simulink model "kinovaMicoSimscapeModel"  (R2021b)
(part 36 of 50)

Y1_10_7=(7*3^(1/2)*dq6*dqr2*cos(q2)*cos(q3)*sin(q6))/4000 + (29*3^(1/2)*dq1*dqr2*sin(2*q2)*cos(q3)*cos(q6))/400 + dq1*dqr2*cos(2*q2)*sin(2*q3)*cos(q6)*((6847*3^(1/2))/160000 - 481/32000) - dq1*dqr2*cos(2*q3)*sin(2*q2)*cos(q6)*((6847*3^(1/2))/160000 - 481/32000) - (333*dq1*dqr2*cos(2*q2)*cos(2*q5)*sin(2*q3)*cos(q6))/32000 + (333*dq1*dqr2*cos(2*q3)*cos(2*q5)*sin(2*q2)*cos(q6))/32000 + (21*dq2*dqr3*cos(q6)*sin(q2)*sin(q3)*sin(q4))/4000 - (21*dq3*dqr3*cos(q6)*sin(q2)*sin(q3)*sin(q4))/4000 + (333*dq1*dqr2*cos(2*q2)*sin(2*q3)*sin(2*q5)*sin(q6))/16000 - (333*dq1*dqr2*cos(2*q3)*sin(2*q2)*sin(2*q5)*sin(q6))/16000 + dq2*dqr2*sin(2*q4)*cos(q2)*cos(q3)*cos(q6)*((1923*3^(1/2))/80000 + 111/3200) - dq3*dqr2*sin(2*q4)*cos(q2)*cos(q3)*cos(q6)*((1923*3^(1/2))/80000 + 111/3200) - (37*3^(1/2)*dq5*dqr3*cos(q6)*sin(q2)*sin(q3)*sin(q4))/4000 + (7*3^(1/2)*dq5*dqr3*cos(q6)*sin(q2)*sin(q3)*sin(q5))/4000 - (37*3^(1/2)*dq6*dqr3*cos(q6)*sin(q2)*sin(q3)*sin(q4))/4000 + (7*3^(1/2)*dq6*dqr3*cos(q6)*sin(q2)*sin(q3)*sin(q5))/2000 + (877*dq1*dqr2*cos(2*q2)*cos(2*q3)*cos(q4)*cos(q5)*sin(q6))/4000 - (37*dq2*dqr2*cos(2*q4)*cos(2*q5)*cos(q2)*cos(q3)*sin(q6))/2000 - (37*dq2*dqr2*cos(2*q4)*sin(2*q5)*cos(q2)*cos(q3)*cos(q6))/4000 - (37*dq2*dqr2*cos(2*q5)*sin(2*q4)*cos(q2)*cos(q3)*cos(q6))/3200 + (37*dq3*dqr2*cos(2*q4)*cos(2*q5)*cos(q2)*cos(q3)*sin(q6))/2000 + (37*dq3*dqr2*cos(2*q4)*sin(2*q5)*cos(q2)*cos(q3)*cos(q6))/4000 + (37*dq3*dqr2*cos(2*q5)*sin(2*q4)*cos(q2)*cos(q3)*cos(q6))/3200 + (877*dq1*dqr2*sin(2*q2)*sin(2*q3)*cos(q4)*cos(q5)*sin(q6))/4000 + (37*dq2*dqr2*sin(2*q4)*sin(2*q5)*cos(q2)*cos(q3)*sin(q6))/1600 - (37*dq3*dqr2*sin(2*q4)*sin(2*q5)*cos(q2)*cos(q3)*sin(q6))/1600 - (29*3^(1/2)*dq1*dqr2*sin(2*q2)*cos(q3)*cos(q5)*cos(q6))/400 - (7*dq2*dqr2*cos(q2)*cos(q3)*cos(q4)*cos(q5)*sin(q6))/1000 - (7*dq2*dqr2*cos(q2)*cos(q3)*cos(q4)*cos(q6)*sin(q5))/2000 + (7*dq3*dqr2*cos(q2)*cos(q3)*cos(q4)*cos(q5)*sin(q6))/1000 + (7*dq3*dqr2*cos(q2)*cos(q3)*cos(q4)*cos(q6)*sin(q5))/2000 - dq1*dqr2*cos(2*q2)*sin(2*q3)*cos(q5)*cos(q6)*((9411*3^(1/2))/160000 - 259/16000) + dq1*dqr2*cos(2*q3)*sin(2*q2)*cos(q5)*cos(q6)*((9411*3^(1/2))/160000 - 259/16000) + (29*3^(1/2)*dq1*dqr2*sin(2*q2)*cos(q3)*sin(q5)*sin(q6))/200 + (7*dq2*dqr3*cos(q4)*cos(q5)*sin(q2)*sin(q3)*sin(q6))/1000 + (7*dq2*dqr3*cos(q4)*cos(q6)*sin(q2)*sin(q3)*sin(q5))/2000 + (7*dq2*dqr3*cos(q5)*cos(q6)*sin(q2)*sin(q3)*sin(q4))/4000 - (7*dq3*dqr3*cos(q4)*cos(q5)*sin(q2)*sin(q3)*sin(q6))/1000 - (7*dq3*dqr3*cos(q4)*cos(q6)*sin(q2)*sin(q3)*sin(q5))/2000 - (7*dq3*dqr3*cos(q5)*cos(q6)*sin(q2)*sin(q3)*sin(q4))/4000 + dq1*dqr2*cos(2*q2)*sin(2*q3)*sin(q5)*sin(q6)*((9411*3^(1/2))/80000 + 37/4000) - dq1*dqr2*cos(2*q3)*sin(2*q2)*sin(q5)*sin(q6)*((9411*3^(1/2))/80000 + 37/4000) - (7*dq2*dqr3*sin(q2)*sin(q3)*sin(q4)*sin(q5)*sin(q6))/2000 + (7*dq3*dqr3*sin(q2)*sin(q3)*sin(q4)*sin(q5)*sin(q6))/2000 - dq6*dqr2*cos(q2)*cos(q3)*cos(q4)*sin(q6)*((37*3^(1/2))/3200 + 1923/80000) - (29*dq1*dqr2*cos(2*q2)*cos(q3)*cos(q4)*cos(q5)*sin(q6))/100 - (29*dq1*dqr2*cos(2*q2)*cos(q3)*cos(q4)*cos(q6)*sin(q5))/200 + dq1*dqr2*cos(2*q2)*cos(2*q4)*sin(2*q3)*cos(q6)*((1923*3^(1/2))/160000 + 111/6400) - dq1*dqr2*cos(2*q3)*cos(2*q4)*sin(2*q2)*cos(q6)*((1923*3^(1/2))/160000 + 111/6400) - (37*dq1*dqr2*cos(2*q2)*cos(2*q4)*cos(2*q5)*sin(2*q3)*cos(q6))/6400 + (37*dq1*dqr2*cos(2*q3)*cos(2*q4)*cos(2*q5)*sin(2*q2)*cos(q6))/6400 - (7*3^(1/2)*dq5*dqr2*cos(q2)*cos(q3)*cos(q5)*sin(q6))/2000 - (7*3^(1/2)*dq5*dqr2*cos(q2)*cos(q3)*cos(q6)*sin(q5))/4000 - (7*3^(1/2)*dq6*dqr2*cos(q2)*cos(q3)*cos(q5)*sin(q6))/4000 - (7*3^(1/2)*dq6*dqr2*cos(q2)*cos(q3)*cos(q6)*sin(q5))/2000 + (37*dq1*dqr2*cos(2*q2)*cos(2*q4)*sin(2*q3)*sin(2*q5)*sin(q6))/3200 + (37*dq1*dqr2*cos(2*q2)*cos(2*q5)*sin(2*q3)*sin(2*q4)*sin(q6))/4000 + (37*dq1*dqr2*cos(2*q2)*sin(2*q3)*sin(2*q4)*sin(2*q5)*cos(q6))/8000 - (37*dq1*dqr2*cos(2*q3)*cos(2*q4)*sin(2*q2)*sin(2*q5)*sin(q6))/3200 - (37*dq1*dqr2*cos(2*q3)*cos(2*q5)*sin(2*q2)*sin(2*q4)*sin(q6))/4000 - (37*dq1*dqr2*cos(2*q3)*sin(2*q2)*sin(2*q4)*sin(2*q5)*cos(q6))/8000 + dq2*dqr3*sin(2*q4)*sin(q2)*sin(q3)*sin(q5)*sin(q6)*((641*3^(1/2))/40000 + 37/2000) - dq3*dqr3*sin(2*q4)*sin(q2)*sin(q3)*sin(q5)*sin(q6)*((641*3^(1/2))/40000 + 37/2000) - (37*3^(1/2)*dq5*dqr2*cos(2*q5)*cos(q2)*cos(q3)*cos(q4)*sin(q6))/4000 - (37*3^(1/2)*dq5*dqr2*sin(2*q5)*cos(q2)*cos(q3)*cos(q4)*cos(q6))/8000 - (37*3^(1/2)*dq6*dqr2*cos(2*q5)*cos(q2)*cos(q3)*cos(q4)*sin(q6))/16000 - (37*3^(1/2)*dq6*dqr2*sin(2*q5)*cos(q2)*cos(q3)*cos(q4)*cos(q6))/8000 - dq1*dqr2*cos(2*q2)*cos(2*q3)*cos(q4)*cos(q6)*sin(q5)*((37*3^(1/2))/4000 - 877/8000) + (37*3^(1/2)*dq5*dqr3*cos(2*q5)*cos(q6)*sin(q2)*sin(q3)*sin(q4))/4000 + (37*3^(1/2)*dq6*dqr3*cos(2*q5)*cos(q6)*sin(q2)*sin(q3)*sin(q4))/4000 - dq1*dqr2*sin(2*q2)*sin(2*q3)*cos(q4)*cos(q6)*sin(q5)*((37*3^(1/2))/4000 - 877/8000) - (37*3^(1/2)*dq5*dqr3*sin(2*q5)*sin(q2)*sin(q3)*sin(q4)*sin(q6))/2000 - (37*3^(1/2)*dq6*dqr3*sin(2*q5)*sin(q2)*sin(q3)*sin(q4)*sin(q6))/8000 + dq5*dqr2*cos(q2)*cos(q3)*cos(q4)*cos(q5)*sin(q6)*((37*3^(1/2))/2000 + 1923/40000) + dq6*dqr2*cos(q2)*cos(q3)*cos(q4)*cos(q6)*sin(q5)*((37*3^(1/2))/2000 + 1923/40000) - dq5*dqr2*cos(q2)*cos(q3)*cos(q4)*cos(q6)*sin(q5)*((37*3^(1/2))/8000 - 1923/80000) + dq6*dqr2*cos(q2)*cos(q3)*cos(q4)*cos(q5)*sin(q6)*((111*3^(1/2))/8000 + 1923/80000) + dq1*dqr2*cos(2*q2)*cos(2*q4)*sin(2*q3)*cos(q5)*cos(q6)*((641*3^(1/2))/160000 - 37/16000) - dq1*dqr2*cos(2*q3)*cos(2*q4)*sin(2*q2)*cos(q5)*cos(q6)*((641*3^(1/2))/160000 - 37/16000) - dq6*dqr3*cos(q4)*cos(q6)*sin(q2)*sin(q3)*sin(q5)*((37*3^(1/2))/2000 + 1923/40000) + dq5*dqr3*cos(q4)*cos(q6)*sin(q2)*sin(q3)*sin(q5)*((37*3^(1/2))/8000 - 1923/80000) - dq1*dqr2*cos(2*q2)*sin(2*q3)*sin(2*q4)*cos(q5)*sin(q6)*((641*3^(1/2))/40000 + 37/2000) + dq1*dqr2*cos(2*q3)*sin(2*q2)*sin(2*q4)*cos(q5)*sin(q6)*((641*3^(1/2))/40000 + 37/2000) - dq1*dqr2*cos(2*q2)*cos(2*q4)*sin(2*q3)*sin(q5)*sin(q6)*((641*3^(1/2))/80000 + 37/4000) + dq1*dqr2*cos(2*q3)*cos(2*q4)*sin(2*q2)*sin(q5)*sin(q6)*((641*3^(1/2))/80000 + 37/4000) - dq1*dqr2*cos(2*q2)*sin(2*q3)*sin(2*q4)*cos(q6)*sin(q5)*((641*3^(1/2))/80000 - 37/8000) + dq1*dqr2*cos(2*q3)*sin(2*q2)*sin(2*q4)*cos(q6)*sin(q5)*((641*3^(1/2))/80000 - 37/8000) + (37*3^(1/2)*dq1*dqr2*cos(2*q2)*cos(2*q3)*cos(2*q5)*cos(q4)*sin(q6))/2000 + (37*3^(1/2)*dq1*dqr2*cos(2*q2)*cos(2*q3)*sin(2*q5)*cos(q4)*cos(q6))/4000 + dq2*dqr2*cos(2*q4)*cos(q2)*cos(q3)*cos(q5)*sin(q6)*((641*3^(1/2))/20000 + 37/1000) - dq3*dqr2*cos(2*q4)*cos(q2)*cos(q3)*cos(q5)*sin(q6)*((641*3^(1/2))/20000 + 37/1000) + dq2*dqr2*cos(2*q4)*cos(q2)*cos(q3)*cos(q6)*sin(q5)*((641*3^(1/2))/40000 - 37/4000) - dq3*dqr2*cos(2*q4)*cos(q2)*cos(q3)*cos(q6)*sin(q5)*((641*3^(1/2))/40000 - 37/4000) + dq2*dqr2*sin(2*q4)*cos(q2)*cos(q3)*cos(q5)*cos(q6)*((641*3^(1/2))/80000 - 37/8000) - dq3*dqr2*sin(2*q4)*cos(q2)*cos(q3)*cos(q5)*cos(q6)*((641*3^(1/2))/80000 - 37/8000) + (37*3^(1/2)*dq1*dqr2*cos(2*q5)*sin(2*q2)*sin(2*q3)*cos(q4)*sin(q6))/2000 + (37*3^(1/2)*dq1*dqr2*sin(2*q2)*sin(2*q3)*sin(2*q5)*cos(q4)*cos(q6))/4000 - dq2*dqr3*cos(2*q4)*cos(q6)*sin(q2)*sin(q3)*sin(q5)*((641*3^(1/2))/40000 - 37/4000) + dq3*dqr3*cos(2*q4)*cos(q6)*sin(q2)*sin(q3)*sin(q5)*((641*3^(1/2))/40000 - 37/4000) + (37*3^(1/2)*dq6*dqr3*sin(q2)*sin(q3)*sin(q4)*sin(q5)*sin(q6))/4000;
Y1_10_8=(37*dq5*dqr3*cos(q3)*cos(q6)*sin(q2))/4000 + (37*dq6*dqr3*cos(q3)*cos(q6)*sin(q2))/4000 + (111*dq4*dqr3*sin(2*q5)*cos(q3)*sin(q2)*sin(q6))/8000 - (7*3^(1/2)*dq2*dqr3*cos(q3)*cos(q6)*sin(q2))/4000 + (7*3^(1/2)*dq3*dqr3*cos(q3)*cos(q6)*sin(q2))/4000 - (7*3^(1/2)*dq6*dqr3*sin(q2)*sin(q3)*sin(q6))/4000 + (21*dq4*dqr3*cos(q3)*cos(q4)*cos(q6)*sin(q2))/4000 - (21*dq6*dqr3*cos(q3)*sin(q2)*sin(q4)*sin(q6))/4000 - dq4*dqr3*cos(q3)*cos(q6)*sin(q2)*((1923*3^(1/2))/80000 + 259/16000) - (111*dq4*dqr3*cos(2*q5)*cos(q3)*cos(q6)*sin(q2))/16000 - dq4*dqr3*cos(2*q4)*cos(q3)*cos(q6)*sin(q2)*((1923*3^(1/2))/80000 + 111/3200) - (7*3^(1/2)*dq2*dqr3*cos(q3)*sin(q2)*sin(q5)*sin(q6))/2000 + (7*3^(1/2)*dq3*dqr3*cos(q3)*sin(q2)*sin(q5)*sin(q6))/2000 + (7*3^(1/2)*dq5*dqr3*cos(q5)*sin(q2)*sin(q3)*sin(q6))/2000 + (7*3^(1/2)*dq6*dqr3*cos(q5)*sin(q2)*sin(q3)*sin(q6))/4000 + (37*dq4*dqr3*cos(2*q4)*cos(2*q5)*cos(q3)*cos(q6)*sin(q2))/3200 + (37*dq5*dqr3*cos(2*q4)*cos(2*q5)*cos(q3)*cos(q6)*sin(q2))/4000 + (37*dq6*dqr3*cos(2*q4)*cos(2*q5)*cos(q3)*cos(q6)*sin(q2))/4000 - dq2*dqr3*sin(2*q4)*cos(q6)*sin(q2)*sin(q3)*((1923*3^(1/2))/80000 + 111/3200) + dq3*dqr3*sin(2*q4)*cos(q6)*sin(q2)*sin(q3)*((1923*3^(1/2))/80000 + 111/3200) + dq6*dqr3*sin(2*q4)*cos(q3)*sin(q2)*sin(q6)*((1923*3^(1/2))/160000 + 111/6400) + (37*dq2*dqr3*cos(2*q4)*cos(2*q5)*sin(q2)*sin(q3)*sin(q6))/2000 + (37*dq2*dqr3*cos(2*q4)*sin(2*q5)*cos(q6)*sin(q2)*sin(q3))/4000 + (37*dq2*dqr3*cos(2*q5)*sin(2*q4)*cos(q6)*sin(q2)*sin(q3))/3200 - (37*dq3*dqr3*cos(2*q4)*cos(2*q5)*sin(q2)*sin(q3)*sin(q6))/2000 - (37*dq3*dqr3*cos(2*q4)*sin(2*q5)*cos(q6)*sin(q2)*sin(q3))/4000 - (37*dq3*dqr3*cos(2*q5)*sin(2*q4)*cos(q6)*sin(q2)*sin(q3))/3200 - (37*dq4*dqr3*cos(2*q4)*sin(2*q5)*cos(q3)*sin(q2)*sin(q6))/1600 - (37*dq4*dqr3*cos(2*q5)*sin(2*q4)*cos(q3)*sin(q2)*sin(q6))/2000 - (37*dq4*dqr3*sin(2*q4)*sin(2*q5)*cos(q3)*cos(q6)*sin(q2))/4000 - (37*dq5*dqr3*cos(2*q4)*sin(2*q5)*cos(q3)*sin(q2)*sin(q6))/2000 - (37*dq5*dqr3*cos(2*q5)*sin(2*q4)*cos(q3)*sin(q2)*sin(q6))/1600 - (37*dq5*dqr3*sin(2*q4)*sin(2*q5)*cos(q3)*cos(q6)*sin(q2))/3200 - (37*dq6*dqr3*cos(2*q4)*sin(2*q5)*cos(q3)*sin(q2)*sin(q6))/8000 - (37*dq6*dqr3*cos(2*q5)*sin(2*q4)*cos(q3)*sin(q2)*sin(q6))/6400 - (37*dq6*dqr3*sin(2*q4)*sin(2*q5)*cos(q3)*cos(q6)*sin(q2))/3200 - (37*dq2*dqr3*sin(2*q4)*sin(2*q5)*sin(q2)*sin(q3)*sin(q6))/1600 + (37*dq3*dqr3*sin(2*q4)*sin(2*q5)*sin(q2)*sin(q3)*sin(q6))/1600 + (1231*dq2*dqr3*cos(q3)*cos(q4)*cos(q5)*cos(q6)*sin(q2))/40000 - (1231*dq3*dqr3*cos(q3)*cos(q4)*cos(q5)*cos(q6)*sin(q2))/40000 + (7*dq4*dqr3*cos(q3)*cos(q4)*cos(q5)*cos(q6)*sin(q2))/4000 + (7*dq5*dqr3*cos(q3)*cos(q4)*cos(q5)*cos(q6)*sin(q2))/2000 + (7*dq6*dqr3*cos(q3)*cos(q4)*cos(q5)*cos(q6)*sin(q2))/1000 - (877*dq2*dqr3*cos(q3)*cos(q5)*sin(q2)*sin(q4)*sin(q6))/4000 + (877*dq3*dqr3*cos(q3)*cos(q5)*sin(q2)*sin(q4)*sin(q6))/4000 - (7*dq4*dqr3*cos(q3)*cos(q4)*sin(q2)*sin(q5)*sin(q6))/2000 - (7*dq4*dqr3*cos(q3)*cos(q5)*sin(q2)*sin(q4)*sin(q6))/1000 - (7*dq4*dqr3*cos(q3)*cos(q6)*sin(q2)*sin(q4)*sin(q5))/2000 - (7*dq5*dqr3*cos(q3)*cos(q4)*sin(q2)*sin(q5)*sin(q6))/1000 - (7*dq5*dqr3*cos(q3)*cos(q5)*sin(q2)*sin(q4)*sin(q6))/2000 - (7*dq5*dqr3*cos(q3)*cos(q6)*sin(q2)*sin(q4)*sin(q5))/4000 - (7*dq6*dqr3*cos(q3)*cos(q4)*sin(q2)*sin(q5)*sin(q6))/2000 - (7*dq6*dqr3*cos(q3)*cos(q5)*sin(q2)*sin(q4)*sin(q6))/4000 - (7*dq6*dqr3*cos(q3)*cos(q6)*sin(q2)*sin(q4)*sin(q5))/2000 - dq6*dqr3*cos(q3)*cos(q5)*cos(q6)*sin(q2)*((641*3^(1/2))/40000 + 37/2000) + dq2*dqr3*cos(q3)*cos(q4)*cos(q6)*sin(q2)*((111*3^(1/2))/8000 + 7539/40000) - dq3*dqr3*cos(q3)*cos(q4)*cos(q6)*sin(q2)*((111*3^(1/2))/8000 + 7539/40000) - dq4*dqr3*cos(q3)*cos(q5)*cos(q6)*sin(q2)*((641*3^(1/2))/80000 - 37/8000) - dq5*dqr3*cos(q3)*cos(q5)*cos(q6)*sin(q2)*((641*3^(1/2))/80000 - 37/8000) + dq4*dqr3*cos(q3)*sin(q2)*sin(q5)*sin(q6)*((641*3^(1/2))/40000 + 37/2000) + dq5*dqr3*cos(q3)*sin(q2)*sin(q5)*sin(q6)*((641*3^(1/2))/40000 + 37/2000) + dq6*dqr3*cos(q3)*sin(q2)*sin(q5)*sin(q6)*((641*3^(1/2))/80000 + 37/1600) + dq6*dqr3*cos(q4)*sin(q2)*sin(q3)*sin(q6)*((37*3^(1/2))/3200 + 1923/80000) + (7*3^(1/2)*dq2*dqr3*cos(q3)*cos(q5)*cos(q6)*sin(q2))/4000 - (7*3^(1/2)*dq3*dqr3*cos(q3)*cos(q5)*cos(q6)*sin(q2))/4000 - (29*dq1*dqr3*sin(2*q2)*sin(q3)*sin(q4)*sin(q5)*sin(q6))/400 + (37*3^(1/2)*dq2*dqr3*cos(2*q5)*cos(q3)*cos(q4)*cos(q6)*sin(q2))/8000 - (37*3^(1/2)*dq3*dqr3*cos(2*q5)*cos(q3)*cos(q4)*cos(q6)*sin(q2))/8000 - (37*3^(1/2)*dq2*dqr3*cos(2*q5)*cos(q3)*sin(q2)*sin(q4)*sin(q6))/2000 - (37*3^(1/2)*dq2*dqr3*sin(2*q5)*cos(q3)*cos(q4)*sin(q2)*sin(q6))/4000 - (37*3^(1/2)*dq2*dqr3*sin(2*q5)*cos(q3)*cos(q6)*sin(q2)*sin(q4))/4000 + (37*3^(1/2)*dq3*dqr3*cos(2*q5)*cos(q3)*sin(q2)*sin(q4)*sin(q6))/2000 + (37*3^(1/2)*dq3*dqr3*sin(2*q5)*cos(q3)*cos(q4)*sin(q2)*sin(q6))/4000 + (37*3^(1/2)*dq3*dqr3*sin(2*q5)*cos(q3)*cos(q6)*sin(q2)*sin(q4))/4000 + (37*3^(1/2)*dq5*dqr3*cos(2*q5)*cos(q4)*sin(q2)*sin(q3)*sin(q6))/4000 + (37*3^(1/2)*dq5*dqr3*sin(2*q5)*cos(q4)*cos(q6)*sin(q2)*sin(q3))/8000 + (37*3^(1/2)*dq6*dqr3*cos(2*q5)*cos(q4)*sin(q2)*sin(q3)*sin(q6))/16000 + (37*3^(1/2)*dq6*dqr3*sin(2*q5)*cos(q4)*cos(q6)*sin(q2)*sin(q3))/8000 + dq2*dqr3*cos(q3)*cos(q6)*sin(q2)*sin(q4)*sin(q5)*((37*3^(1/2))/4000 - 877/8000) - dq3*dqr3*cos(q3)*cos(q6)*sin(q2)*sin(q4)*sin(q5)*((37*3^(1/2))/4000 - 877/8000) + dq2*dqr3*cos(q3)*cos(q4)*sin(q2)*sin(q5)*sin(q6)*((37*3^(1/2))/2000 - 1231/20000) - dq3*dqr3*cos(q3)*cos(q4)*sin(q2)*sin(q5)*sin(q6)*((37*3^(1/2))/2000 - 1231/20000) - dq5*dqr3*cos(q4)*cos(q5)*sin(q2)*sin(q3)*sin(q6)*((37*3^(1/2))/2000 + 1923/40000) - dq6*dqr3*cos(q4)*cos(q5)*sin(q2)*sin(q3)*sin(q6)*((111*3^(1/2))/8000 + 1923/80000) - dq6*dqr3*cos(2*q4)*cos(q3)*cos(q5)*cos(q6)*sin(q2)*((641*3^(1/2))/40000 + 37/2000) - dq4*dqr3*cos(2*q4)*cos(q3)*cos(q5)*cos(q6)*sin(q2)*((641*3^(1/2))/80000 - 37/8000) - dq5*dqr3*cos(2*q4)*cos(q3)*cos(q5)*cos(q6)*sin(q2)*((641*3^(1/2))/80000 - 37/8000) - dq2*dqr3*cos(2*q4)*cos(q5)*sin(q2)*sin(q3)*sin(q6)*((641*3^(1/2))/20000 + 37/1000) + dq3*dqr3*cos(2*q4)*cos(q5)*sin(q2)*sin(q3)*sin(q6)*((641*3^(1/2))/20000 + 37/1000) + dq4*dqr3*sin(2*q4)*cos(q3)*cos(q5)*sin(q2)*sin(q6)*((641*3^(1/2))/20000 + 37/1000) + dq4*dqr3*cos(2*q4)*cos(q3)*sin(q2)*sin(q5)*sin(q6)*((641*3^(1/2))/40000 + 37/2000) + dq5*dqr3*cos(2*q4)*cos(q3)*sin(q2)*sin(q5)*sin(q6)*((641*3^(1/2))/40000 + 37/2000) + dq4*dqr3*sin(2*q4)*cos(q3)*cos(q6)*sin(q2)*sin(q5)*((641*3^(1/2))/40000 - 37/4000) + dq5*dqr3*sin(2*q4)*cos(q3)*cos(q5)*sin(q2)*sin(q6)*((641*3^(1/2))/80000 + 37/4000) + dq6*dqr3*sin(2*q4)*cos(q3)*cos(q6)*sin(q2)*sin(q5)*((641*3^(1/2))/80000 + 37/4000) - dq2*dqr3*sin(2*q4)*cos(q5)*cos(q6)*sin(q2)*sin(q3)*((641*3^(1/2))/80000 - 37/8000) + dq3*dqr3*sin(2*q4)*cos(q5)*cos(q6)*sin(q2)*sin(q3)*((641*3^(1/2))/80000 - 37/8000) + dq6*dqr3*cos(2*q4)*cos(q3)*sin(q2)*sin(q5)*sin(q6)*((641*3^(1/2))/80000 - 37/8000) + dq5*dqr3*sin(2*q4)*cos(q3)*cos(q6)*sin(q2)*sin(q5)*((641*3^(1/2))/160000 - 37/16000) + dq6*dqr3*sin(2*q4)*cos(q3)*cos(q5)*sin(q2)*sin(q6)*((641*3^(1/2))/160000 - 37/16000);
Y1_10_9=(87*dq1*dqr3*sin(2*q2)*cos(q6)*sin(q3)*sin(q4))/800 - (37*dq5*dqr3*cos(q2)*cos(q6)*sin(q3))/4000 - (37*dq6*dqr3*cos(q2)*cos(q6)*sin(q3))/4000 - (29*3^(1/2)*dq1*dqr3*cos(q6)*sin(q3))/800 - (111*dq4*dqr3*sin(2*q5)*cos(q2)*sin(q3)*sin(q6))/8000 + (7*3^(1/2)*dq2*dqr3*cos(q2)*cos(q6)*sin(q3))/4000 - (7*3^(1/2)*dq3*dqr3*cos(q2)*cos(q6)*sin(q3))/4000 + (29*3^(1/2)*dq1*dqr3*cos(q5)*cos(q6)*sin(q3))/800 - (29*3^(1/2)*dq1*dqr3*sin(q3)*sin(q5)*sin(q6))/400 + (29*3^(1/2)*dq1*dqr3*cos(2*q2)*cos(q6)*sin(q3))/800 + (21*dq2*dqr3*cos(q2)*cos(q3)*cos(q6)*sin(q4))/4000 - (21*dq3*dqr3*cos(q2)*cos(q3)*cos(q6)*sin(q4))/4000 - (21*dq4*dqr3*cos(q2)*cos(q4)*cos(q6)*sin(q3))/4000 + (29*dq1*dqr3*cos(q3)*sin(q4)*sin(q5)*sin(q6))/400 + (21*dq6*dqr3*cos(q2)*sin(q3)*sin(q4)*sin(q6))/4000 + dq4*dqr3*cos(q2)*cos(q6)*sin(q3)*((1923*3^(1/2))/80000 + 259/16000) + (111*dq4*dqr3*cos(2*q5)*cos(q2)*cos(q6)*sin(q3))/16000 + dq4*dqr3*cos(2*q4)*cos(q2)*cos(q6)*sin(q3)*((1923*3^(1/2))/80000 + 111/3200) + (7*3^(1/2)*dq2*dqr3*cos(q2)*sin(q3)*sin(q5)*sin(q6))/2000 - (7*3^(1/2)*dq3*dqr3*cos(q2)*sin(q3)*sin(q5)*sin(q6))/2000 - (37*dq4*dqr3*cos(2*q4)*cos(2*q5)*cos(q2)*cos(q6)*sin(q3))/3200 - (37*dq5*dqr3*cos(2*q4)*cos(2*q5)*cos(q2)*cos(q6)*sin(q3))/4000 - (37*dq6*dqr3*cos(2*q4)*cos(2*q5)*cos(q2)*cos(q6)*sin(q3))/4000 - dq6*dqr3*sin(2*q4)*cos(q2)*sin(q3)*sin(q6)*((1923*3^(1/2))/160000 + 111/6400) + (37*dq4*dqr3*cos(2*q4)*sin(2*q5)*cos(q2)*sin(q3)*sin(q6))/1600 + (37*dq4*dqr3*cos(2*q5)*sin(2*q4)*cos(q2)*sin(q3)*sin(q6))/2000 + (37*dq4*dqr3*sin(2*q4)*sin(2*q5)*cos(q2)*cos(q6)*sin(q3))/4000 + (37*dq5*dqr3*cos(2*q4)*sin(2*q5)*cos(q2)*sin(q3)*sin(q6))/2000 + (37*dq5*dqr3*cos(2*q5)*sin(2*q4)*cos(q2)*sin(q3)*sin(q6))/1600 + (37*dq5*dqr3*sin(2*q4)*sin(2*q5)*cos(q2)*cos(q6)*sin(q3))/3200 + (37*dq6*dqr3*cos(2*q4)*sin(2*q5)*cos(q2)*sin(q3)*sin(q6))/8000 + (37*dq6*dqr3*cos(2*q5)*sin(2*q4)*cos(q2)*sin(q3)*sin(q6))/6400 + (37*dq6*dqr3*sin(2*q4)*sin(2*q5)*cos(q2)*cos(q6)*sin(q3))/3200 - (29*3^(1/2)*dq1*dqr3*cos(2*q2)*cos(q5)*cos(q6)*sin(q3))/800 + (7*dq2*dqr3*cos(q2)*cos(q3)*cos(q5)*cos(q6)*sin(q4))/4000 - (1231*dq2*dqr3*cos(q2)*cos(q4)*cos(q5)*cos(q6)*sin(q3))/40000 - (7*dq3*dqr3*cos(q2)*cos(q3)*cos(q5)*cos(q6)*sin(q4))/4000 + (1231*dq3*dqr3*cos(q2)*cos(q4)*cos(q5)*cos(q6)*sin(q3))/40000 - (7*dq4*dqr3*cos(q2)*cos(q4)*cos(q5)*cos(q6)*sin(q3))/4000 - (7*dq5*dqr3*cos(q2)*cos(q4)*cos(q5)*cos(q6)*sin(q3))/2000 - (7*dq6*dqr3*cos(q2)*cos(q4)*cos(q5)*cos(q6)*sin(q3))/1000 + (29*3^(1/2)*dq1*dqr3*cos(2*q2)*sin(q3)*sin(q5)*sin(q6))/400 - (7*dq2*dqr3*cos(q2)*cos(q3)*sin(q4)*sin(q5)*sin(q6))/2000 + (877*dq2*dqr3*cos(q2)*cos(q5)*sin(q3)*sin(q4)*sin(q6))/4000 + (7*dq3*dqr3*cos(q2)*cos(q3)*sin(q4)*sin(q5)*sin(q6))/2000 - (877*dq3*dqr3*cos(q2)*cos(q5)*sin(q3)*sin(q4)*sin(q6))/4000 + (7*dq4*dqr3*cos(q2)*cos(q4)*sin(q3)*sin(q5)*sin(q6))/2000 + (7*dq4*dqr3*cos(q2)*cos(q5)*sin(q3)*sin(q4)*sin(q6))/1000 + (7*dq4*dqr3*cos(q2)*cos(q6)*sin(q3)*sin(q4)*sin(q5))/2000 + (7*dq5*dqr3*cos(q2)*cos(q4)*sin(q3)*sin(q5)*sin(q6))/1000 + (7*dq5*dqr3*cos(q2)*cos(q5)*sin(q3)*sin(q4)*sin(q6))/2000 + (7*dq5*dqr3*cos(q2)*cos(q6)*sin(q3)*sin(q4)*sin(q5))/4000 + (7*dq6*dqr3*cos(q2)*cos(q4)*sin(q3)*sin(q5)*sin(q6))/2000 + (7*dq6*dqr3*cos(q2)*cos(q5)*sin(q3)*sin(q4)*sin(q6))/4000 + (7*dq6*dqr3*cos(q2)*cos(q6)*sin(q3)*sin(q4)*sin(q5))/2000 + dq6*dqr3*cos(q2)*cos(q5)*cos(q6)*sin(q3)*((641*3^(1/2))/40000 + 37/2000) - dq2*dqr3*cos(q2)*cos(q4)*cos(q6)*sin(q3)*((111*3^(1/2))/8000 + 7539/40000) + dq3*dqr3*cos(q2)*cos(q4)*cos(q6)*sin(q3)*((111*3^(1/2))/8000 + 7539/40000) + dq4*dqr3*cos(q2)*cos(q5)*cos(q6)*sin(q3)*((641*3^(1/2))/80000 - 37/8000) + dq5*dqr3*cos(q2)*cos(q5)*cos(q6)*sin(q3)*((641*3^(1/2))/80000 - 37/8000) - dq4*dqr3*cos(q2)*sin(q3)*sin(q5)*sin(q6)*((641*3^(1/2))/40000 + 37/2000) - dq5*dqr3*cos(q2)*sin(q3)*sin(q5)*sin(q6)*((641*3^(1/2))/40000 + 37/2000) - dq6*dqr3*cos(q2)*sin(q3)*sin(q5)*sin(q6)*((641*3^(1/2))/80000 + 37/1600) - (29*dq1*dqr3*cos(2*q2)*cos(q3)*sin(q4)*sin(q5)*sin(q6))/400 + (29*dq1*dqr3*sin(2*q2)*cos(q4)*cos(q5)*sin(q3)*sin(q6))/200 + (29*dq1*dqr3*sin(2*q2)*cos(q4)*cos(q6)*sin(q3)*sin(q5))/400 + (29*dq1*dqr3*sin(2*q2)*cos(q5)*cos(q6)*sin(q3)*sin(q4))/800 - (7*3^(1/2)*dq2*dqr3*cos(q2)*cos(q5)*cos(q6)*sin(q3))/4000 + (7*3^(1/2)*dq3*dqr3*cos(q2)*cos(q5)*cos(q6)*sin(q3))/4000 + (37*3^(1/2)*dq1*dqr3*sin(2*q2)*sin(2*q3)*sin(2*q5)*sin(q4)*sin(q6))/4000 - (37*3^(1/2)*dq2*dqr3*cos(2*q5)*cos(q2)*cos(q4)*cos(q6)*sin(q3))/8000 + (37*3^(1/2)*dq3*dqr3*cos(2*q5)*cos(q2)*cos(q4)*cos(q6)*sin(q3))/8000 + (37*3^(1/2)*dq2*dqr3*cos(2*q5)*cos(q2)*sin(q3)*sin(q4)*sin(q6))/2000 + (37*3^(1/2)*dq2*dqr3*sin(2*q5)*cos(q2)*cos(q4)*sin(q3)*sin(q6))/4000 + (37*3^(1/2)*dq2*dqr3*sin(2*q5)*cos(q2)*cos(q6)*sin(q3)*sin(q4))/4000 - (37*3^(1/2)*dq3*dqr3*cos(2*q5)*cos(q2)*sin(q3)*sin(q4)*sin(q6))/2000 - (37*3^(1/2)*dq3*dqr3*sin(2*q5)*cos(q2)*cos(q4)*sin(q3)*sin(q6))/4000 - (37*3^(1/2)*dq3*dqr3*sin(2*q5)*cos(q2)*cos(q6)*sin(q3)*sin(q4))/4000 - (37*3^(1/2)*dq5*dqr3*sin(2*q5)*cos(q2)*cos(q3)*sin(q4)*sin(q6))/2000 - (37*3^(1/2)*dq6*dqr3*sin(2*q5)*cos(q2)*cos(q3)*sin(q4)*sin(q6))/8000 - dq1*dqr3*cos(2*q2)*cos(2*q3)*sin(q4)*sin(q5)*sin(q6)*((37*3^(1/2))/2000 - 1231/20000) - dq1*dqr3*sin(2*q2)*sin(2*q3)*sin(q4)*sin(q5)*sin(q6)*((37*3^(1/2))/2000 - 1231/20000) - dq2*dqr3*cos(q2)*cos(q6)*sin(q3)*sin(q4)*sin(q5)*((37*3^(1/2))/4000 - 877/8000) + dq3*dqr3*cos(q2)*cos(q6)*sin(q3)*sin(q4)*sin(q5)*((37*3^(1/2))/4000 - 877/8000) - dq2*dqr3*cos(q2)*cos(q4)*sin(q3)*sin(q5)*sin(q6)*((37*3^(1/2))/2000 - 1231/20000) + dq3*dqr3*cos(q2)*cos(q4)*sin(q3)*sin(q5)*sin(q6)*((37*3^(1/2))/2000 - 1231/20000) + dq6*dqr3*cos(2*q4)*cos(q2)*cos(q5)*cos(q6)*sin(q3)*((641*3^(1/2))/40000 + 37/2000) + dq4*dqr3*cos(2*q4)*cos(q2)*cos(q5)*cos(q6)*sin(q3)*((641*3^(1/2))/80000 - 37/8000) + dq5*dqr3*cos(2*q4)*cos(q2)*cos(q5)*cos(q6)*sin(q3)*((641*3^(1/2))/80000 - 37/8000) + (37*3^(1/2)*dq6*dqr3*cos(q2)*cos(q3)*sin(q4)*sin(q5)*sin(q6))/4000 + (37*3^(1/2)*dq1*dqr3*cos(2*q2)*cos(2*q3)*sin(2*q5)*sin(q4)*sin(q6))/4000 - dq4*dqr3*sin(2*q4)*cos(q2)*cos(q5)*sin(q3)*sin(q6)*((641*3^(1/2))/20000 + 37/1000) - dq4*dqr3*cos(2*q4)*cos(q2)*sin(q3)*sin(q5)*sin(q6)*((641*3^(1/2))/40000 + 37/2000) - dq5*dqr3*cos(2*q4)*cos(q2)*sin(q3)*sin(q5)*sin(q6)*((641*3^(1/2))/40000 + 37/2000) - dq4*dqr3*sin(2*q4)*cos(q2)*cos(q6)*sin(q3)*sin(q5)*((641*3^(1/2))/40000 - 37/4000) - dq5*dqr3*sin(2*q4)*cos(q2)*cos(q5)*sin(q3)*sin(q6)*((641*3^(1/2))/80000 + 37/4000) - dq6*dqr3*sin(2*q4)*cos(q2)*cos(q6)*sin(q3)*sin(q5)*((641*3^(1/2))/80000 + 37/4000) - dq6*dqr3*cos(2*q4)*cos(q2)*sin(q3)*sin(q5)*sin(q6)*((641*3^(1/2))/80000 - 37/8000) - dq5*dqr3*sin(2*q4)*cos(q2)*cos(q6)*sin(q3)*sin(q5)*((641*3^(1/2))/160000 - 37/16000) - dq6*dqr3*sin(2*q4)*cos(q2)*cos(q5)*sin(q3)*sin(q6)*((641*3^(1/2))/160000 - 37/16000);
Y1_10_10=dq1*dqr3*cos(2*q3)*sin(2*q2)*cos(q6)*((6847*3^(1/2))/160000 - 481/32000) - (7*3^(1/2)*dq6*dqr3*cos(q2)*cos(q3)*sin(q6))/4000 - (29*3^(1/2)*dq1*dqr3*sin(2*q2)*cos(q3)*cos(q6))/800 - (29*dq1*dqr3*cos(q3)*cos(q4)*cos(q5)*sin(q6))/200 - (29*dq1*dqr3*cos(q3)*cos(q4)*cos(q6)*sin(q5))/400 - (29*dq1*dqr3*cos(q3)*cos(q5)*cos(q6)*sin(q4))/800 - dq1*dqr3*cos(2*q2)*sin(2*q3)*cos(q6)*((6847*3^(1/2))/160000 - 481/32000) - (87*dq1*dqr3*cos(q3)*cos(q6)*sin(q4))/800 + (333*dq1*dqr3*cos(2*q2)*cos(2*q5)*sin(2*q3)*cos(q6))/32000 - (333*dq1*dqr3*cos(2*q3)*cos(2*q5)*sin(2*q2)*cos(q6))/32000 - (21*dq4*dqr4*cos(q6)*sin(q2)*sin(q3)*sin(q4))/4000 - (333*dq1*dqr3*cos(2*q2)*sin(2*q3)*sin(2*q5)*sin(q6))/16000 + (333*dq1*dqr3*cos(2*q3)*sin(2*q2)*sin(2*q5)*sin(q6))/16000 + (87*dq1*dqr3*cos(2*q2)*cos(q3)*cos(q6)*sin(q4))/800 - dq2*dqr3*sin(2*q4)*cos(q2)*cos(q3)*cos(q6)*((1923*3^(1/2))/80000 + 111/3200) + dq3*dqr3*sin(2*q4)*cos(q2)*cos(q3)*cos(q6)*((1923*3^(1/2))/80000 + 111/3200) - (877*dq1*dqr3*cos(2*q2)*cos(2*q3)*cos(q4)*cos(q5)*sin(q6))/4000 - (1231*dq1*dqr3*cos(2*q2)*cos(2*q3)*cos(q5)*cos(q6)*sin(q4))/40000 + (37*dq2*dqr3*cos(2*q4)*cos(2*q5)*cos(q2)*cos(q3)*sin(q6))/2000 + (37*dq2*dqr3*cos(2*q4)*sin(2*q5)*cos(q2)*cos(q3)*cos(q6))/4000 + (37*dq2*dqr3*cos(2*q5)*sin(2*q4)*cos(q2)*cos(q3)*cos(q6))/3200 - (37*dq3*dqr3*cos(2*q4)*cos(2*q5)*cos(q2)*cos(q3)*sin(q6))/2000 - (37*dq3*dqr3*cos(2*q4)*sin(2*q5)*cos(q2)*cos(q3)*cos(q6))/4000 - (37*dq3*dqr3*cos(2*q5)*sin(2*q4)*cos(q2)*cos(q3)*cos(q6))/3200 - (877*dq1*dqr3*sin(2*q2)*sin(2*q3)*cos(q4)*cos(q5)*sin(q6))/4000 - (1231*dq1*dqr3*sin(2*q2)*sin(2*q3)*cos(q5)*cos(q6)*sin(q4))/40000 - (37*dq2*dqr3*sin(2*q4)*sin(2*q5)*cos(q2)*cos(q3)*sin(q6))/1600 + (37*dq3*dqr3*sin(2*q4)*sin(2*q5)*cos(q2)*cos(q3)*sin(q6))/1600 + (29*3^(1/2)*dq1*dqr3*sin(2*q2)*cos(q3)*cos(q5)*cos(q6))/800 + (7*dq2*dqr3*cos(q2)*cos(q3)*cos(q4)*cos(q5)*sin(q6))/1000 + (7*dq2*dqr3*cos(q2)*cos(q3)*cos(q4)*cos(q6)*sin(q5))/2000 - (7*dq3*dqr3*cos(q2)*cos(q3)*cos(q4)*cos(q5)*sin(q6))/1000 - (7*dq3*dqr3*cos(q2)*cos(q3)*cos(q4)*cos(q6)*sin(q5))/2000 - dq1*dqr3*cos(2*q2)*cos(2*q3)*cos(q6)*sin(q4)*((111*3^(1/2))/8000 + 7539/40000) + dq1*dqr3*cos(2*q2)*sin(2*q3)*cos(q5)*cos(q6)*((9411*3^(1/2))/160000 - 259/16000) - dq1*dqr3*cos(2*q3)*sin(2*q2)*cos(q5)*cos(q6)*((9411*3^(1/2))/160000 - 259/16000) - (29*3^(1/2)*dq1*dqr3*sin(2*q2)*cos(q3)*sin(q5)*sin(q6))/400 - (7*dq4*dqr4*cos(q5)*cos(q6)*sin(q2)*sin(q3)*sin(q4))/4000 - (7*dq5*dqr4*cos(q5)*cos(q6)*sin(q2)*sin(q3)*sin(q4))/2000 - (7*dq6*dqr4*cos(q5)*cos(q6)*sin(q2)*sin(q3)*sin(q4))/1000 - dq1*dqr3*sin(2*q2)*sin(2*q3)*cos(q6)*sin(q4)*((111*3^(1/2))/8000 + 7539/40000) - dq1*dqr3*cos(2*q2)*sin(2*q3)*sin(q5)*sin(q6)*((9411*3^(1/2))/80000 + 37/4000) + dq1*dqr3*cos(2*q3)*sin(2*q2)*sin(q5)*sin(q6)*((9411*3^(1/2))/80000 + 37/4000) + (7*dq4*dqr4*sin(q2)*sin(q3)*sin(q4)*sin(q5)*sin(q6))/2000 + (7*dq5*dqr4*sin(q2)*sin(q3)*sin(q4)*sin(q5)*sin(q6))/1000 + (7*dq6*dqr4*sin(q2)*sin(q3)*sin(q4)*sin(q5)*sin(q6))/2000 + dq6*dqr3*cos(q2)*cos(q3)*cos(q4)*sin(q6)*((37*3^(1/2))/3200 + 1923/80000) + (29*dq1*dqr3*cos(2*q2)*cos(q3)*cos(q4)*cos(q5)*sin(q6))/200 + (29*dq1*dqr3*cos(2*q2)*cos(q3)*cos(q4)*cos(q6)*sin(q5))/400 + (29*dq1*dqr3*cos(2*q2)*cos(q3)*cos(q5)*cos(q6)*sin(q4))/800 - dq1*dqr3*cos(2*q2)*cos(2*q4)*sin(2*q3)*cos(q6)*((1923*3^(1/2))/160000 + 111/6400) + dq1*dqr3*cos(2*q3)*cos(2*q4)*sin(2*q2)*cos(q6)*((1923*3^(1/2))/160000 + 111/6400) + (37*dq1*dqr3*cos(2*q2)*cos(2*q4)*cos(2*q5)*sin(2*q3)*cos(q6))/6400 - (37*dq1*dqr3*cos(2*q3)*cos(2*q4)*cos(2*q5)*sin(2*q2)*cos(q6))/6400 - (37*3^(1/2)*dq5*dqr3*cos(q2)*cos(q3)*cos(q6)*sin(q4))/4000 + (7*3^(1/2)*dq5*dqr3*cos(q2)*cos(q3)*cos(q5)*sin(q6))/2000 + (7*3^(1/2)*dq5*dqr3*cos(q2)*cos(q3)*cos(q6)*sin(q5))/4000 - (37*3^(1/2)*dq6*dqr3*cos(q2)*cos(q3)*cos(q6)*sin(q4))/4000 + (7*3^(1/2)*dq6*dqr3*cos(q2)*cos(q3)*cos(q5)*sin(q6))/4000 + (7*3^(1/2)*dq6*dqr3*cos(q2)*cos(q3)*cos(q6)*sin(q5))/2000 - (37*dq1*dqr3*cos(2*q2)*cos(2*q4)*sin(2*q3)*sin(2*q5)*sin(q6))/3200 - (37*dq1*dqr3*cos(2*q2)*cos(2*q5)*sin(2*q3)*sin(2*q4)*sin(q6))/4000 - (37*dq1*dqr3*cos(2*q2)*sin(2*q3)*sin(2*q4)*sin(2*q5)*cos(q6))/8000 + (37*dq1*dqr3*cos(2*q3)*cos(2*q4)*sin(2*q2)*sin(2*q5)*sin(q6))/3200 + (37*dq1*dqr3*cos(2*q3)*cos(2*q5)*sin(2*q2)*sin(2*q4)*sin(q6))/4000 + (37*dq1*dqr3*cos(2*q3)*sin(2*q2)*sin(2*q4)*sin(2*q5)*cos(q6))/8000 + (37*3^(1/2)*dq5*dqr3*cos(2*q5)*cos(q2)*cos(q3)*cos(q4)*sin(q6))/4000 + (37*3^(1/2)*dq5*dqr3*cos(2*q5)*cos(q2)*cos(q3)*cos(q6)*sin(q4))/4000 + (37*3^(1/2)*dq5*dqr3*sin(2*q5)*cos(q2)*cos(q3)*cos(q4)*cos(q6))/8000 + (37*3^(1/2)*dq6*dqr3*cos(2*q5)*cos(q2)*cos(q3)*cos(q4)*sin(q6))/16000 + (37*3^(1/2)*dq6*dqr3*cos(2*q5)*cos(q2)*cos(q3)*cos(q6)*sin(q4))/4000 + (37*3^(1/2)*dq6*dqr3*sin(2*q5)*cos(q2)*cos(q3)*cos(q4)*cos(q6))/8000 + dq1*dqr3*cos(2*q2)*cos(2*q3)*cos(q4)*cos(q6)*sin(q5)*((37*3^(1/2))/4000 - 877/8000) + dq1*dqr3*sin(2*q2)*sin(2*q3)*cos(q4)*cos(q6)*sin(q5)*((37*3^(1/2))/4000 - 877/8000) - dq5*dqr3*cos(q2)*cos(q3)*cos(q4)*cos(q5)*sin(q6)*((37*3^(1/2))/2000 + 1923/40000) - dq6*dqr3*cos(q2)*cos(q3)*cos(q4)*cos(q6)*sin(q5)*((37*3^(1/2))/2000 + 1923/40000) + dq5*dqr3*cos(q2)*cos(q3)*cos(q4)*cos(q6)*sin(q5)*((37*3^(1/2))/8000 - 1923/80000) - dq6*dqr3*cos(q2)*cos(q3)*cos(q4)*cos(q5)*sin(q6)*((111*3^(1/2))/8000 + 1923/80000) - dq1*dqr3*cos(2*q2)*cos(2*q4)*sin(2*q3)*cos(q5)*cos(q6)*((641*3^(1/2))/160000 - 37/16000) + dq1*dqr3*cos(2*q3)*cos(2*q4)*sin(2*q2)*cos(q5)*cos(q6)*((641*3^(1/2))/160000 - 37/16000) + dq1*dqr3*cos(2*q2)*sin(2*q3)*sin(2*q4)*cos(q5)*sin(q6)*((641*3^(1/2))/40000 + 37/2000) - dq1*dqr3*cos(2*q3)*sin(2*q2)*sin(2*q4)*cos(q5)*sin(q6)*((641*3^(1/2))/40000 + 37/2000) + dq1*dqr3*cos(2*q2)*cos(2*q4)*sin(2*q3)*sin(q5)*sin(q6)*((641*3^(1/2))/80000 + 37/4000) - dq1*dqr3*cos(2*q3)*cos(2*q4)*sin(2*q2)*sin(q5)*sin(q6)*((641*3^(1/2))/80000 + 37/4000) + dq1*dqr3*cos(2*q2)*sin(2*q3)*sin(2*q4)*cos(q6)*sin(q5)*((641*3^(1/2))/80000 - 37/8000) - dq1*dqr3*cos(2*q3)*sin(2*q2)*sin(2*q4)*cos(q6)*sin(q5)*((641*3^(1/2))/80000 - 37/8000) - (37*3^(1/2)*dq1*dqr3*cos(2*q2)*cos(2*q3)*cos(2*q5)*cos(q4)*sin(q6))/2000 - (37*3^(1/2)*dq1*dqr3*cos(2*q2)*cos(2*q3)*cos(2*q5)*cos(q6)*sin(q4))/8000 - (37*3^(1/2)*dq1*dqr3*cos(2*q2)*cos(2*q3)*sin(2*q5)*cos(q4)*cos(q6))/4000 - dq2*dqr3*cos(2*q4)*cos(q2)*cos(q3)*cos(q5)*sin(q6)*((641*3^(1/2))/20000 + 37/1000) + dq3*dqr3*cos(2*q4)*cos(q2)*cos(q3)*cos(q5)*sin(q6)*((641*3^(1/2))/20000 + 37/1000) - dq2*dqr3*cos(2*q4)*cos(q2)*cos(q3)*cos(q6)*sin(q5)*((641*3^(1/2))/40000 - 37/4000) + dq3*dqr3*cos(2*q4)*cos(q2)*cos(q3)*cos(q6)*sin(q5)*((641*3^(1/2))/40000 - 37/4000) - dq2*dqr3*sin(2*q4)*cos(q2)*cos(q3)*cos(q5)*cos(q6)*((641*3^(1/2))/80000 - 37/8000) + dq3*dqr3*sin(2*q4)*cos(q2)*cos(q3)*cos(q5)*cos(q6)*((641*3^(1/2))/80000 - 37/8000) - (37*3^(1/2)*dq1*dqr3*cos(2*q5)*sin(2*q2)*sin(2*q3)*cos(q4)*sin(q6))/2000 - (37*3^(1/2)*dq1*dqr3*cos(2*q5)*sin(2*q2)*sin(2*q3)*cos(q6)*sin(q4))/8000 - (37*3^(1/2)*dq1*dqr3*sin(2*q2)*sin(2*q3)*sin(2*q5)*cos(q4)*cos(q6))/4000 + dq2*dqr3*sin(2*q4)*cos(q2)*cos(q3)*sin(q5)*sin(q6)*((641*3^(1/2))/40000 + 37/2000) - dq3*dqr3*sin(2*q4)*cos(q2)*cos(q3)*sin(q5)*sin(q6)*((641*3^(1/2))/40000 + 37/2000);
Y1_10_11=(87*dq6*dqr4*sin(q2)*sin(q4)*sin(q6))/400 - (87*dq4*dqr4*cos(q4)*cos(q6)*sin(q2))/400 - (111*dq2*dqr4*sin(2*q5)*cos(q3)*sin(q2)*sin(q6))/8000 + (111*dq3*dqr4*sin(2*q5)*cos(q3)*sin(q2)*sin(q6))/8000 + (111*dq5*dqr4*cos(2*q5)*sin(q2)*sin(q3)*sin(q6))/4000 + (111*dq5*dqr4*sin(2*q5)*cos(q6)*sin(q2)*sin(q3))/8000 + (111*dq6*dqr4*cos(2*q5)*sin(q2)*sin(q3)*sin(q6))/16000 + (111*dq6*dqr4*sin(2*q5)*cos(q6)*sin(q2)*sin(q3))/8000 - (21*dq2*dqr4*cos(q3)*cos(q4)*cos(q6)*sin(q2))/4000 + (21*dq3*dqr4*cos(q3)*cos(q4)*cos(q6)*sin(q2))/4000 - (29*dq4*dqr4*cos(q4)*cos(q5)*cos(q6)*sin(q2))/400 - (29*dq5*dqr4*cos(q4)*cos(q5)*cos(q6)*sin(q2))/200 - (29*dq6*dqr4*cos(q4)*cos(q5)*cos(q6)*sin(q2))/100 + (29*dq4*dqr4*cos(q4)*sin(q2)*sin(q5)*sin(q6))/200 + (29*dq4*dqr4*cos(q5)*sin(q2)*sin(q4)*sin(q6))/100 + (29*dq4*dqr4*cos(q6)*sin(q2)*sin(q4)*sin(q5))/200 - (21*dq6*dqr4*cos(q4)*sin(q2)*sin(q3)*sin(q6))/4000 + (29*dq5*dqr4*cos(q4)*sin(q2)*sin(q5)*sin(q6))/100 + (29*dq5*dqr4*cos(q5)*sin(q2)*sin(q4)*sin(q6))/200 + (29*dq5*dqr4*cos(q6)*sin(q2)*sin(q4)*sin(q5))/400 + (29*dq6*dqr4*cos(q4)*sin(q2)*sin(q5)*sin(q6))/200 + (29*dq6*dqr4*cos(q5)*sin(q2)*sin(q4)*sin(q6))/400 + (29*dq6*dqr4*cos(q6)*sin(q2)*sin(q4)*sin(q5))/200 + dq2*dqr4*cos(q3)*cos(q6)*sin(q2)*((1923*3^(1/2))/80000 + 259/16000) - dq3*dqr4*cos(q3)*cos(q6)*sin(q2)*((1923*3^(1/2))/80000 + 259/16000) + (111*dq2*dqr4*cos(2*q5)*cos(q3)*cos(q6)*sin(q2))/16000 - (111*dq3*dqr4*cos(2*q5)*cos(q3)*cos(q6)*sin(q2))/16000 + dq6*dqr4*sin(q2)*sin(q3)*sin(q6)*((1923*3^(1/2))/80000 + 259/16000) + dq2*dqr4*cos(2*q4)*cos(q3)*cos(q6)*sin(q2)*((1923*3^(1/2))/80000 + 111/3200) - dq3*dqr4*cos(2*q4)*cos(q3)*cos(q6)*sin(q2)*((1923*3^(1/2))/80000 + 111/3200) - (37*dq2*dqr4*cos(2*q4)*cos(2*q5)*cos(q3)*cos(q6)*sin(q2))/3200 + (37*dq3*dqr4*cos(2*q4)*cos(2*q5)*cos(q3)*cos(q6)*sin(q2))/3200 + (37*dq2*dqr4*cos(2*q4)*sin(2*q5)*cos(q3)*sin(q2)*sin(q6))/1600 + (37*dq2*dqr4*cos(2*q5)*sin(2*q4)*cos(q3)*sin(q2)*sin(q6))/2000 + (37*dq2*dqr4*sin(2*q4)*sin(2*q5)*cos(q3)*cos(q6)*sin(q2))/4000 - (37*dq3*dqr4*cos(2*q4)*sin(2*q5)*cos(q3)*sin(q2)*sin(q6))/1600 - (37*dq3*dqr4*cos(2*q5)*sin(2*q4)*cos(q3)*sin(q2)*sin(q6))/2000 - (37*dq3*dqr4*sin(2*q4)*sin(2*q5)*cos(q3)*cos(q6)*sin(q2))/4000 - (7*dq2*dqr4*cos(q3)*cos(q4)*cos(q5)*cos(q6)*sin(q2))/4000 + (7*dq3*dqr4*cos(q3)*cos(q4)*cos(q5)*cos(q6)*sin(q2))/4000 + (1231*dq4*dqr4*cos(q3)*cos(q4)*cos(q5)*cos(q6)*sin(q2))/40000 + (877*dq6*dqr4*cos(q3)*cos(q4)*cos(q5)*cos(q6)*sin(q2))/4000 - (7*dq2*dqr4*cos(q2)*cos(q6)*sin(q3)*sin(q4)*sin(q5))/2000 + (7*dq2*dqr4*cos(q3)*cos(q4)*sin(q2)*sin(q5)*sin(q6))/2000 + (7*dq2*dqr4*cos(q3)*cos(q5)*sin(q2)*sin(q4)*sin(q6))/1000 + (7*dq2*dqr4*cos(q3)*cos(q6)*sin(q2)*sin(q4)*sin(q5))/2000 + (7*dq3*dqr4*cos(q2)*cos(q6)*sin(q3)*sin(q4)*sin(q5))/2000 - (7*dq3*dqr4*cos(q3)*cos(q4)*sin(q2)*sin(q5)*sin(q6))/2000 - (7*dq3*dqr4*cos(q3)*cos(q5)*sin(q2)*sin(q4)*sin(q6))/1000 - (7*dq3*dqr4*cos(q3)*cos(q6)*sin(q2)*sin(q4)*sin(q5))/2000 - (877*dq4*dqr4*cos(q3)*cos(q5)*sin(q2)*sin(q4)*sin(q6))/4000 - (7*dq4*dqr4*cos(q4)*cos(q5)*sin(q2)*sin(q3)*sin(q6))/1000 - (7*dq4*dqr4*cos(q4)*cos(q6)*sin(q2)*sin(q3)*sin(q5))/2000 - (877*dq5*dqr4*cos(q3)*cos(q4)*sin(q2)*sin(q5)*sin(q6))/4000 - (877*dq5*dqr4*cos(q3)*cos(q5)*sin(q2)*sin(q4)*sin(q6))/8000 - (7*dq5*dqr4*cos(q4)*cos(q5)*sin(q2)*sin(q3)*sin(q6))/2000 - (7*dq5*dqr4*cos(q4)*cos(q6)*sin(q2)*sin(q3)*sin(q5))/4000 - (877*dq6*dqr4*cos(q3)*cos(q4)*sin(q2)*sin(q5)*sin(q6))/8000 - (877*dq6*dqr4*cos(q3)*cos(q6)*sin(q2)*sin(q4)*sin(q5))/8000 - (7*dq6*dqr4*cos(q4)*cos(q5)*sin(q2)*sin(q3)*sin(q6))/4000 - (7*dq6*dqr4*cos(q4)*cos(q6)*sin(q2)*sin(q3)*sin(q5))/2000 + dq4*dqr4*cos(q3)*cos(q4)*cos(q6)*sin(q2)*((111*3^(1/2))/8000 + 7539/40000) + dq2*dqr4*cos(q3)*cos(q5)*cos(q6)*sin(q2)*((641*3^(1/2))/80000 - 37/8000) - dq3*dqr4*cos(q3)*cos(q5)*cos(q6)*sin(q2)*((641*3^(1/2))/80000 - 37/8000) - dq6*dqr4*cos(q3)*sin(q2)*sin(q4)*sin(q6)*((37*3^(1/2))/16000 + 2631/16000) - dq2*dqr4*cos(q3)*sin(q2)*sin(q5)*sin(q6)*((641*3^(1/2))/40000 + 37/2000) + dq3*dqr4*cos(q3)*sin(q2)*sin(q5)*sin(q6)*((641*3^(1/2))/40000 + 37/2000) + dq5*dqr4*cos(q5)*sin(q2)*sin(q3)*sin(q6)*((641*3^(1/2))/40000 + 37/2000) + dq6*dqr4*cos(q6)*sin(q2)*sin(q3)*sin(q5)*((641*3^(1/2))/40000 + 37/2000) + dq5*dqr4*cos(q6)*sin(q2)*sin(q3)*sin(q5)*((641*3^(1/2))/80000 - 37/8000) + dq6*dqr4*cos(q5)*sin(q2)*sin(q3)*sin(q6)*((641*3^(1/2))/80000 - 37/8000) + (37*3^(1/2)*dq5*dqr4*cos(q3)*cos(q4)*cos(q6)*sin(q2))/4000 + (37*3^(1/2)*dq6*dqr4*cos(q3)*cos(q4)*cos(q6)*sin(q2))/4000 + (37*3^(1/2)*dq4*dqr4*cos(2*q5)*cos(q3)*cos(q4)*cos(q6)*sin(q2))/8000 + (37*3^(1/2)*dq5*dqr4*cos(2*q5)*cos(q3)*cos(q4)*cos(q6)*sin(q2))/4000 + (37*3^(1/2)*dq6*dqr4*cos(2*q5)*cos(q3)*cos(q4)*cos(q6)*sin(q2))/4000 - (37*3^(1/2)*dq4*dqr4*cos(2*q5)*cos(q3)*sin(q2)*sin(q4)*sin(q6))/2000 - (37*3^(1/2)*dq4*dqr4*sin(2*q5)*cos(q3)*cos(q4)*sin(q2)*sin(q6))/4000 - (37*3^(1/2)*dq4*dqr4*sin(2*q5)*cos(q3)*cos(q6)*sin(q2)*sin(q4))/4000 - (37*3^(1/2)*dq5*dqr4*cos(2*q5)*cos(q3)*sin(q2)*sin(q4)*sin(q6))/4000 - (37*3^(1/2)*dq5*dqr4*sin(2*q5)*cos(q3)*cos(q4)*sin(q2)*sin(q6))/2000 - (37*3^(1/2)*dq5*dqr4*sin(2*q5)*cos(q3)*cos(q6)*sin(q2)*sin(q4))/8000 - (37*3^(1/2)*dq6*dqr4*cos(2*q5)*cos(q3)*sin(q2)*sin(q4)*sin(q6))/16000 - (37*3^(1/2)*dq6*dqr4*sin(2*q5)*cos(q3)*cos(q4)*sin(q2)*sin(q6))/8000 - (37*3^(1/2)*dq6*dqr4*sin(2*q5)*cos(q3)*cos(q6)*sin(q2)*sin(q4))/8000 - dq5*dqr4*cos(q3)*cos(q4)*cos(q5)*cos(q6)*sin(q2)*((37*3^(1/2))/4000 - 877/8000) - dq4*dqr4*cos(q2)*cos(q6)*sin(q3)*sin(q4)*sin(q5)*((37*3^(1/2))/4000 - 877/8000) + dq4*dqr4*cos(q3)*cos(q6)*sin(q2)*sin(q4)*sin(q5)*((37*3^(1/2))/4000 - 877/8000) + dq4*dqr4*cos(q3)*cos(q4)*sin(q2)*sin(q5)*sin(q6)*((37*3^(1/2))/2000 - 1231/20000) - dq5*dqr4*cos(q2)*cos(q6)*sin(q3)*sin(q4)*sin(q5)*((37*3^(1/2))/8000 - 877/16000) + dq5*dqr4*cos(q3)*cos(q6)*sin(q2)*sin(q4)*sin(q5)*((37*3^(1/2))/8000 - 877/16000) - dq6*dqr4*cos(q3)*cos(q5)*sin(q2)*sin(q4)*sin(q6)*((111*3^(1/2))/8000 + 877/16000) + dq2*dqr4*cos(2*q4)*cos(q3)*cos(q5)*cos(q6)*sin(q2)*((641*3^(1/2))/80000 - 37/8000) - dq3*dqr4*cos(2*q4)*cos(q3)*cos(q5)*cos(q6)*sin(q2)*((641*3^(1/2))/80000 - 37/8000) - dq2*dqr4*sin(2*q4)*cos(q3)*cos(q5)*sin(q2)*sin(q6)*((641*3^(1/2))/20000 + 37/1000) + dq3*dqr4*sin(2*q4)*cos(q3)*cos(q5)*sin(q2)*sin(q6)*((641*3^(1/2))/20000 + 37/1000) - dq2*dqr4*cos(2*q4)*cos(q3)*sin(q2)*sin(q5)*sin(q6)*((641*3^(1/2))/40000 + 37/2000) + dq3*dqr4*cos(2*q4)*cos(q3)*sin(q2)*sin(q5)*sin(q6)*((641*3^(1/2))/40000 + 37/2000) - dq2*dqr4*sin(2*q4)*cos(q3)*cos(q6)*sin(q2)*sin(q5)*((641*3^(1/2))/40000 - 37/4000) + dq3*dqr4*sin(2*q4)*cos(q3)*cos(q6)*sin(q2)*sin(q5)*((641*3^(1/2))/40000 - 37/4000);
Y1_10_12=(7*dq1*dqr4*sin(q4)*sin(q5)*sin(q6))/2000 - (87*dq1*dqr4*cos(q4)*cos(q6)*sin(q3))/800 - (7*dq1*dqr4*cos(q5)*cos(q6)*sin(q4))/4000 - (21*dq1*dqr4*cos(q6)*sin(q4))/4000 + (111*dq2*dqr4*sin(2*q5)*cos(q2)*sin(q3)*sin(q6))/8000 - (111*dq3*dqr4*sin(2*q5)*cos(q2)*sin(q3)*sin(q6))/8000 - dq1*dqr4*sin(2*q4)*sin(q5)*sin(q6)*((641*3^(1/2))/80000 + 37/4000) + (21*dq2*dqr4*cos(q2)*cos(q4)*cos(q6)*sin(q3))/4000 - (21*dq3*dqr4*cos(q2)*cos(q4)*cos(q6)*sin(q3))/4000 - (29*dq1*dqr4*cos(q4)*cos(q5)*cos(q6)*sin(q3))/800 - (21*dq4*dqr4*cos(q2)*cos(q3)*cos(q6)*sin(q4))/4000 + (29*dq1*dqr4*cos(q4)*sin(q3)*sin(q5)*sin(q6))/400 + (29*dq1*dqr4*cos(q5)*sin(q3)*sin(q4)*sin(q6))/200 + (29*dq1*dqr4*cos(q6)*sin(q3)*sin(q4)*sin(q5))/400 - dq2*dqr4*cos(q2)*cos(q6)*sin(q3)*((1923*3^(1/2))/80000 + 259/16000) + dq3*dqr4*cos(q2)*cos(q6)*sin(q3)*((1923*3^(1/2))/80000 + 259/16000) + (87*dq1*dqr4*cos(2*q2)*cos(q4)*cos(q6)*sin(q3))/800 - (111*dq2*dqr4*cos(2*q5)*cos(q2)*cos(q6)*sin(q3))/16000 + (111*dq3*dqr4*cos(2*q5)*cos(q2)*cos(q6)*sin(q3))/16000 - dq2*dqr4*cos(2*q4)*cos(q2)*cos(q6)*sin(q3)*((1923*3^(1/2))/80000 + 111/3200) + dq3*dqr4*cos(2*q4)*cos(q2)*cos(q6)*sin(q3)*((1923*3^(1/2))/80000 + 111/3200) + (37*dq2*dqr4*cos(2*q4)*cos(2*q5)*cos(q2)*cos(q6)*sin(q3))/3200 - (37*dq3*dqr4*cos(2*q4)*cos(2*q5)*cos(q2)*cos(q6)*sin(q3))/3200 + (877*dq1*dqr4*cos(2*q2)*sin(2*q3)*cos(q5)*sin(q4)*sin(q6))/8000 - (877*dq1*dqr4*cos(2*q3)*sin(2*q2)*cos(q5)*sin(q4)*sin(q6))/8000 - (37*dq2*dqr4*cos(2*q4)*sin(2*q5)*cos(q2)*sin(q3)*sin(q6))/1600 - (37*dq2*dqr4*cos(2*q5)*sin(2*q4)*cos(q2)*sin(q3)*sin(q6))/2000 - (37*dq2*dqr4*sin(2*q4)*sin(2*q5)*cos(q2)*cos(q6)*sin(q3))/4000 + (37*dq3*dqr4*cos(2*q4)*sin(2*q5)*cos(q2)*sin(q3)*sin(q6))/1600 + (37*dq3*dqr4*cos(2*q5)*sin(2*q4)*cos(q2)*sin(q3)*sin(q6))/2000 + (37*dq3*dqr4*sin(2*q4)*sin(2*q5)*cos(q2)*cos(q6)*sin(q3))/4000 + (7*dq2*dqr4*cos(q2)*cos(q4)*cos(q5)*cos(q6)*sin(q3))/4000 - (7*dq3*dqr4*cos(q2)*cos(q4)*cos(q5)*cos(q6)*sin(q3))/4000 - (7*dq4*dqr4*cos(q2)*cos(q3)*cos(q4)*cos(q6)*sin(q5))/2000 - (7*dq4*dqr4*cos(q2)*cos(q3)*cos(q5)*cos(q6)*sin(q4))/4000 - (1231*dq4*dqr4*cos(q2)*cos(q4)*cos(q5)*cos(q6)*sin(q3))/40000 - (7*dq5*dqr4*cos(q2)*cos(q3)*cos(q4)*cos(q6)*sin(q5))/4000 - (7*dq5*dqr4*cos(q2)*cos(q3)*cos(q5)*cos(q6)*sin(q4))/2000 - (7*dq6*dqr4*cos(q2)*cos(q3)*cos(q5)*cos(q6)*sin(q4))/1000 - (877*dq6*dqr4*cos(q2)*cos(q4)*cos(q5)*cos(q6)*sin(q3))/4000 - (7*dq2*dqr4*cos(q2)*cos(q4)*sin(q3)*sin(q5)*sin(q6))/2000 - (7*dq2*dqr4*cos(q2)*cos(q5)*sin(q3)*sin(q4)*sin(q6))/1000 + (7*dq3*dqr4*cos(q2)*cos(q4)*sin(q3)*sin(q5)*sin(q6))/2000 + (7*dq3*dqr4*cos(q2)*cos(q5)*sin(q3)*sin(q4)*sin(q6))/1000 + (7*dq4*dqr4*cos(q2)*cos(q3)*sin(q4)*sin(q5)*sin(q6))/2000 + (877*dq4*dqr4*cos(q2)*cos(q5)*sin(q3)*sin(q4)*sin(q6))/4000 + (7*dq5*dqr4*cos(q2)*cos(q3)*sin(q4)*sin(q5)*sin(q6))/1000 + (877*dq5*dqr4*cos(q2)*cos(q4)*sin(q3)*sin(q5)*sin(q6))/4000 + (877*dq5*dqr4*cos(q2)*cos(q5)*sin(q3)*sin(q4)*sin(q6))/8000 + (7*dq6*dqr4*cos(q2)*cos(q3)*sin(q4)*sin(q5)*sin(q6))/2000 + (877*dq6*dqr4*cos(q2)*cos(q4)*sin(q3)*sin(q5)*sin(q6))/8000 + (877*dq6*dqr4*cos(q2)*cos(q6)*sin(q3)*sin(q4)*sin(q5))/8000 - dq4*dqr4*cos(q2)*cos(q4)*cos(q6)*sin(q3)*((111*3^(1/2))/8000 + 7539/40000) - dq2*dqr4*cos(q2)*cos(q5)*cos(q6)*sin(q3)*((641*3^(1/2))/80000 - 37/8000) + dq3*dqr4*cos(q2)*cos(q5)*cos(q6)*sin(q3)*((641*3^(1/2))/80000 - 37/8000) + (29*dq1*dqr4*cos(2*q2)*cos(q4)*cos(q5)*cos(q6)*sin(q3))/800 + dq6*dqr4*cos(q2)*sin(q3)*sin(q4)*sin(q6)*((37*3^(1/2))/16000 + 2631/16000) + dq2*dqr4*cos(q2)*sin(q3)*sin(q5)*sin(q6)*((641*3^(1/2))/40000 + 37/2000) - dq3*dqr4*cos(q2)*sin(q3)*sin(q5)*sin(q6)*((641*3^(1/2))/40000 + 37/2000) - (29*dq1*dqr4*cos(2*q2)*cos(q4)*sin(q3)*sin(q5)*sin(q6))/400 - (29*dq1*dqr4*cos(2*q2)*cos(q5)*sin(q3)*sin(q4)*sin(q6))/200 - (29*dq1*dqr4*cos(2*q2)*cos(q6)*sin(q3)*sin(q4)*sin(q5))/400 + (29*dq1*dqr4*sin(2*q2)*cos(q3)*cos(q4)*sin(q5)*sin(q6))/400 + (29*dq1*dqr4*sin(2*q2)*cos(q3)*cos(q5)*sin(q4)*sin(q6))/200 + (29*dq1*dqr4*sin(2*q2)*cos(q3)*cos(q6)*sin(q4)*sin(q5))/400 - (37*3^(1/2)*dq5*dqr4*cos(q2)*cos(q4)*cos(q6)*sin(q3))/4000 - (37*3^(1/2)*dq6*dqr4*cos(q2)*cos(q4)*cos(q6)*sin(q3))/4000 - (37*3^(1/2)*dq4*dqr4*cos(2*q5)*cos(q2)*cos(q4)*cos(q6)*sin(q3))/8000 - (37*3^(1/2)*dq5*dqr4*cos(2*q5)*cos(q2)*cos(q4)*cos(q6)*sin(q3))/4000 - (37*3^(1/2)*dq6*dqr4*cos(2*q5)*cos(q2)*cos(q4)*cos(q6)*sin(q3))/4000 + (37*3^(1/2)*dq4*dqr4*cos(2*q5)*cos(q2)*sin(q3)*sin(q4)*sin(q6))/2000 + (37*3^(1/2)*dq4*dqr4*sin(2*q5)*cos(q2)*cos(q4)*sin(q3)*sin(q6))/4000 + (37*3^(1/2)*dq4*dqr4*sin(2*q5)*cos(q2)*cos(q6)*sin(q3)*sin(q4))/4000 + (37*3^(1/2)*dq5*dqr4*cos(2*q5)*cos(q2)*sin(q3)*sin(q4)*sin(q6))/4000 + (37*3^(1/2)*dq5*dqr4*sin(2*q5)*cos(q2)*cos(q4)*sin(q3)*sin(q6))/2000 + (37*3^(1/2)*dq5*dqr4*sin(2*q5)*cos(q2)*cos(q6)*sin(q3)*sin(q4))/8000 + (37*3^(1/2)*dq6*dqr4*cos(2*q5)*cos(q2)*sin(q3)*sin(q4)*sin(q6))/16000 + (37*3^(1/2)*dq6*dqr4*sin(2*q5)*cos(q2)*cos(q4)*sin(q3)*sin(q6))/8000 + (37*3^(1/2)*dq6*dqr4*sin(2*q5)*cos(q2)*cos(q6)*sin(q3)*sin(q4))/8000 - dq1*dqr4*cos(2*q2)*sin(2*q3)*cos(q6)*sin(q4)*sin(q5)*((37*3^(1/2))/8000 - 877/16000) + dq1*dqr4*cos(2*q3)*sin(2*q2)*cos(q6)*sin(q4)*sin(q5)*((37*3^(1/2))/8000 - 877/16000) - dq1*dqr4*cos(2*q2)*sin(2*q3)*cos(q4)*sin(q5)*sin(q6)*((37*3^(1/2))/4000 - 1231/40000) + dq1*dqr4*cos(2*q3)*sin(2*q2)*cos(q4)*sin(q5)*sin(q6)*((37*3^(1/2))/4000 - 1231/40000) + dq5*dqr4*cos(q2)*cos(q4)*cos(q5)*cos(q6)*sin(q3)*((37*3^(1/2))/4000 - 877/8000) - dq4*dqr4*cos(q2)*cos(q4)*sin(q3)*sin(q5)*sin(q6)*((37*3^(1/2))/2000 - 1231/20000) + dq6*dqr4*cos(q2)*cos(q5)*sin(q3)*sin(q4)*sin(q6)*((111*3^(1/2))/8000 + 877/16000) + dq1*dqr4*cos(2*q2)*cos(2*q3)*sin(2*q4)*sin(q5)*sin(q6)*((641*3^(1/2))/80000 + 37/4000) + dq1*dqr4*sin(2*q2)*sin(2*q3)*sin(2*q4)*sin(q5)*sin(q6)*((641*3^(1/2))/80000 + 37/4000) - dq2*dqr4*cos(2*q4)*cos(q2)*cos(q5)*cos(q6)*sin(q3)*((641*3^(1/2))/80000 - 37/8000) + dq3*dqr4*cos(2*q4)*cos(q2)*cos(q5)*cos(q6)*sin(q3)*((641*3^(1/2))/80000 - 37/8000) + (37*3^(1/2)*dq1*dqr4*cos(2*q2)*cos(2*q5)*sin(2*q3)*sin(q4)*sin(q6))/4000 + (37*3^(1/2)*dq1*dqr4*cos(2*q2)*sin(2*q3)*sin(2*q5)*cos(q6)*sin(q4))/8000 - (37*3^(1/2)*dq1*dqr4*cos(2*q3)*cos(2*q5)*sin(2*q2)*sin(q4)*sin(q6))/4000 - (37*3^(1/2)*dq1*dqr4*cos(2*q3)*sin(2*q2)*sin(2*q5)*cos(q6)*sin(q4))/8000 + dq2*dqr4*sin(2*q4)*cos(q2)*cos(q5)*sin(q3)*sin(q6)*((641*3^(1/2))/20000 + 37/1000) - dq3*dqr4*sin(2*q4)*cos(q2)*cos(q5)*sin(q3)*sin(q6)*((641*3^(1/2))/20000 + 37/1000) + dq2*dqr4*cos(2*q4)*cos(q2)*sin(q3)*sin(q5)*sin(q6)*((641*3^(1/2))/40000 + 37/2000) - dq3*dqr4*cos(2*q4)*cos(q2)*sin(q3)*sin(q5)*sin(q6)*((641*3^(1/2))/40000 + 37/2000) + dq2*dqr4*sin(2*q4)*cos(q2)*cos(q6)*sin(q3)*sin(q5)*((641*3^(1/2))/40000 - 37/4000) - dq3*dqr4*sin(2*q4)*cos(q2)*cos(q6)*sin(q3)*sin(q5)*((641*3^(1/2))/40000 - 37/4000);
Y1_10_13=dq1*dqr4*sin(2*q4)*cos(q6)*((1923*3^(1/2))/160000 + 111/6400) - (37*dq1*dqr4*cos(2*q4)*cos(2*q5)*sin(q6))/4000 - (37*dq1*dqr4*cos(2*q4)*sin(2*q5)*cos(q6))/8000 - (37*dq1*dqr4*cos(2*q5)*sin(2*q4)*cos(q6))/6400 + (37*dq1*dqr4*sin(2*q4)*sin(2*q5)*sin(q6))/3200 - (7*dq1*dqr4*cos(q4)*cos(q5)*sin(q6))/1000 - (7*dq1*dqr4*cos(q4)*cos(q6)*sin(q5))/2000 - (37*dq6*dqr5*sin(q2)*sin(q3)*sin(q6))/4000 + (111*dq4*dqr5*cos(2*q5)*sin(q2)*sin(q3)*sin(q6))/4000 + (111*dq4*dqr5*sin(2*q5)*cos(q6)*sin(q2)*sin(q3))/8000 + dq1*dqr4*cos(2*q4)*cos(q5)*sin(q6)*((641*3^(1/2))/40000 + 37/2000) + dq1*dqr4*cos(2*q4)*cos(q6)*sin(q5)*((641*3^(1/2))/80000 - 37/8000) + dq1*dqr4*sin(2*q4)*cos(q5)*cos(q6)*((641*3^(1/2))/160000 - 37/16000) - (21*dq6*dqr4*cos(q2)*cos(q3)*cos(q4)*sin(q6))/4000 + (29*dq4*dqr5*cos(q6)*sin(q2)*sin(q4)*sin(q5))/400 + (29*dq5*dqr5*cos(q6)*sin(q2)*sin(q4)*sin(q5))/200 + (29*dq6*dqr5*cos(q6)*sin(q2)*sin(q4)*sin(q5))/100 + dq6*dqr4*cos(q2)*cos(q3)*sin(q6)*((1923*3^(1/2))/80000 + 259/16000) - (87*dq1*dqr4*sin(2*q2)*cos(q3)*cos(q4)*cos(q6))/800 + (111*dq5*dqr4*cos(2*q5)*cos(q2)*cos(q3)*sin(q6))/4000 + (111*dq5*dqr4*sin(2*q5)*cos(q2)*cos(q3)*cos(q6))/8000 + (111*dq6*dqr4*cos(2*q5)*cos(q2)*cos(q3)*sin(q6))/16000 + (111*dq6*dqr4*sin(2*q5)*cos(q2)*cos(q3)*cos(q6))/8000 + (37*3^(1/2)*dq2*dqr5*cos(q6)*sin(q2)*sin(q3)*sin(q4))/4000 - (7*3^(1/2)*dq2*dqr5*cos(q5)*sin(q2)*sin(q3)*sin(q6))/2000 - (7*3^(1/2)*dq2*dqr5*cos(q6)*sin(q2)*sin(q3)*sin(q5))/4000 - (37*3^(1/2)*dq3*dqr5*cos(q6)*sin(q2)*sin(q3)*sin(q4))/4000 + (7*3^(1/2)*dq3*dqr5*cos(q5)*sin(q2)*sin(q3)*sin(q6))/2000 + (7*3^(1/2)*dq3*dqr5*cos(q6)*sin(q2)*sin(q3)*sin(q5))/4000 - (37*dq1*dqr4*sin(2*q2)*sin(2*q3)*sin(2*q4)*sin(2*q5)*sin(q6))/3200 - (1231*dq1*dqr4*cos(2*q2)*sin(2*q3)*cos(q4)*cos(q5)*cos(q6))/80000 + (1231*dq1*dqr4*cos(2*q3)*sin(2*q2)*cos(q4)*cos(q5)*cos(q6))/80000 - (7*dq4*dqr4*cos(q2)*cos(q3)*cos(q4)*cos(q5)*sin(q6))/1000 - (7*dq5*dqr4*cos(q2)*cos(q3)*cos(q4)*cos(q5)*sin(q6))/2000 - (7*dq6*dqr4*cos(q2)*cos(q3)*cos(q4)*cos(q5)*sin(q6))/4000 - (7*dq6*dqr4*cos(q2)*cos(q3)*cos(q4)*cos(q6)*sin(q5))/2000 - dq1*dqr4*cos(2*q2)*sin(2*q3)*cos(q4)*cos(q6)*((111*3^(1/2))/16000 + 7539/80000) + dq1*dqr4*cos(2*q3)*sin(2*q2)*cos(q4)*cos(q6)*((111*3^(1/2))/16000 + 7539/80000) + (7*dq2*dqr5*cos(q3)*cos(q5)*sin(q2)*sin(q4)*sin(q6))/2000 + (7*dq2*dqr5*cos(q3)*cos(q6)*sin(q2)*sin(q4)*sin(q5))/4000 - (7*dq3*dqr5*cos(q3)*cos(q5)*sin(q2)*sin(q4)*sin(q6))/2000 - (7*dq3*dqr5*cos(q3)*cos(q6)*sin(q2)*sin(q4)*sin(q5))/4000 - (877*dq4*dqr5*cos(q3)*cos(q5)*sin(q2)*sin(q4)*sin(q6))/8000 - (7*dq4*dqr5*cos(q4)*cos(q5)*sin(q2)*sin(q3)*sin(q6))/2000 - (7*dq4*dqr5*cos(q4)*cos(q6)*sin(q2)*sin(q3)*sin(q5))/4000 - (7*dq4*dqr5*cos(q5)*cos(q6)*sin(q2)*sin(q3)*sin(q4))/2000 - (7*dq5*dqr5*cos(q4)*cos(q5)*sin(q2)*sin(q3)*sin(q6))/1000 - (7*dq5*dqr5*cos(q4)*cos(q6)*sin(q2)*sin(q3)*sin(q5))/2000 - (7*dq5*dqr5*cos(q5)*cos(q6)*sin(q2)*sin(q3)*sin(q4))/4000 - (877*dq6*dqr5*cos(q3)*cos(q6)*sin(q2)*sin(q4)*sin(q5))/4000 - (7*dq6*dqr5*cos(q4)*cos(q5)*sin(q2)*sin(q3)*sin(q6))/2000 - (7*dq6*dqr5*cos(q4)*cos(q6)*sin(q2)*sin(q3)*sin(q5))/1000 - (7*dq6*dqr5*cos(q5)*cos(q6)*sin(q2)*sin(q3)*sin(q4))/2000 + (7*dq4*dqr5*sin(q2)*sin(q3)*sin(q4)*sin(q5)*sin(q6))/1000 + (7*dq5*dqr5*sin(q2)*sin(q3)*sin(q4)*sin(q5)*sin(q6))/2000 + (7*dq6*dqr5*sin(q2)*sin(q3)*sin(q4)*sin(q5)*sin(q6))/4000 + dq5*dqr4*cos(q2)*cos(q3)*cos(q5)*sin(q6)*((641*3^(1/2))/40000 + 37/2000) + dq6*dqr4*cos(q2)*cos(q3)*cos(q6)*sin(q5)*((641*3^(1/2))/40000 + 37/2000) + dq5*dqr4*cos(q2)*cos(q3)*cos(q6)*sin(q5)*((641*3^(1/2))/80000 - 37/8000) + dq6*dqr4*cos(q2)*cos(q3)*cos(q5)*sin(q6)*((641*3^(1/2))/80000 - 37/8000) - (29*dq1*dqr4*sin(2*q2)*cos(q3)*cos(q4)*cos(q5)*cos(q6))/800 - dq1*dqr4*cos(2*q2)*cos(2*q3)*sin(2*q4)*cos(q6)*((1923*3^(1/2))/160000 + 111/6400) + dq5*dqr5*cos(q5)*sin(q2)*sin(q3)*sin(q6)*((641*3^(1/2))/20000 + 37/1000) + dq6*dqr5*cos(q6)*sin(q2)*sin(q3)*sin(q5)*((641*3^(1/2))/20000 + 37/1000) + dq4*dqr5*cos(q5)*sin(q2)*sin(q3)*sin(q6)*((641*3^(1/2))/40000 + 37/2000) + dq6*dqr5*cos(q5)*sin(q2)*sin(q3)*sin(q6)*((641*3^(1/2))/40000 + 37/2000) + dq5*dqr5*cos(q6)*sin(q2)*sin(q3)*sin(q5)*((641*3^(1/2))/40000 - 37/4000) + dq4*dqr5*cos(q6)*sin(q2)*sin(q3)*sin(q5)*((641*3^(1/2))/80000 - 37/8000) + (37*dq1*dqr4*cos(2*q2)*cos(2*q3)*cos(2*q4)*cos(2*q5)*sin(q6))/4000 + (37*dq1*dqr4*cos(2*q2)*cos(2*q3)*cos(2*q4)*sin(2*q5)*cos(q6))/8000 + (37*dq1*dqr4*cos(2*q2)*cos(2*q3)*cos(2*q5)*sin(2*q4)*cos(q6))/6400 - dq1*dqr4*sin(2*q2)*sin(2*q3)*sin(2*q4)*cos(q6)*((1923*3^(1/2))/160000 + 111/6400) - (37*dq1*dqr4*cos(2*q2)*cos(2*q3)*sin(2*q4)*sin(2*q5)*sin(q6))/3200 + (37*dq1*dqr4*cos(2*q4)*cos(2*q5)*sin(2*q2)*sin(2*q3)*sin(q6))/4000 + (37*dq1*dqr4*cos(2*q4)*sin(2*q2)*sin(2*q3)*sin(2*q5)*cos(q6))/8000 + (37*dq1*dqr4*cos(2*q5)*sin(2*q2)*sin(2*q3)*sin(2*q4)*cos(q6))/6400 - (37*3^(1/2)*dq2*dqr5*cos(2*q5)*cos(q4)*sin(q2)*sin(q3)*sin(q6))/4000 - (37*3^(1/2)*dq2*dqr5*cos(2*q5)*cos(q6)*sin(q2)*sin(q3)*sin(q4))/4000 - (37*3^(1/2)*dq2*dqr5*sin(2*q5)*cos(q4)*cos(q6)*sin(q2)*sin(q3))/8000 + (37*3^(1/2)*dq3*dqr5*cos(2*q5)*cos(q4)*sin(q2)*sin(q3)*sin(q6))/4000 + (37*3^(1/2)*dq3*dqr5*cos(2*q5)*cos(q6)*sin(q2)*sin(q3)*sin(q4))/4000 + (37*3^(1/2)*dq3*dqr5*sin(2*q5)*cos(q4)*cos(q6)*sin(q2)*sin(q3))/8000 + (37*3^(1/2)*dq2*dqr5*sin(2*q5)*sin(q2)*sin(q3)*sin(q4)*sin(q6))/2000 - (37*3^(1/2)*dq3*dqr5*sin(2*q5)*sin(q2)*sin(q3)*sin(q4)*sin(q6))/2000 - dq1*dqr4*cos(2*q2)*cos(2*q3)*cos(2*q4)*cos(q5)*sin(q6)*((641*3^(1/2))/40000 + 37/2000) - dq1*dqr4*cos(2*q2)*cos(2*q3)*cos(2*q4)*cos(q6)*sin(q5)*((641*3^(1/2))/80000 - 37/8000) - dq1*dqr4*cos(2*q2)*cos(2*q3)*sin(2*q4)*cos(q5)*cos(q6)*((641*3^(1/2))/160000 - 37/16000) + dq5*dqr5*cos(q3)*cos(q6)*sin(q2)*sin(q4)*sin(q5)*((37*3^(1/2))/4000 - 877/8000) + dq4*dqr5*cos(q3)*cos(q6)*sin(q2)*sin(q4)*sin(q5)*((37*3^(1/2))/8000 - 877/16000) + dq2*dqr5*cos(q4)*cos(q5)*sin(q2)*sin(q3)*sin(q6)*((37*3^(1/2))/2000 + 1923/40000) - dq3*dqr5*cos(q4)*cos(q5)*sin(q2)*sin(q3)*sin(q6)*((37*3^(1/2))/2000 + 1923/40000) - dq2*dqr5*cos(q4)*cos(q6)*sin(q2)*sin(q3)*sin(q5)*((37*3^(1/2))/8000 - 1923/80000) + dq3*dqr5*cos(q4)*cos(q6)*sin(q2)*sin(q3)*sin(q5)*((37*3^(1/2))/8000 - 1923/80000) - dq1*dqr4*cos(2*q4)*sin(2*q2)*sin(2*q3)*cos(q5)*sin(q6)*((641*3^(1/2))/40000 + 37/2000) - dq1*dqr4*cos(2*q4)*sin(2*q2)*sin(2*q3)*cos(q6)*sin(q5)*((641*3^(1/2))/80000 - 37/8000) - dq1*dqr4*sin(2*q2)*sin(2*q3)*sin(2*q4)*cos(q5)*cos(q6)*((641*3^(1/2))/160000 - 37/16000) - (37*3^(1/2)*dq1*dqr4*cos(2*q2)*cos(2*q5)*sin(2*q3)*cos(q4)*cos(q6))/16000 + (37*3^(1/2)*dq1*dqr4*cos(2*q3)*cos(2*q5)*sin(2*q2)*cos(q4)*cos(q6))/16000 + (37*3^(1/2)*dq1*dqr4*cos(2*q2)*sin(2*q3)*sin(2*q5)*cos(q4)*sin(q6))/8000 - (37*3^(1/2)*dq1*dqr4*cos(2*q3)*sin(2*q2)*sin(2*q5)*cos(q4)*sin(q6))/8000;
Y1_10_14=(37*dq3*dqr5*cos(q3)*cos(q6)*sin(q2))/4000 - (37*dq2*dqr5*cos(q3)*cos(q6)*sin(q2))/4000 - (29*dq4*dqr5*cos(q4)*cos(q5)*cos(q6)*sin(q2))/200 - (29*dq5*dqr5*cos(q4)*cos(q5)*cos(q6)*sin(q2))/400 - (29*dq6*dqr5*cos(q4)*cos(q5)*cos(q6)*sin(q2))/200 + (29*dq1*dqr5*cos(q4)*sin(q3)*sin(q5)*sin(q6))/200 + (29*dq1*dqr5*cos(q5)*sin(q3)*sin(q4)*sin(q6))/400 + (29*dq1*dqr5*cos(q6)*sin(q3)*sin(q4)*sin(q5))/800 + (29*dq4*dqr5*cos(q4)*sin(q2)*sin(q5)*sin(q6))/100 + (29*dq4*dqr5*cos(q5)*sin(q2)*sin(q4)*sin(q6))/200 + (29*dq5*dqr5*cos(q4)*sin(q2)*sin(q5)*sin(q6))/200 + (29*dq5*dqr5*cos(q5)*sin(q2)*sin(q4)*sin(q6))/100 + (29*dq6*dqr5*cos(q4)*sin(q2)*sin(q5)*sin(q6))/400 + (29*dq6*dqr5*cos(q5)*sin(q2)*sin(q4)*sin(q6))/200 - (7*3^(1/2)*dq5*dqr5*cos(q2)*sin(q3)*sin(q5)*sin(q6))/2000 + (7*3^(1/2)*dq5*dqr5*cos(q3)*sin(q2)*sin(q5)*sin(q6))/2000 + (37*3^(1/2)*dq6*dqr5*cos(q2)*sin(q3)*sin(q4)*sin(q6))/4000 - (37*3^(1/2)*dq6*dqr5*cos(q3)*sin(q2)*sin(q4)*sin(q6))/4000 - (7*3^(1/2)*dq6*dqr5*cos(q2)*sin(q3)*sin(q5)*sin(q6))/4000 + (7*3^(1/2)*dq6*dqr5*cos(q3)*sin(q2)*sin(q5)*sin(q6))/4000 - (37*dq2*dqr5*cos(2*q4)*cos(2*q5)*cos(q3)*cos(q6)*sin(q2))/4000 + (37*dq3*dqr5*cos(2*q4)*cos(2*q5)*cos(q3)*cos(q6)*sin(q2))/4000 - (37*dq2*dqr5*cos(2*q4)*sin(2*q5)*cos(q2)*sin(q3)*sin(q6))/2000 + (37*dq2*dqr5*cos(2*q4)*sin(2*q5)*cos(q3)*sin(q2)*sin(q6))/2000 - (37*dq2*dqr5*cos(2*q5)*sin(2*q4)*cos(q2)*sin(q3)*sin(q6))/1600 + (37*dq2*dqr5*cos(2*q5)*sin(2*q4)*cos(q3)*sin(q2)*sin(q6))/1600 + (37*dq2*dqr5*sin(2*q4)*sin(2*q5)*cos(q3)*cos(q6)*sin(q2))/3200 + (37*dq3*dqr5*cos(2*q4)*sin(2*q5)*cos(q2)*sin(q3)*sin(q6))/2000 - (37*dq3*dqr5*cos(2*q4)*sin(2*q5)*cos(q3)*sin(q2)*sin(q6))/2000 + (37*dq3*dqr5*cos(2*q5)*sin(2*q4)*cos(q2)*sin(q3)*sin(q6))/1600 - (37*dq3*dqr5*cos(2*q5)*sin(2*q4)*cos(q3)*sin(q2)*sin(q6))/1600 - (37*dq3*dqr5*sin(2*q4)*sin(2*q5)*cos(q3)*cos(q6)*sin(q2))/3200 + (7*dq2*dqr5*cos(q2)*cos(q4)*cos(q5)*cos(q6)*sin(q3))/2000 - (7*dq2*dqr5*cos(q3)*cos(q4)*cos(q5)*cos(q6)*sin(q2))/2000 - (7*dq3*dqr5*cos(q2)*cos(q4)*cos(q5)*cos(q6)*sin(q3))/2000 + (7*dq3*dqr5*cos(q3)*cos(q4)*cos(q5)*cos(q6)*sin(q2))/2000 - (29*3^(1/2)*dq1*dqr5*sin(2*q2)*cos(q5)*sin(q3)*sin(q6))/400 - (29*3^(1/2)*dq1*dqr5*sin(2*q2)*cos(q6)*sin(q3)*sin(q5))/800 - (7*dq2*dqr5*cos(q2)*cos(q4)*sin(q3)*sin(q5)*sin(q6))/1000 - (7*dq2*dqr5*cos(q2)*cos(q5)*sin(q3)*sin(q4)*sin(q6))/2000 - (7*dq2*dqr5*cos(q2)*cos(q6)*sin(q3)*sin(q4)*sin(q5))/4000 + (7*dq2*dqr5*cos(q3)*cos(q4)*sin(q2)*sin(q5)*sin(q6))/1000 + (7*dq3*dqr5*cos(q2)*cos(q4)*sin(q3)*sin(q5)*sin(q6))/1000 + (7*dq3*dqr5*cos(q2)*cos(q5)*sin(q3)*sin(q4)*sin(q6))/2000 + (7*dq3*dqr5*cos(q2)*cos(q6)*sin(q3)*sin(q4)*sin(q5))/4000 - (7*dq3*dqr5*cos(q3)*cos(q4)*sin(q2)*sin(q5)*sin(q6))/1000 + (877*dq4*dqr5*cos(q2)*cos(q4)*sin(q3)*sin(q5)*sin(q6))/4000 + (877*dq4*dqr5*cos(q2)*cos(q5)*sin(q3)*sin(q4)*sin(q6))/8000 - (877*dq4*dqr5*cos(q3)*cos(q4)*sin(q2)*sin(q5)*sin(q6))/4000 + (877*dq5*dqr5*cos(q2)*cos(q5)*sin(q3)*sin(q4)*sin(q6))/4000 - (877*dq5*dqr5*cos(q3)*cos(q5)*sin(q2)*sin(q4)*sin(q6))/4000 + (877*dq6*dqr5*cos(q2)*cos(q5)*sin(q3)*sin(q4)*sin(q6))/8000 + (877*dq6*dqr5*cos(q2)*cos(q6)*sin(q3)*sin(q4)*sin(q5))/4000 - (877*dq6*dqr5*cos(q3)*cos(q5)*sin(q2)*sin(q4)*sin(q6))/8000 + dq2*dqr5*cos(q3)*cos(q5)*cos(q6)*sin(q2)*((641*3^(1/2))/80000 - 37/8000) - dq3*dqr5*cos(q3)*cos(q5)*cos(q6)*sin(q2)*((641*3^(1/2))/80000 - 37/8000) + dq2*dqr5*cos(q2)*sin(q3)*sin(q5)*sin(q6)*((641*3^(1/2))/40000 + 37/2000) - dq2*dqr5*cos(q3)*sin(q2)*sin(q5)*sin(q6)*((641*3^(1/2))/40000 + 37/2000) - dq3*dqr5*cos(q2)*sin(q3)*sin(q5)*sin(q6)*((641*3^(1/2))/40000 + 37/2000) + dq3*dqr5*cos(q3)*sin(q2)*sin(q5)*sin(q6)*((641*3^(1/2))/40000 + 37/2000) - (29*dq1*dqr5*cos(2*q2)*cos(q4)*sin(q3)*sin(q5)*sin(q6))/200 - (29*dq1*dqr5*cos(2*q2)*cos(q5)*sin(q3)*sin(q4)*sin(q6))/400 - (29*dq1*dqr5*cos(2*q2)*cos(q6)*sin(q3)*sin(q4)*sin(q5))/800 + (37*3^(1/2)*dq4*dqr5*cos(q3)*cos(q4)*cos(q6)*sin(q2))/4000 - (7*3^(1/2)*dq5*dqr5*cos(q3)*cos(q5)*cos(q6)*sin(q2))/4000 - (7*3^(1/2)*dq6*dqr5*cos(q3)*cos(q5)*cos(q6)*sin(q2))/2000 - (37*3^(1/2)*dq4*dqr5*cos(2*q5)*cos(q2)*cos(q4)*cos(q6)*sin(q3))/4000 + (37*3^(1/2)*dq4*dqr5*cos(2*q5)*cos(q3)*cos(q4)*cos(q6)*sin(q2))/4000 + (37*3^(1/2)*dq4*dqr5*cos(2*q5)*cos(q2)*sin(q3)*sin(q4)*sin(q6))/4000 - (37*3^(1/2)*dq4*dqr5*cos(2*q5)*cos(q3)*sin(q2)*sin(q4)*sin(q6))/4000 + (37*3^(1/2)*dq4*dqr5*sin(2*q5)*cos(q2)*cos(q4)*sin(q3)*sin(q6))/2000 + (37*3^(1/2)*dq4*dqr5*sin(2*q5)*cos(q2)*cos(q6)*sin(q3)*sin(q4))/8000 - (37*3^(1/2)*dq4*dqr5*sin(2*q5)*cos(q3)*cos(q4)*sin(q2)*sin(q6))/2000 - (37*3^(1/2)*dq4*dqr5*sin(2*q5)*cos(q3)*cos(q6)*sin(q2)*sin(q4))/8000 + dq4*dqr5*cos(q2)*cos(q4)*cos(q5)*cos(q6)*sin(q3)*((37*3^(1/2))/4000 - 877/8000) - dq4*dqr5*cos(q3)*cos(q4)*cos(q5)*cos(q6)*sin(q2)*((37*3^(1/2))/4000 - 877/8000) - dq6*dqr5*cos(q2)*cos(q4)*cos(q5)*cos(q6)*sin(q3)*((37*3^(1/2))/2000 + 1577/10000) + dq6*dqr5*cos(q3)*cos(q4)*cos(q5)*cos(q6)*sin(q2)*((37*3^(1/2))/2000 + 1577/10000) + dq5*dqr5*cos(q2)*cos(q4)*cos(q5)*cos(q6)*sin(q3)*((37*3^(1/2))/4000 - 1577/20000) - dq5*dqr5*cos(q3)*cos(q4)*cos(q5)*cos(q6)*sin(q2)*((37*3^(1/2))/4000 - 1577/20000) - dq5*dqr5*cos(q2)*cos(q6)*sin(q3)*sin(q4)*sin(q5)*((37*3^(1/2))/4000 - 877/8000) + dq5*dqr5*cos(q2)*cos(q4)*sin(q3)*sin(q5)*sin(q6)*((37*3^(1/2))/2000 + 1577/10000) - dq5*dqr5*cos(q3)*cos(q4)*sin(q2)*sin(q5)*sin(q6)*((37*3^(1/2))/2000 + 1577/10000) - dq4*dqr5*cos(q2)*cos(q6)*sin(q3)*sin(q4)*sin(q5)*((37*3^(1/2))/8000 - 877/16000) + dq6*dqr5*cos(q2)*cos(q4)*sin(q3)*sin(q5)*sin(q6)*((37*3^(1/2))/4000 + 1577/20000) - dq6*dqr5*cos(q3)*cos(q4)*sin(q2)*sin(q5)*sin(q6)*((37*3^(1/2))/4000 + 1577/20000) + dq2*dqr5*cos(2*q4)*cos(q3)*cos(q5)*cos(q6)*sin(q2)*((641*3^(1/2))/80000 - 37/8000) - dq3*dqr5*cos(2*q4)*cos(q3)*cos(q5)*cos(q6)*sin(q2)*((641*3^(1/2))/80000 - 37/8000) + dq2*dqr5*cos(2*q4)*cos(q2)*sin(q3)*sin(q5)*sin(q6)*((641*3^(1/2))/40000 + 37/2000) - dq2*dqr5*cos(2*q4)*cos(q3)*sin(q2)*sin(q5)*sin(q6)*((641*3^(1/2))/40000 + 37/2000) - dq3*dqr5*cos(2*q4)*cos(q2)*sin(q3)*sin(q5)*sin(q6)*((641*3^(1/2))/40000 + 37/2000) + dq3*dqr5*cos(2*q4)*cos(q3)*sin(q2)*sin(q5)*sin(q6)*((641*3^(1/2))/40000 + 37/2000) + dq2*dqr5*sin(2*q4)*cos(q2)*cos(q5)*sin(q3)*sin(q6)*((641*3^(1/2))/80000 + 37/4000) - dq2*dqr5*sin(2*q4)*cos(q3)*cos(q5)*sin(q2)*sin(q6)*((641*3^(1/2))/80000 + 37/4000) - dq3*dqr5*sin(2*q4)*cos(q2)*cos(q5)*sin(q3)*sin(q6)*((641*3^(1/2))/80000 + 37/4000) + dq3*dqr5*sin(2*q4)*cos(q3)*cos(q5)*sin(q2)*sin(q6)*((641*3^(1/2))/80000 + 37/4000) + dq2*dqr5*sin(2*q4)*cos(q2)*cos(q6)*sin(q3)*sin(q5)*((641*3^(1/2))/160000 - 37/16000) - dq2*dqr5*sin(2*q4)*cos(q3)*cos(q6)*sin(q2)*sin(q5)*((641*3^(1/2))/160000 - 37/16000) - dq3*dqr5*sin(2*q4)*cos(q2)*cos(q6)*sin(q3)*sin(q5)*((641*3^(1/2))/160000 - 37/16000) + dq3*dqr5*sin(2*q4)*cos(q3)*cos(q6)*sin(q2)*sin(q5)*((641*3^(1/2))/160000 - 37/16000);
Y1_10_15=(111*dq1*dqr5*cos(2*q5)*sin(q6))/16000 - (37*dq1*dqr5*cos(2*q4)*cos(2*q5)*sin(q6))/3200 + (37*dq1*dqr5*sin(2*q4)*sin(2*q5)*sin(q6))/4000 + (37*dq2*dqr5*cos(q2)*cos(q6)*sin(q3))/4000 - (37*dq3*dqr5*cos(q2)*cos(q6)*sin(q3))/4000 - (7*dq1*dqr5*cos(q4)*cos(q5)*sin(q6))/2000 - (7*dq1*dqr5*cos(q4)*cos(q6)*sin(q5))/4000 - (7*dq1*dqr5*cos(q5)*cos(q6)*sin(q4))/2000 - (37*dq6*dqr5*cos(q2)*cos(q3)*sin(q6))/4000 + (7*dq1*dqr5*sin(q4)*sin(q5)*sin(q6))/1000 - dq1*dqr5*cos(q5)*sin(q6)*((6847*3^(1/2))/160000 - 111/8000) - dq1*dqr5*cos(q6)*sin(q5)*((6847*3^(1/2))/320000 - 111/32000) + (29*3^(1/2)*dq1*dqr5*cos(q3)*cos(q5)*sin(q6))/400 + (29*3^(1/2)*dq1*dqr5*cos(q3)*cos(q6)*sin(q5))/800 + dq1*dqr5*cos(2*q4)*cos(q5)*sin(q6)*((641*3^(1/2))/160000 + 37/8000) + dq1*dqr5*cos(2*q4)*cos(q6)*sin(q5)*((641*3^(1/2))/320000 - 37/32000) - dq1*dqr5*sin(2*q4)*sin(q5)*sin(q6)*((641*3^(1/2))/80000 + 37/4000) - (29*dq1*dqr5*cos(q4)*cos(q5)*cos(q6)*sin(q3))/400 + (333*dq1*dqr5*cos(2*q2)*cos(2*q3)*cos(2*q5)*sin(q6))/16000 + (333*dq1*dqr5*cos(2*q5)*sin(2*q2)*sin(2*q3)*sin(q6))/16000 + (111*dq4*dqr5*cos(2*q5)*cos(q2)*cos(q3)*sin(q6))/4000 - (37*dq1*dqr5*sin(2*q2)*sin(2*q3)*sin(2*q4)*sin(2*q5)*sin(q6))/4000 + (37*dq2*dqr5*cos(2*q4)*cos(2*q5)*cos(q2)*cos(q6)*sin(q3))/4000 - (37*dq3*dqr5*cos(2*q4)*cos(2*q5)*cos(q2)*cos(q6)*sin(q3))/4000 + (877*dq1*dqr5*cos(2*q2)*sin(2*q3)*cos(q4)*sin(q5)*sin(q6))/8000 + (1231*dq1*dqr5*cos(2*q2)*sin(2*q3)*cos(q6)*sin(q4)*sin(q5))/80000 - (877*dq1*dqr5*cos(2*q3)*sin(2*q2)*cos(q4)*sin(q5)*sin(q6))/8000 - (1231*dq1*dqr5*cos(2*q3)*sin(2*q2)*cos(q6)*sin(q4)*sin(q5))/80000 - (37*dq2*dqr5*sin(2*q4)*sin(2*q5)*cos(q2)*cos(q6)*sin(q3))/3200 + (37*dq3*dqr5*sin(2*q4)*sin(2*q5)*cos(q2)*cos(q6)*sin(q3))/3200 - (29*3^(1/2)*dq1*dqr5*cos(2*q2)*cos(q3)*cos(q5)*sin(q6))/400 - (29*3^(1/2)*dq1*dqr5*cos(2*q2)*cos(q3)*cos(q6)*sin(q5))/800 - (7*dq4*dqr5*cos(q2)*cos(q3)*cos(q4)*cos(q5)*sin(q6))/2000 - (7*dq4*dqr5*cos(q2)*cos(q3)*cos(q4)*cos(q6)*sin(q5))/4000 - (7*dq4*dqr5*cos(q2)*cos(q3)*cos(q5)*cos(q6)*sin(q4))/2000 - (7*dq5*dqr5*cos(q2)*cos(q3)*cos(q4)*cos(q5)*sin(q6))/1000 - (7*dq5*dqr5*cos(q2)*cos(q3)*cos(q4)*cos(q6)*sin(q5))/2000 - (7*dq5*dqr5*cos(q2)*cos(q3)*cos(q5)*cos(q6)*sin(q4))/4000 - (7*dq6*dqr5*cos(q2)*cos(q3)*cos(q4)*cos(q5)*sin(q6))/2000 - (7*dq6*dqr5*cos(q2)*cos(q3)*cos(q4)*cos(q6)*sin(q5))/1000 - (7*dq6*dqr5*cos(q2)*cos(q3)*cos(q5)*cos(q6)*sin(q4))/2000 + dq1*dqr5*cos(2*q2)*cos(2*q3)*cos(q5)*sin(q6)*((9411*3^(1/2))/160000 + 37/8000) + dq1*dqr5*cos(2*q2)*cos(2*q3)*cos(q6)*sin(q5)*((9411*3^(1/2))/320000 - 259/32000) + (7*dq4*dqr5*cos(q2)*cos(q3)*sin(q4)*sin(q5)*sin(q6))/1000 + (7*dq5*dqr5*cos(q2)*cos(q3)*sin(q4)*sin(q5)*sin(q6))/2000 + (7*dq6*dqr5*cos(q2)*cos(q3)*sin(q4)*sin(q5)*sin(q6))/4000 + dq1*dqr5*sin(2*q2)*sin(2*q3)*cos(q5)*sin(q6)*((9411*3^(1/2))/160000 + 37/8000) + dq1*dqr5*sin(2*q2)*sin(2*q3)*cos(q6)*sin(q5)*((9411*3^(1/2))/320000 - 259/32000) + dq5*dqr5*cos(q2)*cos(q3)*cos(q5)*sin(q6)*((641*3^(1/2))/20000 + 37/1000) + dq6*dqr5*cos(q2)*cos(q3)*cos(q6)*sin(q5)*((641*3^(1/2))/20000 + 37/1000) + dq4*dqr5*cos(q2)*cos(q3)*cos(q5)*sin(q6)*((641*3^(1/2))/40000 + 37/2000) + dq6*dqr5*cos(q2)*cos(q3)*cos(q5)*sin(q6)*((641*3^(1/2))/40000 + 37/2000) + dq5*dqr5*cos(q2)*cos(q3)*cos(q6)*sin(q5)*((641*3^(1/2))/40000 - 37/4000) - dq2*dqr5*cos(q2)*cos(q5)*cos(q6)*sin(q3)*((641*3^(1/2))/80000 - 37/8000) + dq3*dqr5*cos(q2)*cos(q5)*cos(q6)*sin(q3)*((641*3^(1/2))/80000 - 37/8000) + dq4*dqr5*cos(q2)*cos(q3)*cos(q6)*sin(q5)*((641*3^(1/2))/80000 - 37/8000) + (29*dq1*dqr5*cos(2*q2)*cos(q4)*cos(q5)*cos(q6)*sin(q3))/400 + (37*dq1*dqr5*cos(2*q2)*cos(2*q3)*cos(2*q4)*cos(2*q5)*sin(q6))/3200 + (29*dq1*dqr5*sin(2*q2)*cos(q3)*cos(q4)*sin(q5)*sin(q6))/200 + (29*dq1*dqr5*sin(2*q2)*cos(q3)*cos(q5)*sin(q4)*sin(q6))/400 + (29*dq1*dqr5*sin(2*q2)*cos(q3)*cos(q6)*sin(q4)*sin(q5))/800 + (37*3^(1/2)*dq2*dqr5*cos(q2)*cos(q3)*cos(q6)*sin(q4))/4000 - (7*3^(1/2)*dq2*dqr5*cos(q2)*cos(q3)*cos(q5)*sin(q6))/2000 - (7*3^(1/2)*dq2*dqr5*cos(q2)*cos(q3)*cos(q6)*sin(q5))/4000 - (37*3^(1/2)*dq3*dqr5*cos(q2)*cos(q3)*cos(q6)*sin(q4))/4000 + (7*3^(1/2)*dq3*dqr5*cos(q2)*cos(q3)*cos(q5)*sin(q6))/2000 + (7*3^(1/2)*dq3*dqr5*cos(q2)*cos(q3)*cos(q6)*sin(q5))/4000 - (37*3^(1/2)*dq4*dqr5*cos(q2)*cos(q4)*cos(q6)*sin(q3))/4000 + (7*3^(1/2)*dq5*dqr5*cos(q2)*cos(q5)*cos(q6)*sin(q3))/4000 + (7*3^(1/2)*dq6*dqr5*cos(q2)*cos(q5)*cos(q6)*sin(q3))/2000 - (37*dq1*dqr5*cos(2*q2)*cos(2*q3)*sin(2*q4)*sin(2*q5)*sin(q6))/4000 + (37*dq1*dqr5*cos(2*q4)*cos(2*q5)*sin(2*q2)*sin(2*q3)*sin(q6))/3200 - (37*3^(1/2)*dq2*dqr5*cos(2*q5)*cos(q2)*cos(q3)*cos(q4)*sin(q6))/4000 - (37*3^(1/2)*dq2*dqr5*cos(2*q5)*cos(q2)*cos(q3)*cos(q6)*sin(q4))/4000 - (37*3^(1/2)*dq2*dqr5*sin(2*q5)*cos(q2)*cos(q3)*cos(q4)*cos(q6))/8000 + (37*3^(1/2)*dq3*dqr5*cos(2*q5)*cos(q2)*cos(q3)*cos(q4)*sin(q6))/4000 + (37*3^(1/2)*dq3*dqr5*cos(2*q5)*cos(q2)*cos(q3)*cos(q6)*sin(q4))/4000 + (37*3^(1/2)*dq3*dqr5*sin(2*q5)*cos(q2)*cos(q3)*cos(q4)*cos(q6))/8000 + (37*3^(1/2)*dq2*dqr5*sin(2*q5)*cos(q2)*cos(q3)*sin(q4)*sin(q6))/2000 - (37*3^(1/2)*dq3*dqr5*sin(2*q5)*cos(q2)*cos(q3)*sin(q4)*sin(q6))/2000 - dq1*dqr5*cos(2*q2)*sin(2*q3)*cos(q5)*sin(q4)*sin(q6)*((37*3^(1/2))/4000 - 1231/40000) + dq1*dqr5*cos(2*q3)*sin(2*q2)*cos(q5)*sin(q4)*sin(q6)*((37*3^(1/2))/4000 - 1231/40000) + dq2*dqr5*cos(q2)*cos(q3)*cos(q4)*cos(q5)*sin(q6)*((37*3^(1/2))/2000 + 1923/40000) - dq3*dqr5*cos(q2)*cos(q3)*cos(q4)*cos(q5)*sin(q6)*((37*3^(1/2))/2000 + 1923/40000) - dq2*dqr5*cos(q2)*cos(q3)*cos(q4)*cos(q6)*sin(q5)*((37*3^(1/2))/8000 - 1923/80000) + dq3*dqr5*cos(q2)*cos(q3)*cos(q4)*cos(q6)*sin(q5)*((37*3^(1/2))/8000 - 1923/80000) - dq1*dqr5*cos(2*q2)*cos(2*q3)*cos(2*q4)*cos(q5)*sin(q6)*((641*3^(1/2))/160000 + 37/8000) - dq1*dqr5*cos(2*q2)*cos(2*q3)*cos(2*q4)*cos(q6)*sin(q5)*((641*3^(1/2))/320000 - 37/32000) + dq1*dqr5*cos(2*q2)*cos(2*q3)*sin(2*q4)*sin(q5)*sin(q6)*((641*3^(1/2))/80000 + 37/4000) - dq1*dqr5*cos(2*q4)*sin(2*q2)*sin(2*q3)*cos(q5)*sin(q6)*((641*3^(1/2))/160000 + 37/8000) - dq1*dqr5*cos(2*q4)*sin(2*q2)*sin(2*q3)*cos(q6)*sin(q5)*((641*3^(1/2))/320000 - 37/32000) + dq1*dqr5*sin(2*q2)*sin(2*q3)*sin(2*q4)*sin(q5)*sin(q6)*((641*3^(1/2))/80000 + 37/4000) - dq2*dqr5*cos(2*q4)*cos(q2)*cos(q5)*cos(q6)*sin(q3)*((641*3^(1/2))/80000 - 37/8000) + dq3*dqr5*cos(2*q4)*cos(q2)*cos(q5)*cos(q6)*sin(q3)*((641*3^(1/2))/80000 - 37/8000) + (37*3^(1/2)*dq1*dqr5*cos(2*q2)*cos(2*q5)*sin(2*q3)*sin(q4)*sin(q6))/4000 + (37*3^(1/2)*dq1*dqr5*cos(2*q2)*sin(2*q3)*sin(2*q5)*cos(q4)*sin(q6))/2000 + (37*3^(1/2)*dq1*dqr5*cos(2*q2)*sin(2*q3)*sin(2*q5)*cos(q6)*sin(q4))/8000 - (37*3^(1/2)*dq1*dqr5*cos(2*q3)*cos(2*q5)*sin(2*q2)*sin(q4)*sin(q6))/4000 - (37*3^(1/2)*dq1*dqr5*cos(2*q3)*sin(2*q2)*sin(2*q5)*cos(q4)*sin(q6))/2000 - (37*3^(1/2)*dq1*dqr5*cos(2*q3)*sin(2*q2)*sin(2*q5)*cos(q6)*sin(q4))/8000;
Y1_10_16=(111*dq1*dqr5*sin(2*q5)*cos(q6))/32000 - (37*dq1*dqr5*cos(2*q4)*sin(2*q5)*cos(q6))/6400 - (37*dq1*dqr5*cos(2*q5)*sin(2*q4)*cos(q6))/8000 + (87*dq4*dqr6*sin(q2)*sin(q4)*sin(q6))/400 - (37*dq5*dqr6*sin(q2)*sin(q3)*sin(q6))/4000 - (37*dq6*dqr6*sin(q2)*sin(q3)*sin(q6))/2000 + (111*dq4*dqr6*cos(2*q5)*sin(q2)*sin(q3)*sin(q6))/16000 + (111*dq4*dqr6*sin(2*q5)*cos(q6)*sin(q2)*sin(q3))/8000 + dq1*dqr5*sin(2*q4)*cos(q5)*cos(q6)*((641*3^(1/2))/160000 - 37/16000) + (7*3^(1/2)*dq2*dqr6*sin(q2)*sin(q3)*sin(q6))/4000 - (7*3^(1/2)*dq3*dqr6*sin(q2)*sin(q3)*sin(q6))/4000 + (333*dq1*dqr5*cos(2*q2)*cos(2*q3)*sin(2*q5)*cos(q6))/32000 + (21*dq2*dqr6*cos(q3)*sin(q2)*sin(q4)*sin(q6))/4000 - (21*dq3*dqr6*cos(q3)*sin(q2)*sin(q4)*sin(q6))/4000 - (21*dq4*dqr6*cos(q4)*sin(q2)*sin(q3)*sin(q6))/4000 + (29*dq4*dqr6*cos(q5)*sin(q2)*sin(q4)*sin(q6))/400 + (29*dq4*dqr6*cos(q6)*sin(q2)*sin(q4)*sin(q5))/200 - (21*dq6*dqr6*cos(q6)*sin(q2)*sin(q3)*sin(q4))/4000 + (29*dq5*dqr6*cos(q5)*sin(q2)*sin(q4)*sin(q6))/200 + (29*dq5*dqr6*cos(q6)*sin(q2)*sin(q4)*sin(q5))/100 + (29*dq6*dqr6*cos(q5)*sin(q2)*sin(q4)*sin(q6))/100 + (29*dq6*dqr6*cos(q6)*sin(q2)*sin(q4)*sin(q5))/200 + (333*dq1*dqr5*sin(2*q2)*sin(2*q3)*sin(2*q5)*cos(q6))/32000 + (111*dq4*dqr5*sin(2*q5)*cos(q2)*cos(q3)*cos(q6))/8000 + dq4*dqr6*sin(q2)*sin(q3)*sin(q6)*((1923*3^(1/2))/80000 + 259/16000) + (37*3^(1/2)*dq2*dqr6*cos(q6)*sin(q2)*sin(q3)*sin(q4))/4000 - (7*3^(1/2)*dq2*dqr6*cos(q5)*sin(q2)*sin(q3)*sin(q6))/4000 - (7*3^(1/2)*dq2*dqr6*cos(q6)*sin(q2)*sin(q3)*sin(q5))/2000 - (37*3^(1/2)*dq3*dqr6*cos(q6)*sin(q2)*sin(q3)*sin(q4))/4000 + (7*3^(1/2)*dq3*dqr6*cos(q5)*sin(q2)*sin(q3)*sin(q6))/4000 + (7*3^(1/2)*dq3*dqr6*cos(q6)*sin(q2)*sin(q3)*sin(q5))/2000 - (37*3^(1/2)*dq5*dqr6*cos(q3)*sin(q2)*sin(q4)*sin(q6))/4000 - (37*3^(1/2)*dq6*dqr6*cos(q3)*sin(q2)*sin(q4)*sin(q6))/2000 + (7*dq2*dqr6*cos(q3)*cos(q4)*sin(q2)*sin(q5)*sin(q6))/2000 + (7*dq2*dqr6*cos(q3)*cos(q5)*sin(q2)*sin(q4)*sin(q6))/4000 + (7*dq2*dqr6*cos(q3)*cos(q6)*sin(q2)*sin(q4)*sin(q5))/2000 - (7*dq3*dqr6*cos(q3)*cos(q4)*sin(q2)*sin(q5)*sin(q6))/2000 - (7*dq3*dqr6*cos(q3)*cos(q5)*sin(q2)*sin(q4)*sin(q6))/4000 - (7*dq3*dqr6*cos(q3)*cos(q6)*sin(q2)*sin(q4)*sin(q5))/2000 - (877*dq4*dqr6*cos(q3)*cos(q4)*sin(q2)*sin(q5)*sin(q6))/8000 - (877*dq4*dqr6*cos(q3)*cos(q6)*sin(q2)*sin(q4)*sin(q5))/8000 - (7*dq4*dqr6*cos(q4)*cos(q5)*sin(q2)*sin(q3)*sin(q6))/4000 - (7*dq4*dqr6*cos(q4)*cos(q6)*sin(q2)*sin(q3)*sin(q5))/2000 - (7*dq4*dqr6*cos(q5)*cos(q6)*sin(q2)*sin(q3)*sin(q4))/1000 - (877*dq5*dqr6*cos(q3)*cos(q5)*sin(q2)*sin(q4)*sin(q6))/8000 - (877*dq5*dqr6*cos(q3)*cos(q6)*sin(q2)*sin(q4)*sin(q5))/4000 - (7*dq5*dqr6*cos(q4)*cos(q5)*sin(q2)*sin(q3)*sin(q6))/2000 - (7*dq5*dqr6*cos(q4)*cos(q6)*sin(q2)*sin(q3)*sin(q5))/1000 - (7*dq5*dqr6*cos(q5)*cos(q6)*sin(q2)*sin(q3)*sin(q4))/2000 - (877*dq6*dqr6*cos(q3)*cos(q5)*sin(q2)*sin(q4)*sin(q6))/4000 - (7*dq6*dqr6*cos(q4)*cos(q5)*sin(q2)*sin(q3)*sin(q6))/1000 - (7*dq6*dqr6*cos(q4)*cos(q6)*sin(q2)*sin(q3)*sin(q5))/2000 - (7*dq6*dqr6*cos(q5)*cos(q6)*sin(q2)*sin(q3)*sin(q4))/4000 + (7*dq4*dqr6*sin(q2)*sin(q3)*sin(q4)*sin(q5)*sin(q6))/2000 + (7*dq5*dqr6*sin(q2)*sin(q3)*sin(q4)*sin(q5)*sin(q6))/4000 + (7*dq6*dqr6*sin(q2)*sin(q3)*sin(q4)*sin(q5)*sin(q6))/2000 - (29*dq1*dqr5*sin(2*q2)*cos(q3)*cos(q4)*cos(q5)*cos(q6))/400 + dq5*dqr6*cos(q6)*sin(q2)*sin(q3)*sin(q5)*((641*3^(1/2))/20000 + 37/1000) + dq6*dqr6*cos(q5)*sin(q2)*sin(q3)*sin(q6)*((641*3^(1/2))/20000 + 37/1000) - dq4*dqr6*cos(q3)*sin(q2)*sin(q4)*sin(q6)*((37*3^(1/2))/16000 + 2631/16000) + dq6*dqr6*cos(q6)*sin(q2)*sin(q3)*sin(q5)*((641*3^(1/2))/40000 + 37/800) + dq4*dqr6*cos(q6)*sin(q2)*sin(q3)*sin(q5)*((641*3^(1/2))/40000 + 37/2000) + dq5*dqr6*cos(q5)*sin(q2)*sin(q3)*sin(q6)*((641*3^(1/2))/40000 + 37/2000) - dq2*dqr6*cos(q3)*sin(q2)*sin(q5)*sin(q6)*((641*3^(1/2))/80000 + 37/1600) + dq3*dqr6*cos(q3)*sin(q2)*sin(q5)*sin(q6)*((641*3^(1/2))/80000 + 37/1600) - dq2*dqr6*cos(q4)*sin(q2)*sin(q3)*sin(q6)*((37*3^(1/2))/3200 + 1923/80000) + dq3*dqr6*cos(q4)*sin(q2)*sin(q3)*sin(q6)*((37*3^(1/2))/3200 + 1923/80000) + dq4*dqr6*cos(q5)*sin(q2)*sin(q3)*sin(q6)*((641*3^(1/2))/80000 - 37/8000) + (37*dq1*dqr5*cos(2*q2)*cos(2*q3)*cos(2*q4)*sin(2*q5)*cos(q6))/6400 + (37*dq1*dqr5*cos(2*q2)*cos(2*q3)*cos(2*q5)*sin(2*q4)*cos(q6))/8000 + (37*dq1*dqr5*cos(2*q4)*sin(2*q2)*sin(2*q3)*sin(2*q5)*cos(q6))/6400 + (37*dq1*dqr5*cos(2*q5)*sin(2*q2)*sin(2*q3)*sin(2*q4)*cos(q6))/8000 + dq1*dqr5*cos(2*q2)*sin(2*q3)*cos(q4)*cos(q5)*cos(q6)*((37*3^(1/2))/8000 - 877/16000) - dq1*dqr5*cos(2*q3)*sin(2*q2)*cos(q4)*cos(q5)*cos(q6)*((37*3^(1/2))/8000 - 877/16000) - (37*3^(1/2)*dq2*dqr6*cos(2*q5)*cos(q4)*sin(q2)*sin(q3)*sin(q6))/16000 - (37*3^(1/2)*dq2*dqr6*cos(2*q5)*cos(q6)*sin(q2)*sin(q3)*sin(q4))/4000 - (37*3^(1/2)*dq2*dqr6*sin(2*q5)*cos(q4)*cos(q6)*sin(q2)*sin(q3))/8000 + (37*3^(1/2)*dq3*dqr6*cos(2*q5)*cos(q4)*sin(q2)*sin(q3)*sin(q6))/16000 + (37*3^(1/2)*dq3*dqr6*cos(2*q5)*cos(q6)*sin(q2)*sin(q3)*sin(q4))/4000 + (37*3^(1/2)*dq3*dqr6*sin(2*q5)*cos(q4)*cos(q6)*sin(q2)*sin(q3))/8000 - (37*3^(1/2)*dq4*dqr6*cos(2*q5)*cos(q3)*sin(q2)*sin(q4)*sin(q6))/16000 - (37*3^(1/2)*dq4*dqr6*sin(2*q5)*cos(q3)*cos(q6)*sin(q2)*sin(q4))/8000 + (37*3^(1/2)*dq2*dqr6*sin(2*q5)*sin(q2)*sin(q3)*sin(q4)*sin(q6))/8000 - (37*3^(1/2)*dq3*dqr6*sin(2*q5)*sin(q2)*sin(q3)*sin(q4)*sin(q6))/8000 - dq1*dqr5*cos(2*q2)*cos(2*q3)*sin(2*q4)*cos(q5)*cos(q6)*((641*3^(1/2))/160000 - 37/16000) - dq6*dqr6*cos(q3)*cos(q6)*sin(q2)*sin(q4)*sin(q5)*((37*3^(1/2))/4000 + 877/8000) - dq6*dqr6*cos(q3)*cos(q4)*sin(q2)*sin(q5)*sin(q6)*((37*3^(1/2))/2000 + 1577/10000) - dq4*dqr6*cos(q3)*cos(q5)*sin(q2)*sin(q4)*sin(q6)*((111*3^(1/2))/8000 + 877/16000) - dq5*dqr6*cos(q3)*cos(q4)*sin(q2)*sin(q5)*sin(q6)*((37*3^(1/2))/4000 + 1577/20000) + dq2*dqr6*cos(q4)*cos(q6)*sin(q2)*sin(q3)*sin(q5)*((37*3^(1/2))/2000 + 1923/40000) - dq3*dqr6*cos(q4)*cos(q6)*sin(q2)*sin(q3)*sin(q5)*((37*3^(1/2))/2000 + 1923/40000) + dq2*dqr6*cos(q4)*cos(q5)*sin(q2)*sin(q3)*sin(q6)*((111*3^(1/2))/8000 + 1923/80000) - dq3*dqr6*cos(q4)*cos(q5)*sin(q2)*sin(q3)*sin(q6)*((111*3^(1/2))/8000 + 1923/80000) - dq1*dqr5*sin(2*q2)*sin(2*q3)*sin(2*q4)*cos(q5)*cos(q6)*((641*3^(1/2))/160000 - 37/16000) - (37*3^(1/2)*dq1*dqr5*cos(2*q2)*cos(2*q5)*sin(2*q3)*cos(q4)*cos(q6))/4000 + (37*3^(1/2)*dq1*dqr5*cos(2*q3)*cos(2*q5)*sin(2*q2)*cos(q4)*cos(q6))/4000 - dq2*dqr6*cos(2*q4)*cos(q3)*sin(q2)*sin(q5)*sin(q6)*((641*3^(1/2))/80000 - 37/8000) + dq3*dqr6*cos(2*q4)*cos(q3)*sin(q2)*sin(q5)*sin(q6)*((641*3^(1/2))/80000 - 37/8000) - (37*3^(1/2)*dq2*dqr6*sin(q2)*sin(q3)*sin(q4)*sin(q5)*sin(q6))/4000 + (37*3^(1/2)*dq3*dqr6*sin(q2)*sin(q3)*sin(q4)*sin(q5)*sin(q6))/4000;
Y1_10_17=(37*dq3*dqr6*cos(q3)*cos(q6)*sin(q2))/4000 - (37*dq2*dqr6*cos(q3)*cos(q6)*sin(q2))/4000 - (87*dq6*dqr6*cos(q4)*cos(q6)*sin(q2))/400 + (87*dq1*dqr6*sin(q3)*sin(q4)*sin(q6))/800 - (87*dq1*dqr6*cos(2*q2)*sin(q3)*sin(q4)*sin(q6))/800 + (7*3^(1/2)*dq6*dqr6*cos(q3)*cos(q6)*sin(q2))/4000 - (29*dq4*dqr6*cos(q4)*cos(q5)*cos(q6)*sin(q2))/100 - (29*dq5*dqr6*cos(q4)*cos(q5)*cos(q6)*sin(q2))/200 - (29*dq6*dqr6*cos(q4)*cos(q5)*cos(q6)*sin(q2))/400 + (29*3^(1/2)*dq1*dqr6*sin(2*q2)*sin(q3)*sin(q6))/800 - (21*dq2*dqr6*cos(q2)*sin(q3)*sin(q4)*sin(q6))/4000 + (21*dq3*dqr6*cos(q2)*sin(q3)*sin(q4)*sin(q6))/4000 + (29*dq1*dqr6*cos(q4)*sin(q3)*sin(q5)*sin(q6))/400 + (29*dq1*dqr6*cos(q5)*sin(q3)*sin(q4)*sin(q6))/800 + (29*dq1*dqr6*cos(q6)*sin(q3)*sin(q4)*sin(q5))/400 + (29*dq4*dqr6*cos(q4)*sin(q2)*sin(q5)*sin(q6))/200 + (29*dq5*dqr6*cos(q4)*sin(q2)*sin(q5)*sin(q6))/400 + (29*dq6*dqr6*cos(q4)*sin(q2)*sin(q5)*sin(q6))/200 + (37*3^(1/2)*dq5*dqr6*cos(q2)*sin(q3)*sin(q4)*sin(q6))/4000 - (7*3^(1/2)*dq5*dqr6*cos(q2)*sin(q3)*sin(q5)*sin(q6))/4000 + (7*3^(1/2)*dq5*dqr6*cos(q3)*sin(q2)*sin(q5)*sin(q6))/4000 + (37*3^(1/2)*dq6*dqr6*cos(q2)*sin(q3)*sin(q4)*sin(q6))/2000 - (7*3^(1/2)*dq6*dqr6*cos(q2)*sin(q3)*sin(q5)*sin(q6))/2000 + (7*3^(1/2)*dq6*dqr6*cos(q3)*sin(q2)*sin(q5)*sin(q6))/2000 - (37*dq2*dqr6*cos(2*q4)*cos(2*q5)*cos(q3)*cos(q6)*sin(q2))/4000 + (37*dq3*dqr6*cos(2*q4)*cos(2*q5)*cos(q3)*cos(q6)*sin(q2))/4000 + dq2*dqr6*sin(2*q4)*cos(q2)*sin(q3)*sin(q6)*((1923*3^(1/2))/160000 + 111/6400) - dq2*dqr6*sin(2*q4)*cos(q3)*sin(q2)*sin(q6)*((1923*3^(1/2))/160000 + 111/6400) - dq3*dqr6*sin(2*q4)*cos(q2)*sin(q3)*sin(q6)*((1923*3^(1/2))/160000 + 111/6400) + dq3*dqr6*sin(2*q4)*cos(q3)*sin(q2)*sin(q6)*((1923*3^(1/2))/160000 + 111/6400) - (37*dq2*dqr6*cos(2*q4)*sin(2*q5)*cos(q2)*sin(q3)*sin(q6))/8000 + (37*dq2*dqr6*cos(2*q4)*sin(2*q5)*cos(q3)*sin(q2)*sin(q6))/8000 - (37*dq2*dqr6*cos(2*q5)*sin(2*q4)*cos(q2)*sin(q3)*sin(q6))/6400 + (37*dq2*dqr6*cos(2*q5)*sin(2*q4)*cos(q3)*sin(q2)*sin(q6))/6400 + (37*dq2*dqr6*sin(2*q4)*sin(2*q5)*cos(q3)*cos(q6)*sin(q2))/3200 + (37*dq3*dqr6*cos(2*q4)*sin(2*q5)*cos(q2)*sin(q3)*sin(q6))/8000 - (37*dq3*dqr6*cos(2*q4)*sin(2*q5)*cos(q3)*sin(q2)*sin(q6))/8000 + (37*dq3*dqr6*cos(2*q5)*sin(2*q4)*cos(q2)*sin(q3)*sin(q6))/6400 - (37*dq3*dqr6*cos(2*q5)*sin(2*q4)*cos(q3)*sin(q2)*sin(q6))/6400 - (37*dq3*dqr6*sin(2*q4)*sin(2*q5)*cos(q3)*cos(q6)*sin(q2))/3200 + (7*dq2*dqr6*cos(q2)*cos(q4)*cos(q5)*cos(q6)*sin(q3))/1000 - (7*dq2*dqr6*cos(q3)*cos(q4)*cos(q5)*cos(q6)*sin(q2))/1000 - (7*dq3*dqr6*cos(q2)*cos(q4)*cos(q5)*cos(q6)*sin(q3))/1000 + (7*dq3*dqr6*cos(q3)*cos(q4)*cos(q5)*cos(q6)*sin(q2))/1000 - (877*dq4*dqr6*cos(q2)*cos(q4)*cos(q5)*cos(q6)*sin(q3))/4000 + (877*dq4*dqr6*cos(q3)*cos(q4)*cos(q5)*cos(q6)*sin(q2))/4000 - (29*3^(1/2)*dq1*dqr6*sin(2*q2)*cos(q5)*sin(q3)*sin(q6))/800 - (29*3^(1/2)*dq1*dqr6*sin(2*q2)*cos(q6)*sin(q3)*sin(q5))/400 - (7*dq2*dqr6*cos(q2)*cos(q4)*sin(q3)*sin(q5)*sin(q6))/2000 - (7*dq2*dqr6*cos(q2)*cos(q5)*sin(q3)*sin(q4)*sin(q6))/4000 - (7*dq2*dqr6*cos(q2)*cos(q6)*sin(q3)*sin(q4)*sin(q5))/2000 + (7*dq3*dqr6*cos(q2)*cos(q4)*sin(q3)*sin(q5)*sin(q6))/2000 + (7*dq3*dqr6*cos(q2)*cos(q5)*sin(q3)*sin(q4)*sin(q6))/4000 + (7*dq3*dqr6*cos(q2)*cos(q6)*sin(q3)*sin(q4)*sin(q5))/2000 + (877*dq4*dqr6*cos(q2)*cos(q4)*sin(q3)*sin(q5)*sin(q6))/8000 + (877*dq4*dqr6*cos(q2)*cos(q6)*sin(q3)*sin(q4)*sin(q5))/8000 + (877*dq5*dqr6*cos(q2)*cos(q5)*sin(q3)*sin(q4)*sin(q6))/8000 + (877*dq5*dqr6*cos(q2)*cos(q6)*sin(q3)*sin(q4)*sin(q5))/4000 + (877*dq6*dqr6*cos(q2)*cos(q5)*sin(q3)*sin(q4)*sin(q6))/4000 + dq6*dqr6*cos(q2)*cos(q4)*cos(q6)*sin(q3)*((37*3^(1/2))/4000 - 351/2500) - dq6*dqr6*cos(q3)*cos(q4)*cos(q6)*sin(q2)*((37*3^(1/2))/4000 - 351/2500) + dq2*dqr6*cos(q3)*cos(q5)*cos(q6)*sin(q2)*((641*3^(1/2))/40000 + 37/2000) - dq3*dqr6*cos(q3)*cos(q5)*cos(q6)*sin(q2)*((641*3^(1/2))/40000 + 37/2000) + dq4*dqr6*cos(q2)*sin(q3)*sin(q4)*sin(q6)*((37*3^(1/2))/16000 + 2631/16000) + dq2*dqr6*cos(q2)*sin(q3)*sin(q5)*sin(q6)*((641*3^(1/2))/80000 + 37/1600) - dq3*dqr6*cos(q2)*sin(q3)*sin(q5)*sin(q6)*((641*3^(1/2))/80000 + 37/1600) - (29*dq1*dqr6*cos(2*q2)*cos(q4)*sin(q3)*sin(q5)*sin(q6))/400 - (29*dq1*dqr6*cos(2*q2)*cos(q5)*sin(q3)*sin(q4)*sin(q6))/800 - (29*dq1*dqr6*cos(2*q2)*cos(q6)*sin(q3)*sin(q4)*sin(q5))/400 - (37*3^(1/2)*dq4*dqr6*cos(q2)*cos(q4)*cos(q6)*sin(q3))/4000 + (37*3^(1/2)*dq4*dqr6*cos(q3)*cos(q4)*cos(q6)*sin(q2))/4000 - (7*3^(1/2)*dq5*dqr6*cos(q3)*cos(q5)*cos(q6)*sin(q2))/2000 - (7*3^(1/2)*dq6*dqr6*cos(q3)*cos(q5)*cos(q6)*sin(q2))/4000 - (37*3^(1/2)*dq4*dqr6*cos(2*q5)*cos(q2)*cos(q4)*cos(q6)*sin(q3))/4000 + (37*3^(1/2)*dq4*dqr6*cos(2*q5)*cos(q3)*cos(q4)*cos(q6)*sin(q2))/4000 + (37*3^(1/2)*dq4*dqr6*cos(2*q5)*cos(q2)*sin(q3)*sin(q4)*sin(q6))/16000 + (37*3^(1/2)*dq4*dqr6*sin(2*q5)*cos(q2)*cos(q4)*sin(q3)*sin(q6))/8000 + (37*3^(1/2)*dq4*dqr6*sin(2*q5)*cos(q2)*cos(q6)*sin(q3)*sin(q4))/8000 - (37*3^(1/2)*dq4*dqr6*sin(2*q5)*cos(q3)*cos(q4)*sin(q2)*sin(q6))/8000 - dq5*dqr6*cos(q2)*cos(q4)*cos(q5)*cos(q6)*sin(q3)*((37*3^(1/2))/2000 + 1577/10000) + dq5*dqr6*cos(q3)*cos(q4)*cos(q5)*cos(q6)*sin(q2)*((37*3^(1/2))/2000 + 1577/10000) - dq6*dqr6*cos(q2)*cos(q4)*cos(q5)*cos(q6)*sin(q3)*((111*3^(1/2))/4000 + 1577/20000) + dq6*dqr6*cos(q3)*cos(q4)*cos(q5)*cos(q6)*sin(q2)*((111*3^(1/2))/4000 + 1577/20000) + dq6*dqr6*cos(q2)*cos(q6)*sin(q3)*sin(q4)*sin(q5)*((37*3^(1/2))/4000 + 877/8000) + dq6*dqr6*cos(q2)*cos(q4)*sin(q3)*sin(q5)*sin(q6)*((37*3^(1/2))/2000 + 1577/10000) + dq4*dqr6*cos(q2)*cos(q5)*sin(q3)*sin(q4)*sin(q6)*((111*3^(1/2))/8000 + 877/16000) + dq5*dqr6*cos(q2)*cos(q4)*sin(q3)*sin(q5)*sin(q6)*((37*3^(1/2))/4000 + 1577/20000) - dq2*dqr6*cos(2*q4)*cos(q2)*cos(q5)*cos(q6)*sin(q3)*((641*3^(1/2))/40000 + 37/2000) + dq2*dqr6*cos(2*q4)*cos(q3)*cos(q5)*cos(q6)*sin(q2)*((641*3^(1/2))/40000 + 37/2000) - dq3*dqr6*cos(2*q4)*cos(q3)*cos(q5)*cos(q6)*sin(q2)*((641*3^(1/2))/40000 + 37/2000) + dq2*dqr6*sin(2*q4)*cos(q2)*cos(q6)*sin(q3)*sin(q5)*((641*3^(1/2))/80000 + 37/4000) - dq2*dqr6*sin(2*q4)*cos(q3)*cos(q6)*sin(q2)*sin(q5)*((641*3^(1/2))/80000 + 37/4000) - dq3*dqr6*sin(2*q4)*cos(q2)*cos(q6)*sin(q3)*sin(q5)*((641*3^(1/2))/80000 + 37/4000) + dq3*dqr6*sin(2*q4)*cos(q3)*cos(q6)*sin(q2)*sin(q5)*((641*3^(1/2))/80000 + 37/4000) + dq2*dqr6*cos(2*q4)*cos(q2)*sin(q3)*sin(q5)*sin(q6)*((641*3^(1/2))/80000 - 37/8000) - dq3*dqr6*cos(2*q4)*cos(q2)*sin(q3)*sin(q5)*sin(q6)*((641*3^(1/2))/80000 - 37/8000) + dq2*dqr6*sin(2*q4)*cos(q2)*cos(q5)*sin(q3)*sin(q6)*((641*3^(1/2))/160000 - 37/16000) - dq2*dqr6*sin(2*q4)*cos(q3)*cos(q5)*sin(q2)*sin(q6)*((641*3^(1/2))/160000 - 37/16000) - dq3*dqr6*sin(2*q4)*cos(q2)*cos(q5)*sin(q3)*sin(q6)*((641*3^(1/2))/160000 - 37/16000) + dq3*dqr6*sin(2*q4)*cos(q3)*cos(q5)*sin(q2)*sin(q6)*((641*3^(1/2))/160000 - 37/16000);
Y1_10_18=(37*dq2*dqr6*cos(q2)*cos(q6)*sin(q3))/4000 - (29*3^(1/2)*dq1*dqr6*cos(q3)*sin(q6))/800 - (21*dq1*dqr6*cos(q4)*sin(q6))/4000 - (37*dq3*dqr6*cos(q2)*cos(q6)*sin(q3))/4000 - (7*dq1*dqr6*cos(q4)*cos(q5)*sin(q6))/4000 - (7*dq1*dqr6*cos(q4)*cos(q6)*sin(q5))/2000 - (7*dq1*dqr6*cos(q5)*cos(q6)*sin(q4))/1000 - (37*dq5*dqr6*cos(q2)*cos(q3)*sin(q6))/4000 - (37*dq6*dqr6*cos(q2)*cos(q3)*sin(q6))/2000 + (7*dq1*dqr6*sin(q4)*sin(q5)*sin(q6))/2000 - dq1*dqr6*cos(q6)*sin(q5)*((6847*3^(1/2))/160000 - 111/8000) + (87*dq1*dqr6*sin(2*q2)*cos(q3)*sin(q4)*sin(q6))/800 + (7*3^(1/2)*dq2*dqr6*cos(q2)*cos(q3)*sin(q6))/4000 - (7*3^(1/2)*dq3*dqr6*cos(q2)*cos(q3)*sin(q6))/4000 + (29*3^(1/2)*dq1*dqr6*cos(q3)*cos(q5)*sin(q6))/800 + (29*3^(1/2)*dq1*dqr6*cos(q3)*cos(q6)*sin(q5))/400 - (7*3^(1/2)*dq6*dqr6*cos(q2)*cos(q6)*sin(q3))/4000 + dq1*dqr6*cos(2*q4)*cos(q6)*sin(q5)*((641*3^(1/2))/160000 + 37/8000) - dq1*dqr6*sin(2*q4)*sin(q5)*sin(q6)*((641*3^(1/2))/160000 - 37/16000) + (29*3^(1/2)*dq1*dqr6*cos(2*q2)*cos(q3)*sin(q6))/800 - (29*dq1*dqr6*cos(q4)*cos(q5)*cos(q6)*sin(q3))/200 - (21*dq4*dqr6*cos(q2)*cos(q3)*cos(q4)*sin(q6))/4000 - (21*dq6*dqr6*cos(q2)*cos(q3)*cos(q6)*sin(q4))/4000 + dq4*dqr6*cos(q2)*cos(q3)*sin(q6)*((1923*3^(1/2))/80000 + 259/16000) + (111*dq4*dqr6*cos(2*q5)*cos(q2)*cos(q3)*sin(q6))/16000 + (37*dq2*dqr6*cos(2*q4)*cos(2*q5)*cos(q2)*cos(q6)*sin(q3))/4000 - (37*dq3*dqr6*cos(2*q4)*cos(2*q5)*cos(q2)*cos(q6)*sin(q3))/4000 + (1231*dq1*dqr6*cos(2*q2)*sin(2*q3)*cos(q5)*sin(q4)*sin(q6))/80000 - (1231*dq1*dqr6*cos(2*q3)*sin(2*q2)*cos(q5)*sin(q4)*sin(q6))/80000 - (37*dq2*dqr6*sin(2*q4)*sin(2*q5)*cos(q2)*cos(q6)*sin(q3))/3200 + (37*dq3*dqr6*sin(2*q4)*sin(2*q5)*cos(q2)*cos(q6)*sin(q3))/3200 - (29*3^(1/2)*dq1*dqr6*cos(2*q2)*cos(q3)*cos(q5)*sin(q6))/800 - (29*3^(1/2)*dq1*dqr6*cos(2*q2)*cos(q3)*cos(q6)*sin(q5))/400 - (7*dq4*dqr6*cos(q2)*cos(q3)*cos(q4)*cos(q5)*sin(q6))/4000 - (7*dq4*dqr6*cos(q2)*cos(q3)*cos(q4)*cos(q6)*sin(q5))/2000 - (7*dq4*dqr6*cos(q2)*cos(q3)*cos(q5)*cos(q6)*sin(q4))/1000 - (7*dq5*dqr6*cos(q2)*cos(q3)*cos(q4)*cos(q5)*sin(q6))/2000 - (7*dq5*dqr6*cos(q2)*cos(q3)*cos(q4)*cos(q6)*sin(q5))/1000 - (7*dq5*dqr6*cos(q2)*cos(q3)*cos(q5)*cos(q6)*sin(q4))/2000 - (7*dq6*dqr6*cos(q2)*cos(q3)*cos(q4)*cos(q5)*sin(q6))/1000 - (7*dq6*dqr6*cos(q2)*cos(q3)*cos(q4)*cos(q6)*sin(q5))/2000 - (7*dq6*dqr6*cos(q2)*cos(q3)*cos(q5)*cos(q6)*sin(q4))/4000 + dq1*dqr6*cos(2*q2)*cos(2*q3)*cos(q6)*sin(q5)*((9411*3^(1/2))/160000 + 37/8000) + (7*dq4*dqr6*cos(q2)*cos(q3)*sin(q4)*sin(q5)*sin(q6))/2000 + (7*dq5*dqr6*cos(q2)*cos(q3)*sin(q4)*sin(q5)*sin(q6))/4000 + (7*dq6*dqr6*cos(q2)*cos(q3)*sin(q4)*sin(q5)*sin(q6))/2000 + dq1*dqr6*cos(2*q2)*sin(2*q3)*sin(q4)*sin(q6)*((111*3^(1/2))/16000 + 7539/80000) - dq1*dqr6*cos(2*q3)*sin(2*q2)*sin(q4)*sin(q6)*((111*3^(1/2))/16000 + 7539/80000) + dq1*dqr6*sin(2*q2)*sin(2*q3)*cos(q6)*sin(q5)*((9411*3^(1/2))/160000 + 37/8000) + dq1*dqr6*sin(2*q2)*sin(2*q3)*cos(q5)*sin(q6)*((9411*3^(1/2))/320000 - 259/32000) + dq5*dqr6*cos(q2)*cos(q3)*cos(q6)*sin(q5)*((641*3^(1/2))/20000 + 37/1000) + dq6*dqr6*cos(q2)*cos(q3)*cos(q5)*sin(q6)*((641*3^(1/2))/20000 + 37/1000) + dq6*dqr6*cos(q2)*cos(q3)*cos(q6)*sin(q5)*((641*3^(1/2))/40000 + 37/800) - dq2*dqr6*cos(q2)*cos(q5)*cos(q6)*sin(q3)*((641*3^(1/2))/40000 + 37/2000) + dq3*dqr6*cos(q2)*cos(q5)*cos(q6)*sin(q3)*((641*3^(1/2))/40000 + 37/2000) + dq4*dqr6*cos(q2)*cos(q3)*cos(q6)*sin(q5)*((641*3^(1/2))/40000 + 37/2000) + dq5*dqr6*cos(q2)*cos(q3)*cos(q5)*sin(q6)*((641*3^(1/2))/40000 + 37/2000) - dq2*dqr6*cos(q2)*cos(q3)*cos(q4)*sin(q6)*((37*3^(1/2))/3200 + 1923/80000) + dq3*dqr6*cos(q2)*cos(q3)*cos(q4)*sin(q6)*((37*3^(1/2))/3200 + 1923/80000) + dq4*dqr6*cos(q2)*cos(q3)*cos(q5)*sin(q6)*((641*3^(1/2))/80000 - 37/8000) + (29*dq1*dqr6*cos(2*q2)*cos(q4)*cos(q5)*cos(q6)*sin(q3))/200 + (29*dq1*dqr6*sin(2*q2)*cos(q3)*cos(q4)*sin(q5)*sin(q6))/400 + (29*dq1*dqr6*sin(2*q2)*cos(q3)*cos(q5)*sin(q4)*sin(q6))/800 + (29*dq1*dqr6*sin(2*q2)*cos(q3)*cos(q6)*sin(q4)*sin(q5))/400 + (37*3^(1/2)*dq2*dqr6*cos(q2)*cos(q3)*cos(q6)*sin(q4))/4000 - (7*3^(1/2)*dq2*dqr6*cos(q2)*cos(q3)*cos(q5)*sin(q6))/4000 - (7*3^(1/2)*dq2*dqr6*cos(q2)*cos(q3)*cos(q6)*sin(q5))/2000 - (37*3^(1/2)*dq3*dqr6*cos(q2)*cos(q3)*cos(q6)*sin(q4))/4000 + (7*3^(1/2)*dq3*dqr6*cos(q2)*cos(q3)*cos(q5)*sin(q6))/4000 + (7*3^(1/2)*dq3*dqr6*cos(q2)*cos(q3)*cos(q6)*sin(q5))/2000 + (7*3^(1/2)*dq5*dqr6*cos(q2)*cos(q5)*cos(q6)*sin(q3))/2000 + (7*3^(1/2)*dq6*dqr6*cos(q2)*cos(q5)*cos(q6)*sin(q3))/4000 - (37*3^(1/2)*dq2*dqr6*cos(2*q5)*cos(q2)*cos(q3)*cos(q4)*sin(q6))/16000 - (37*3^(1/2)*dq2*dqr6*cos(2*q5)*cos(q2)*cos(q3)*cos(q6)*sin(q4))/4000 + (37*3^(1/2)*dq3*dqr6*cos(2*q5)*cos(q2)*cos(q3)*cos(q4)*sin(q6))/16000 + (37*3^(1/2)*dq3*dqr6*cos(2*q5)*cos(q2)*cos(q3)*cos(q6)*sin(q4))/4000 + (37*3^(1/2)*dq2*dqr6*sin(2*q5)*cos(q2)*cos(q3)*sin(q4)*sin(q6))/8000 - (37*3^(1/2)*dq3*dqr6*sin(2*q5)*cos(q2)*cos(q3)*sin(q4)*sin(q6))/8000 - dq1*dqr6*cos(2*q2)*sin(2*q3)*cos(q4)*sin(q5)*sin(q6)*((37*3^(1/2))/8000 - 877/16000) + dq1*dqr6*cos(2*q3)*sin(2*q2)*cos(q4)*sin(q5)*sin(q6)*((37*3^(1/2))/8000 - 877/16000) - dq1*dqr6*cos(2*q2)*sin(2*q3)*cos(q6)*sin(q4)*sin(q5)*((37*3^(1/2))/4000 - 1231/40000) + dq1*dqr6*cos(2*q3)*sin(2*q2)*cos(q6)*sin(q4)*sin(q5)*((37*3^(1/2))/4000 - 1231/40000) + dq2*dqr6*cos(q2)*cos(q3)*cos(q4)*cos(q6)*sin(q5)*((37*3^(1/2))/2000 + 1923/40000) - dq3*dqr6*cos(q2)*cos(q3)*cos(q4)*cos(q6)*sin(q5)*((37*3^(1/2))/2000 + 1923/40000) + dq2*dqr6*cos(q2)*cos(q3)*cos(q4)*cos(q5)*sin(q6)*((111*3^(1/2))/8000 + 1923/80000) - dq3*dqr6*cos(q2)*cos(q3)*cos(q4)*cos(q5)*sin(q6)*((111*3^(1/2))/8000 + 1923/80000) - dq1*dqr6*cos(2*q2)*cos(2*q3)*cos(2*q4)*cos(q6)*sin(q5)*((641*3^(1/2))/160000 + 37/8000) - dq1*dqr6*cos(2*q4)*sin(2*q2)*sin(2*q3)*cos(q6)*sin(q5)*((641*3^(1/2))/160000 + 37/8000) + dq1*dqr6*cos(2*q2)*cos(2*q3)*sin(2*q4)*sin(q5)*sin(q6)*((641*3^(1/2))/160000 - 37/16000) - dq1*dqr6*cos(2*q4)*sin(2*q2)*sin(2*q3)*cos(q5)*sin(q6)*((641*3^(1/2))/320000 - 37/32000) + dq1*dqr6*sin(2*q2)*sin(2*q3)*sin(2*q4)*sin(q5)*sin(q6)*((641*3^(1/2))/160000 - 37/16000) + dq3*dqr6*cos(2*q4)*cos(q2)*cos(q5)*cos(q6)*sin(q3)*((641*3^(1/2))/40000 + 37/2000) - (37*3^(1/2)*dq2*dqr6*cos(q2)*cos(q3)*sin(q4)*sin(q5)*sin(q6))/4000 + (37*3^(1/2)*dq3*dqr6*cos(q2)*cos(q3)*sin(q4)*sin(q5)*sin(q6))/4000 + (37*3^(1/2)*dq1*dqr6*cos(2*q2)*cos(2*q5)*sin(2*q3)*sin(q4)*sin(q6))/16000 + (37*3^(1/2)*dq1*dqr6*cos(2*q2)*sin(2*q3)*sin(2*q5)*cos(q4)*sin(q6))/8000 + (37*3^(1/2)*dq1*dqr6*cos(2*q2)*sin(2*q3)*sin(2*q5)*cos(q6)*sin(q4))/8000 - (37*3^(1/2)*dq1*dqr6*cos(2*q3)*cos(2*q5)*sin(2*q2)*sin(q4)*sin(q6))/16000 - (37*3^(1/2)*dq1*dqr6*cos(2*q3)*sin(2*q2)*sin(2*q5)*cos(q4)*sin(q6))/8000 - (37*3^(1/2)*dq1*dqr6*cos(2*q3)*sin(2*q2)*sin(2*q5)*cos(q6)*sin(q4))/8000;
Y1_10_19=dq1*dqr6*sin(q6)*((14539*3^(1/2))/320000 + 111/12800) + (111*dq1*dqr6*cos(2*q5)*sin(q6))/64000 + (111*dq1*dqr6*sin(2*q5)*cos(q6))/32000 + (37*ddqr5*cos(q6)*sin(q2)*sin(q3))/2000 + (37*ddqr6*cos(q6)*sin(q2)*sin(q3))/2000 - (21*ddqr2*cos(q3)*cos(q6)*sin(q2)*sin(q4))/4000 + (21*ddqr4*cos(q4)*cos(q6)*sin(q2)*sin(q3))/4000 + (29*ddqr4*sin(q2)*sin(q4)*sin(q5)*sin(q6))/200 - (21*ddqr6*sin(q2)*sin(q3)*sin(q4)*sin(q6))/4000 + (29*ddqr5*sin(q2)*sin(q4)*sin(q5)*sin(q6))/100 + (29*ddqr6*sin(q2)*sin(q4)*sin(q5)*sin(q6))/200 + dq1*dqr6*cos(2*q4)*sin(q6)*((1923*3^(1/2))/320000 + 111/12800) - (37*dq1*dqr6*cos(2*q4)*cos(2*q5)*sin(q6))/12800 - (37*dq1*dqr6*cos(2*q4)*sin(2*q5)*cos(q6))/6400 - (37*dq1*dqr6*cos(2*q5)*sin(2*q4)*cos(q6))/8000 - ddqr4*cos(q6)*sin(q2)*sin(q3)*((1923*3^(1/2))/40000 + 259/8000) + (37*dq1*dqr6*sin(2*q4)*sin(2*q5)*sin(q6))/16000 - (111*ddqr4*cos(2*q5)*cos(q6)*sin(q2)*sin(q3))/8000 + (111*ddqr4*sin(2*q5)*sin(q2)*sin(q3)*sin(q6))/4000 - (7*3^(1/2)*ddqr2*cos(q6)*sin(q2)*sin(q3))/4000 + (7*3^(1/2)*ddqr3*cos(q6)*sin(q2)*sin(q3))/4000 - dq1*dqr6*cos(q5)*sin(q6)*((6847*3^(1/2))/320000 - 111/32000) - (7*ddqr2*cos(q3)*cos(q5)*cos(q6)*sin(q2)*sin(q4))/4000 + (1231*ddqr2*cos(q4)*cos(q5)*cos(q6)*sin(q2)*sin(q3))/40000 + (7*ddqr3*cos(q3)*cos(q5)*cos(q6)*sin(q2)*sin(q4))/4000 - (1231*ddqr3*cos(q4)*cos(q5)*cos(q6)*sin(q2)*sin(q3))/40000 + (7*ddqr4*cos(q4)*cos(q5)*cos(q6)*sin(q2)*sin(q3))/4000 + (7*ddqr5*cos(q4)*cos(q5)*cos(q6)*sin(q2)*sin(q3))/2000 + (7*ddqr6*cos(q4)*cos(q5)*cos(q6)*sin(q2)*sin(q3))/1000 + (7*ddqr2*cos(q3)*sin(q2)*sin(q4)*sin(q5)*sin(q6))/2000 - (877*ddqr2*cos(q5)*sin(q2)*sin(q3)*sin(q4)*sin(q6))/4000 - (7*ddqr3*cos(q3)*sin(q2)*sin(q4)*sin(q5)*sin(q6))/2000 + (877*ddqr3*cos(q5)*sin(q2)*sin(q3)*sin(q4)*sin(q6))/4000 - (7*ddqr4*cos(q4)*sin(q2)*sin(q3)*sin(q5)*sin(q6))/2000 - (7*ddqr4*cos(q5)*sin(q2)*sin(q3)*sin(q4)*sin(q6))/1000 - (7*ddqr4*cos(q6)*sin(q2)*sin(q3)*sin(q4)*sin(q5))/2000 - (877*ddqr5*cos(q3)*sin(q2)*sin(q4)*sin(q5)*sin(q6))/4000 - (7*ddqr5*cos(q4)*sin(q2)*sin(q3)*sin(q5)*sin(q6))/1000 - (7*ddqr5*cos(q5)*sin(q2)*sin(q3)*sin(q4)*sin(q6))/2000 - (7*ddqr5*cos(q6)*sin(q2)*sin(q3)*sin(q4)*sin(q5))/4000 - (7*ddqr6*cos(q4)*sin(q2)*sin(q3)*sin(q5)*sin(q6))/2000 - (7*ddqr6*cos(q5)*sin(q2)*sin(q3)*sin(q4)*sin(q6))/4000 - (7*ddqr6*cos(q6)*sin(q2)*sin(q3)*sin(q4)*sin(q5))/2000 + dq1*dqr6*sin(2*q4)*cos(q5)*cos(q6)*((641*3^(1/2))/80000 + 37/4000) + dq1*dqr6*cos(2*q4)*cos(q5)*sin(q6)*((641*3^(1/2))/320000 - 37/32000) - ddqr6*cos(q5)*cos(q6)*sin(q2)*sin(q3)*((641*3^(1/2))/20000 + 37/1000) - ddqr4*cos(q5)*cos(q6)*sin(q2)*sin(q3)*((641*3^(1/2))/40000 - 37/4000) - ddqr5*cos(q5)*cos(q6)*sin(q2)*sin(q3)*((641*3^(1/2))/40000 - 37/4000) + ddqr2*cos(q4)*cos(q6)*sin(q2)*sin(q3)*((111*3^(1/2))/8000 + 7539/40000) - ddqr3*cos(q4)*cos(q6)*sin(q2)*sin(q3)*((111*3^(1/2))/8000 + 7539/40000) + ddqr4*sin(q2)*sin(q3)*sin(q5)*sin(q6)*((641*3^(1/2))/20000 + 37/1000) + ddqr5*sin(q2)*sin(q3)*sin(q5)*sin(q6)*((641*3^(1/2))/20000 + 37/1000) + ddqr6*sin(q2)*sin(q3)*sin(q5)*sin(q6)*((641*3^(1/2))/40000 + 37/800) - dq1*dqr6*cos(2*q2)*cos(2*q3)*sin(q6)*((6847*3^(1/2))/320000 - 481/64000) + (7*3^(1/2)*ddqr2*cos(q5)*cos(q6)*sin(q2)*sin(q3))/4000 - (7*3^(1/2)*ddqr3*cos(q5)*cos(q6)*sin(q2)*sin(q3))/4000 + (333*dq1*dqr6*cos(2*q2)*cos(2*q3)*cos(2*q5)*sin(q6))/64000 + (333*dq1*dqr6*cos(2*q2)*cos(2*q3)*sin(2*q5)*cos(q6))/32000 - dq1*dqr6*sin(2*q2)*sin(2*q3)*sin(q6)*((6847*3^(1/2))/320000 - 481/64000) - (7*3^(1/2)*ddqr2*sin(q2)*sin(q3)*sin(q5)*sin(q6))/2000 + (7*3^(1/2)*ddqr3*sin(q2)*sin(q3)*sin(q5)*sin(q6))/2000 + (333*dq1*dqr6*cos(2*q5)*sin(2*q2)*sin(2*q3)*sin(q6))/64000 + (333*dq1*dqr6*sin(2*q2)*sin(2*q3)*sin(2*q5)*cos(q6))/32000 + (111*dq4*dqr6*sin(2*q5)*cos(q2)*cos(q3)*cos(q6))/8000 - (37*dq1*dqr6*sin(2*q2)*sin(2*q3)*sin(2*q4)*sin(2*q5)*sin(q6))/16000 - (877*dq1*dqr6*cos(2*q2)*sin(2*q3)*cos(q4)*cos(q5)*cos(q6))/8000 + (877*dq1*dqr6*cos(2*q3)*sin(2*q2)*cos(q4)*cos(q5)*cos(q6))/8000 + ddqr2*cos(q6)*sin(q2)*sin(q3)*sin(q4)*sin(q5)*((37*3^(1/2))/4000 - 877/8000) - ddqr3*cos(q6)*sin(q2)*sin(q3)*sin(q4)*sin(q5)*((37*3^(1/2))/4000 - 877/8000) - ddqr6*cos(q3)*sin(q2)*sin(q4)*sin(q5)*sin(q6)*((37*3^(1/2))/4000 + 877/8000) + ddqr2*cos(q4)*sin(q2)*sin(q3)*sin(q5)*sin(q6)*((37*3^(1/2))/2000 - 1231/20000) - ddqr3*cos(q4)*sin(q2)*sin(q3)*sin(q5)*sin(q6)*((37*3^(1/2))/2000 - 1231/20000) + ddqr4*cos(q3)*sin(q2)*sin(q4)*sin(q5)*sin(q6)*((37*3^(1/2))/2000 - 1231/20000) + dq1*dqr6*cos(2*q2)*cos(2*q3)*cos(q5)*sin(q6)*((9411*3^(1/2))/320000 - 259/32000) - (29*dq1*dqr6*sin(2*q2)*cos(q3)*cos(q4)*cos(q5)*cos(q6))/200 - dq1*dqr6*cos(2*q2)*cos(2*q3)*cos(2*q4)*sin(q6)*((1923*3^(1/2))/320000 + 111/12800) + (37*3^(1/2)*ddqr2*cos(2*q5)*cos(q4)*cos(q6)*sin(q2)*sin(q3))/8000 - (37*3^(1/2)*ddqr3*cos(2*q5)*cos(q4)*cos(q6)*sin(q2)*sin(q3))/8000 + (37*dq1*dqr6*cos(2*q2)*cos(2*q3)*cos(2*q4)*cos(2*q5)*sin(q6))/12800 + (37*dq1*dqr6*cos(2*q2)*cos(2*q3)*cos(2*q4)*sin(2*q5)*cos(q6))/6400 + (37*dq1*dqr6*cos(2*q2)*cos(2*q3)*cos(2*q5)*sin(2*q4)*cos(q6))/8000 - dq1*dqr6*cos(2*q4)*sin(2*q2)*sin(2*q3)*sin(q6)*((1923*3^(1/2))/320000 + 111/12800) - (37*3^(1/2)*ddqr2*cos(2*q5)*sin(q2)*sin(q3)*sin(q4)*sin(q6))/2000 - (37*3^(1/2)*ddqr2*sin(2*q5)*cos(q4)*sin(q2)*sin(q3)*sin(q6))/4000 - (37*3^(1/2)*ddqr2*sin(2*q5)*cos(q6)*sin(q2)*sin(q3)*sin(q4))/4000 + (37*3^(1/2)*ddqr3*cos(2*q5)*sin(q2)*sin(q3)*sin(q4)*sin(q6))/2000 + (37*3^(1/2)*ddqr3*sin(2*q5)*cos(q4)*sin(q2)*sin(q3)*sin(q6))/4000 + (37*3^(1/2)*ddqr3*sin(2*q5)*cos(q6)*sin(q2)*sin(q3)*sin(q4))/4000 - (37*3^(1/2)*ddqr4*sin(2*q5)*cos(q3)*sin(q2)*sin(q4)*sin(q6))/4000 - (37*dq1*dqr6*cos(2*q2)*cos(2*q3)*sin(2*q4)*sin(2*q5)*sin(q6))/16000 + (37*dq1*dqr6*cos(2*q4)*cos(2*q5)*sin(2*q2)*sin(2*q3)*sin(q6))/12800 + (37*dq1*dqr6*cos(2*q4)*sin(2*q2)*sin(2*q3)*sin(2*q5)*cos(q6))/6400 + (37*dq1*dqr6*cos(2*q5)*sin(2*q2)*sin(2*q3)*sin(2*q4)*cos(q6))/8000 - (37*3^(1/2)*dq2*dqr6*sin(2*q5)*cos(q2)*cos(q3)*cos(q4)*cos(q6))/8000 + (37*3^(1/2)*dq3*dqr6*sin(2*q5)*cos(q2)*cos(q3)*cos(q4)*cos(q6))/8000 - dq1*dqr6*cos(2*q2)*cos(2*q3)*sin(2*q4)*cos(q5)*cos(q6)*((641*3^(1/2))/80000 + 37/4000) - dq1*dqr6*cos(2*q2)*cos(2*q3)*cos(2*q4)*cos(q5)*sin(q6)*((641*3^(1/2))/320000 - 37/32000) - dq1*dqr6*sin(2*q2)*sin(2*q3)*sin(2*q4)*cos(q5)*cos(q6)*((641*3^(1/2))/80000 + 37/4000) - (37*3^(1/2)*dq1*dqr6*cos(2*q2)*cos(2*q5)*sin(2*q3)*cos(q4)*cos(q6))/4000 + (37*3^(1/2)*dq1*dqr6*cos(2*q3)*cos(2*q5)*sin(2*q2)*cos(q4)*cos(q6))/4000;
Y1_10_20=(21*ddqr2*cos(q2)*cos(q6)*sin(q3)*sin(q4))/4000 - (87*ddqr4*cos(q6)*sin(q2)*sin(q4))/400 - (87*ddqr6*cos(q4)*sin(q2)*sin(q6))/400 - (29*3^(1/2)*ddqr1*sin(2*q2)*cos(q6)*sin(q3))/400 - (87*ddqr1*cos(q6)*sin(q3)*sin(q4))/400 - (21*ddqr3*cos(q2)*cos(q6)*sin(q3)*sin(q4))/4000 + (21*ddqr3*cos(q3)*cos(q6)*sin(q2)*sin(q4))/4000 - (29*ddqr1*cos(q4)*cos(q5)*sin(q3)*sin(q6))/100 - (29*ddqr1*cos(q4)*cos(q6)*sin(q3)*sin(q5))/200 - (29*ddqr1*cos(q5)*cos(q6)*sin(q3)*sin(q4))/400 - (29*ddqr4*cos(q4)*cos(q5)*sin(q2)*sin(q6))/100 - (29*ddqr4*cos(q4)*cos(q6)*sin(q2)*sin(q5))/200 - (29*ddqr4*cos(q5)*cos(q6)*sin(q2)*sin(q4))/400 - (29*ddqr5*cos(q4)*cos(q5)*sin(q2)*sin(q6))/200 - (29*ddqr5*cos(q4)*cos(q6)*sin(q2)*sin(q5))/400 - (29*ddqr5*cos(q5)*cos(q6)*sin(q2)*sin(q4))/200 - (29*ddqr6*cos(q4)*cos(q5)*sin(q2)*sin(q6))/400 - (29*ddqr6*cos(q4)*cos(q6)*sin(q2)*sin(q5))/200 - (29*ddqr6*cos(q5)*cos(q6)*sin(q2)*sin(q4))/100 + (29*ddqr1*sin(q3)*sin(q4)*sin(q5)*sin(q6))/200 + (87*ddqr1*cos(2*q2)*cos(q6)*sin(q3)*sin(q4))/400 + (7*3^(1/2)*ddqr6*cos(q3)*sin(q2)*sin(q6))/4000 + (7*ddqr2*cos(q2)*cos(q4)*cos(q5)*sin(q3)*sin(q6))/1000 + (7*ddqr2*cos(q2)*cos(q4)*cos(q6)*sin(q3)*sin(q5))/2000 + (7*ddqr2*cos(q2)*cos(q5)*cos(q6)*sin(q3)*sin(q4))/4000 - (7*ddqr2*cos(q3)*cos(q4)*cos(q5)*sin(q2)*sin(q6))/1000 - (7*ddqr2*cos(q3)*cos(q4)*cos(q6)*sin(q2)*sin(q5))/2000 - (7*ddqr3*cos(q2)*cos(q4)*cos(q6)*sin(q3)*sin(q5))/2000 - (7*ddqr3*cos(q2)*cos(q5)*cos(q6)*sin(q3)*sin(q4))/4000 + (7*ddqr3*cos(q3)*cos(q4)*cos(q5)*sin(q2)*sin(q6))/1000 + (7*ddqr3*cos(q3)*cos(q4)*cos(q6)*sin(q2)*sin(q5))/2000 - (1231*ddqr4*cos(q2)*cos(q5)*cos(q6)*sin(q3)*sin(q4))/40000 + (877*ddqr4*cos(q3)*cos(q4)*cos(q5)*sin(q2)*sin(q6))/4000 + (1231*ddqr4*cos(q3)*cos(q5)*cos(q6)*sin(q2)*sin(q4))/40000 - (877*ddqr6*cos(q2)*cos(q5)*cos(q6)*sin(q3)*sin(q4))/4000 + (877*ddqr6*cos(q3)*cos(q5)*cos(q6)*sin(q2)*sin(q4))/4000 - (29*3^(1/2)*ddqr1*sin(2*q2)*sin(q3)*sin(q5)*sin(q6))/200 - (7*ddqr2*cos(q2)*sin(q3)*sin(q4)*sin(q5)*sin(q6))/2000 + (7*ddqr3*cos(q2)*sin(q3)*sin(q4)*sin(q5)*sin(q6))/2000 + (877*ddqr5*cos(q2)*sin(q3)*sin(q4)*sin(q5)*sin(q6))/4000 - ddqr6*cos(q3)*cos(q4)*sin(q2)*sin(q6)*((37*3^(1/2))/4000 - 351/2500) - ddqr4*cos(q2)*cos(q6)*sin(q3)*sin(q4)*((111*3^(1/2))/8000 + 7539/40000) + ddqr4*cos(q3)*cos(q6)*sin(q2)*sin(q4)*((111*3^(1/2))/8000 + 7539/40000) + (29*ddqr1*cos(2*q2)*cos(q4)*cos(q5)*sin(q3)*sin(q6))/100 + (29*ddqr1*cos(2*q2)*cos(q4)*cos(q6)*sin(q3)*sin(q5))/200 + (29*ddqr1*cos(2*q2)*cos(q5)*cos(q6)*sin(q3)*sin(q4))/400 - (29*ddqr1*cos(2*q2)*sin(q3)*sin(q4)*sin(q5)*sin(q6))/200 - (37*3^(1/2)*ddqr5*cos(q2)*cos(q6)*sin(q3)*sin(q4))/2000 + (37*3^(1/2)*ddqr5*cos(q3)*cos(q6)*sin(q2)*sin(q4))/2000 + (7*3^(1/2)*ddqr5*cos(q2)*cos(q6)*sin(q3)*sin(q5))/4000 - (7*3^(1/2)*ddqr5*cos(q3)*cos(q5)*sin(q2)*sin(q6))/2000 - (7*3^(1/2)*ddqr5*cos(q3)*cos(q6)*sin(q2)*sin(q5))/4000 - (37*3^(1/2)*ddqr6*cos(q2)*cos(q6)*sin(q3)*sin(q4))/2000 + (37*3^(1/2)*ddqr6*cos(q3)*cos(q6)*sin(q2)*sin(q4))/2000 + (7*3^(1/2)*ddqr6*cos(q2)*cos(q6)*sin(q3)*sin(q5))/2000 - (7*3^(1/2)*ddqr6*cos(q3)*cos(q5)*sin(q2)*sin(q6))/4000 - (7*3^(1/2)*ddqr6*cos(q3)*cos(q6)*sin(q2)*sin(q5))/2000 + ddqr2*sin(2*q4)*cos(q3)*cos(q6)*sin(q2)*((1923*3^(1/2))/80000 + 111/3200) - ddqr3*sin(2*q4)*cos(q3)*cos(q6)*sin(q2)*((1923*3^(1/2))/80000 + 111/3200) + (37*ddqr2*cos(2*q4)*cos(2*q5)*cos(q2)*sin(q3)*sin(q6))/2000 - (37*ddqr2*cos(2*q4)*cos(2*q5)*cos(q3)*sin(q2)*sin(q6))/2000 - (37*ddqr2*cos(2*q4)*sin(2*q5)*cos(q3)*cos(q6)*sin(q2))/4000 - (37*ddqr2*cos(2*q5)*sin(2*q4)*cos(q3)*cos(q6)*sin(q2))/3200 + (37*ddqr3*cos(2*q4)*cos(2*q5)*cos(q3)*sin(q2)*sin(q6))/2000 + (37*ddqr3*cos(2*q4)*sin(2*q5)*cos(q3)*cos(q6)*sin(q2))/4000 + (37*ddqr3*cos(2*q5)*sin(2*q4)*cos(q3)*cos(q6)*sin(q2))/3200 - (37*ddqr2*sin(2*q4)*sin(2*q5)*cos(q2)*sin(q3)*sin(q6))/1600 + (37*ddqr2*sin(2*q4)*sin(2*q5)*cos(q3)*sin(q2)*sin(q6))/1600 - (37*ddqr3*sin(2*q4)*sin(2*q5)*cos(q3)*sin(q2)*sin(q6))/1600 + (29*3^(1/2)*ddqr1*sin(2*q2)*cos(q5)*cos(q6)*sin(q3))/400 + ddqr4*cos(q2)*cos(q4)*cos(q6)*sin(q3)*sin(q5)*((37*3^(1/2))/4000 - 877/8000) - ddqr4*cos(q3)*cos(q4)*cos(q6)*sin(q2)*sin(q5)*((37*3^(1/2))/4000 - 877/8000) + ddqr5*cos(q2)*cos(q5)*cos(q6)*sin(q3)*sin(q4)*((37*3^(1/2))/4000 - 877/8000) - ddqr5*cos(q3)*cos(q5)*cos(q6)*sin(q2)*sin(q4)*((37*3^(1/2))/4000 - 877/8000) + ddqr5*cos(q3)*cos(q4)*cos(q5)*sin(q2)*sin(q6)*((37*3^(1/2))/2000 + 1577/10000) - ddqr6*cos(q2)*cos(q4)*cos(q6)*sin(q3)*sin(q5)*((37*3^(1/2))/2000 + 1577/10000) + ddqr6*cos(q3)*cos(q4)*cos(q6)*sin(q2)*sin(q5)*((37*3^(1/2))/2000 + 1577/10000) + ddqr5*cos(q2)*cos(q4)*cos(q6)*sin(q3)*sin(q5)*((37*3^(1/2))/4000 - 1577/20000) - ddqr5*cos(q3)*cos(q4)*cos(q6)*sin(q2)*sin(q5)*((37*3^(1/2))/4000 - 1577/20000) + ddqr6*cos(q3)*cos(q4)*cos(q5)*sin(q2)*sin(q6)*((111*3^(1/2))/4000 + 1577/20000) + ddqr6*cos(q2)*sin(q3)*sin(q4)*sin(q5)*sin(q6)*((37*3^(1/2))/4000 + 877/8000) - ddqr4*cos(q2)*sin(q3)*sin(q4)*sin(q5)*sin(q6)*((37*3^(1/2))/2000 - 1231/20000) - ddqr2*cos(2*q4)*cos(q2)*cos(q5)*sin(q3)*sin(q6)*((641*3^(1/2))/20000 + 37/1000) + ddqr2*cos(2*q4)*cos(q3)*cos(q5)*sin(q2)*sin(q6)*((641*3^(1/2))/20000 + 37/1000) - ddqr3*cos(2*q4)*cos(q3)*cos(q5)*sin(q2)*sin(q6)*((641*3^(1/2))/20000 + 37/1000) - ddqr2*cos(2*q4)*cos(q2)*cos(q6)*sin(q3)*sin(q5)*((641*3^(1/2))/40000 - 37/4000) + ddqr2*cos(2*q4)*cos(q3)*cos(q6)*sin(q2)*sin(q5)*((641*3^(1/2))/40000 - 37/4000) + ddqr3*cos(2*q4)*cos(q2)*cos(q6)*sin(q3)*sin(q5)*((641*3^(1/2))/40000 - 37/4000) - ddqr3*cos(2*q4)*cos(q3)*cos(q6)*sin(q2)*sin(q5)*((641*3^(1/2))/40000 - 37/4000) + ddqr2*sin(2*q4)*cos(q3)*cos(q5)*cos(q6)*sin(q2)*((641*3^(1/2))/80000 - 37/8000) - ddqr3*sin(2*q4)*cos(q3)*cos(q5)*cos(q6)*sin(q2)*((641*3^(1/2))/80000 - 37/8000) + ddqr2*sin(2*q4)*cos(q2)*sin(q3)*sin(q5)*sin(q6)*((641*3^(1/2))/40000 + 37/2000) - ddqr2*sin(2*q4)*cos(q3)*sin(q2)*sin(q5)*sin(q6)*((641*3^(1/2))/40000 + 37/2000) - ddqr3*sin(2*q4)*cos(q2)*sin(q3)*sin(q5)*sin(q6)*((641*3^(1/2))/40000 + 37/2000) + ddqr3*sin(2*q4)*cos(q3)*sin(q2)*sin(q5)*sin(q6)*((641*3^(1/2))/40000 + 37/2000) - (37*3^(1/2)*ddqr4*cos(2*q5)*cos(q2)*cos(q6)*sin(q3)*sin(q4))/8000 + (37*3^(1/2)*ddqr4*cos(2*q5)*cos(q3)*cos(q4)*sin(q2)*sin(q6))/2000 + (37*3^(1/2)*ddqr4*cos(2*q5)*cos(q3)*cos(q6)*sin(q2)*sin(q4))/8000 + (37*3^(1/2)*ddqr4*sin(2*q5)*cos(q3)*cos(q4)*cos(q6)*sin(q2))/4000 + (37*3^(1/2)*ddqr4*sin(2*q5)*cos(q2)*sin(q3)*sin(q4)*sin(q6))/4000;
Y1_10_21=(111*ddqr1*sin(2*q5)*sin(q6))/16000 - (37*ddqr1*cos(2*q4)*sin(2*q5)*sin(q6))/3200 - (37*ddqr1*cos(2*q5)*sin(2*q4)*sin(q6))/4000 - (7*ddqr1*cos(q4)*sin(q5)*sin(q6))/1000 - (7*ddqr1*cos(q5)*sin(q4)*sin(q6))/500 - (7*ddqr1*cos(q6)*sin(q4)*sin(q5))/1000 - ddqr1*sin(q5)*sin(q6)*((6847*3^(1/2))/80000 - 111/4000) + (29*3^(1/2)*ddqr1*cos(q3)*cos(q6))/400 + (29*ddqr2*cos(q2)*cos(q4)*sin(q5)*sin(q6))/200 + (29*ddqr2*cos(q2)*cos(q5)*sin(q4)*sin(q6))/100 + (29*ddqr2*cos(q2)*cos(q6)*sin(q4)*sin(q5))/200 - (21*ddqr6*cos(q2)*cos(q3)*sin(q4)*sin(q6))/4000 + (333*ddqr1*cos(2*q2)*cos(2*q3)*sin(2*q5)*sin(q6))/16000 + (333*ddqr1*sin(2*q2)*sin(2*q3)*sin(2*q5)*sin(q6))/16000 - (87*ddqr1*sin(2*q2)*cos(q3)*cos(q6)*sin(q4))/400 - (29*3^(1/2)*ddqr1*cos(q3)*cos(q5)*cos(q6))/400 + (29*3^(1/2)*ddqr1*cos(q3)*sin(q5)*sin(q6))/200 - (7*3^(1/2)*ddqr6*cos(q2)*sin(q3)*sin(q6))/4000 + ddqr1*sin(2*q4)*cos(q5)*sin(q6)*((641*3^(1/2))/40000 + 37/2000) + ddqr1*cos(2*q4)*sin(q5)*sin(q6)*((641*3^(1/2))/80000 + 37/4000) + ddqr1*sin(2*q4)*cos(q6)*sin(q5)*((641*3^(1/2))/80000 - 37/8000) - (29*3^(1/2)*ddqr1*cos(2*q2)*cos(q3)*cos(q6))/400 - (877*ddqr2*cos(q2)*cos(q3)*cos(q5)*sin(q4)*sin(q6))/4000 + (877*ddqr3*cos(q2)*cos(q3)*cos(q5)*sin(q4)*sin(q6))/4000 - (7*ddqr3*cos(q2)*cos(q4)*cos(q5)*sin(q3)*sin(q6))/1000 - (7*ddqr4*cos(q2)*cos(q3)*cos(q4)*sin(q5)*sin(q6))/2000 - (7*ddqr4*cos(q2)*cos(q3)*cos(q5)*sin(q4)*sin(q6))/1000 - (7*ddqr4*cos(q2)*cos(q3)*cos(q6)*sin(q4)*sin(q5))/2000 - (877*ddqr4*cos(q2)*cos(q4)*cos(q5)*sin(q3)*sin(q6))/4000 - (7*ddqr5*cos(q2)*cos(q3)*cos(q4)*sin(q5)*sin(q6))/1000 - (7*ddqr5*cos(q2)*cos(q3)*cos(q5)*sin(q4)*sin(q6))/2000 - (7*ddqr5*cos(q2)*cos(q3)*cos(q6)*sin(q4)*sin(q5))/4000 - (7*ddqr6*cos(q2)*cos(q3)*cos(q4)*sin(q5)*sin(q6))/2000 - (7*ddqr6*cos(q2)*cos(q3)*cos(q5)*sin(q4)*sin(q6))/4000 - (7*ddqr6*cos(q2)*cos(q3)*cos(q6)*sin(q4)*sin(q5))/2000 - ddqr1*cos(2*q2)*sin(2*q3)*cos(q6)*sin(q4)*((111*3^(1/2))/8000 + 7539/40000) + ddqr1*cos(2*q3)*sin(2*q2)*cos(q6)*sin(q4)*((111*3^(1/2))/8000 + 7539/40000) + ddqr1*cos(2*q2)*cos(2*q3)*sin(q5)*sin(q6)*((9411*3^(1/2))/80000 + 37/4000) + ddqr1*sin(2*q2)*sin(2*q3)*sin(q5)*sin(q6)*((9411*3^(1/2))/80000 + 37/4000) + ddqr6*cos(q2)*cos(q4)*sin(q3)*sin(q6)*((37*3^(1/2))/4000 - 351/2500) + ddqr4*cos(q2)*cos(q3)*sin(q5)*sin(q6)*((641*3^(1/2))/20000 + 37/1000) + ddqr5*cos(q2)*cos(q3)*sin(q5)*sin(q6)*((641*3^(1/2))/20000 + 37/1000) + ddqr6*cos(q2)*cos(q3)*sin(q5)*sin(q6)*((641*3^(1/2))/40000 + 37/800) - (29*ddqr1*sin(2*q2)*cos(q3)*cos(q4)*cos(q5)*sin(q6))/100 - (29*ddqr1*sin(2*q2)*cos(q3)*cos(q4)*cos(q6)*sin(q5))/200 - (29*ddqr1*sin(2*q2)*cos(q3)*cos(q5)*cos(q6)*sin(q4))/400 + (37*ddqr1*cos(2*q2)*cos(2*q3)*cos(2*q4)*sin(2*q5)*sin(q6))/3200 + (37*ddqr1*cos(2*q2)*cos(2*q3)*cos(2*q5)*sin(2*q4)*sin(q6))/4000 + (29*ddqr1*sin(2*q2)*cos(q3)*sin(q4)*sin(q5)*sin(q6))/200 - (7*3^(1/2)*ddqr2*cos(q2)*cos(q3)*sin(q5)*sin(q6))/2000 + (7*3^(1/2)*ddqr3*cos(q2)*cos(q3)*sin(q5)*sin(q6))/2000 + (7*3^(1/2)*ddqr5*cos(q2)*cos(q5)*sin(q3)*sin(q6))/2000 + (7*3^(1/2)*ddqr6*cos(q2)*cos(q5)*sin(q3)*sin(q6))/4000 + (37*ddqr1*cos(2*q4)*sin(2*q2)*sin(2*q3)*sin(2*q5)*sin(q6))/3200 + (37*ddqr1*cos(2*q5)*sin(2*q2)*sin(2*q3)*sin(2*q4)*sin(q6))/4000 - ddqr2*sin(2*q4)*cos(q2)*cos(q6)*sin(q3)*((1923*3^(1/2))/80000 + 111/3200) + ddqr3*sin(2*q4)*cos(q2)*cos(q6)*sin(q3)*((1923*3^(1/2))/80000 + 111/3200) - (877*ddqr1*cos(2*q2)*sin(2*q3)*cos(q4)*cos(q5)*sin(q6))/4000 - (1231*ddqr1*cos(2*q2)*sin(2*q3)*cos(q5)*cos(q6)*sin(q4))/40000 + (877*ddqr1*cos(2*q3)*sin(2*q2)*cos(q4)*cos(q5)*sin(q6))/4000 + (1231*ddqr1*cos(2*q3)*sin(2*q2)*cos(q5)*cos(q6)*sin(q4))/40000 + (37*ddqr2*cos(2*q4)*sin(2*q5)*cos(q2)*cos(q6)*sin(q3))/4000 + (37*ddqr2*cos(2*q5)*sin(2*q4)*cos(q2)*cos(q6)*sin(q3))/3200 - (37*ddqr3*cos(2*q4)*cos(2*q5)*cos(q2)*sin(q3)*sin(q6))/2000 - (37*ddqr3*cos(2*q4)*sin(2*q5)*cos(q2)*cos(q6)*sin(q3))/4000 - (37*ddqr3*cos(2*q5)*sin(2*q4)*cos(q2)*cos(q6)*sin(q3))/3200 + (29*3^(1/2)*ddqr1*cos(2*q2)*cos(q3)*cos(q5)*cos(q6))/400 + (37*ddqr3*sin(2*q4)*sin(2*q5)*cos(q2)*sin(q3)*sin(q6))/1600 - (29*3^(1/2)*ddqr1*cos(2*q2)*cos(q3)*sin(q5)*sin(q6))/200 - ddqr1*cos(2*q2)*sin(2*q3)*sin(q4)*sin(q5)*sin(q6)*((37*3^(1/2))/2000 - 1231/20000) + ddqr1*cos(2*q3)*sin(2*q2)*sin(q4)*sin(q5)*sin(q6)*((37*3^(1/2))/2000 - 1231/20000) + ddqr2*cos(q2)*cos(q3)*cos(q6)*sin(q4)*sin(q5)*((37*3^(1/2))/4000 - 877/8000) - ddqr3*cos(q2)*cos(q3)*cos(q6)*sin(q4)*sin(q5)*((37*3^(1/2))/4000 - 877/8000) - ddqr5*cos(q2)*cos(q4)*cos(q5)*sin(q3)*sin(q6)*((37*3^(1/2))/2000 + 1577/10000) + ddqr2*cos(q2)*cos(q3)*cos(q4)*sin(q5)*sin(q6)*((37*3^(1/2))/2000 - 1231/20000) - ddqr3*cos(q2)*cos(q3)*cos(q4)*sin(q5)*sin(q6)*((37*3^(1/2))/2000 - 1231/20000) - ddqr6*cos(q2)*cos(q4)*cos(q5)*sin(q3)*sin(q6)*((111*3^(1/2))/4000 + 1577/20000) - ddqr1*cos(2*q2)*cos(2*q3)*sin(2*q4)*cos(q5)*sin(q6)*((641*3^(1/2))/40000 + 37/2000) - ddqr1*cos(2*q2)*cos(2*q3)*cos(2*q4)*sin(q5)*sin(q6)*((641*3^(1/2))/80000 + 37/4000) - ddqr1*cos(2*q2)*cos(2*q3)*sin(2*q4)*cos(q6)*sin(q5)*((641*3^(1/2))/80000 - 37/8000) - ddqr1*sin(2*q2)*sin(2*q3)*sin(2*q4)*cos(q5)*sin(q6)*((641*3^(1/2))/40000 + 37/2000) - ddqr1*cos(2*q4)*sin(2*q2)*sin(2*q3)*sin(q5)*sin(q6)*((641*3^(1/2))/80000 + 37/4000) - ddqr1*sin(2*q2)*sin(2*q3)*sin(2*q4)*cos(q6)*sin(q5)*((641*3^(1/2))/80000 - 37/8000) - (37*3^(1/2)*ddqr1*cos(2*q2)*cos(2*q5)*sin(2*q3)*cos(q4)*sin(q6))/2000 - (37*3^(1/2)*ddqr1*cos(2*q2)*cos(2*q5)*sin(2*q3)*cos(q6)*sin(q4))/8000 + (37*3^(1/2)*ddqr1*cos(2*q3)*cos(2*q5)*sin(2*q2)*cos(q4)*sin(q6))/2000 + (37*3^(1/2)*ddqr1*cos(2*q3)*cos(2*q5)*sin(2*q2)*cos(q6)*sin(q4))/8000 + ddqr3*cos(2*q4)*cos(q2)*cos(q5)*sin(q3)*sin(q6)*((641*3^(1/2))/20000 + 37/1000) - ddqr2*sin(2*q4)*cos(q2)*cos(q5)*cos(q6)*sin(q3)*((641*3^(1/2))/80000 - 37/8000) + ddqr3*sin(2*q4)*cos(q2)*cos(q5)*cos(q6)*sin(q3)*((641*3^(1/2))/80000 - 37/8000) + (37*3^(1/2)*ddqr1*cos(2*q2)*sin(2*q3)*sin(2*q5)*sin(q4)*sin(q6))/4000 - (37*3^(1/2)*ddqr1*cos(2*q3)*sin(2*q2)*sin(2*q5)*sin(q4)*sin(q6))/4000 - (37*3^(1/2)*ddqr2*cos(2*q5)*cos(q2)*cos(q3)*sin(q4)*sin(q6))/2000 - (37*3^(1/2)*ddqr2*sin(2*q5)*cos(q2)*cos(q3)*cos(q6)*sin(q4))/4000 + (37*3^(1/2)*ddqr3*cos(2*q5)*cos(q2)*cos(q3)*sin(q4)*sin(q6))/2000 + (37*3^(1/2)*ddqr3*sin(2*q5)*cos(q2)*cos(q3)*cos(q6)*sin(q4))/4000 - (37*3^(1/2)*ddqr4*cos(2*q5)*cos(q2)*cos(q4)*sin(q3)*sin(q6))/2000 - (37*3^(1/2)*ddqr4*sin(2*q5)*cos(q2)*cos(q4)*cos(q6)*sin(q3))/4000 + ddqr1*cos(2*q2)*sin(2*q3)*cos(q4)*cos(q6)*sin(q5)*((37*3^(1/2))/4000 - 877/8000) - ddqr1*cos(2*q3)*sin(2*q2)*cos(q4)*cos(q6)*sin(q5)*((37*3^(1/2))/4000 - 877/8000);
Y1_10_22=(21*ddqr1*cos(q4)*cos(q6))/2000 - ddqr1*cos(q6)*((14539*3^(1/2))/160000 + 111/6400) - (111*ddqr1*cos(2*q5)*cos(q6))/32000 - (37*ddqr1*sin(2*q4)*sin(2*q5)*cos(q6))/8000 - (87*ddqr2*cos(q2)*cos(q4)*cos(q6))/400 + (7*ddqr1*cos(q4)*cos(q5)*cos(q6))/2000 + (37*ddqr5*cos(q2)*cos(q3)*cos(q6))/2000 + (37*ddqr6*cos(q2)*cos(q3)*cos(q6))/2000 + ddqr1*cos(q5)*cos(q6)*((6847*3^(1/2))/160000 - 111/16000) - ddqr1*cos(2*q4)*cos(q6)*((1923*3^(1/2))/160000 + 111/6400) + (37*ddqr1*cos(2*q4)*cos(2*q5)*cos(q6))/6400 - (29*ddqr2*cos(q2)*cos(q4)*cos(q5)*cos(q6))/400 + (21*ddqr4*cos(q2)*cos(q3)*cos(q4)*cos(q6))/4000 + ddqr1*cos(2*q2)*cos(2*q3)*cos(q6)*((6847*3^(1/2))/160000 - 481/32000) - (333*ddqr1*cos(2*q2)*cos(2*q3)*cos(2*q5)*cos(q6))/32000 + ddqr1*sin(2*q2)*sin(2*q3)*cos(q6)*((6847*3^(1/2))/160000 - 481/32000) - (333*ddqr1*cos(2*q5)*sin(2*q2)*sin(2*q3)*cos(q6))/32000 - ddqr4*cos(q2)*cos(q3)*cos(q6)*((1923*3^(1/2))/40000 + 259/8000) - (111*ddqr4*cos(2*q5)*cos(q2)*cos(q3)*cos(q6))/8000 + (111*ddqr4*sin(2*q5)*cos(q2)*cos(q3)*sin(q6))/4000 - (7*3^(1/2)*ddqr2*cos(q2)*cos(q3)*cos(q6))/4000 + (7*3^(1/2)*ddqr3*cos(q2)*cos(q3)*cos(q6))/4000 - ddqr1*cos(2*q4)*cos(q5)*cos(q6)*((641*3^(1/2))/160000 - 37/16000) - ddqr1*sin(2*q2)*sin(2*q3)*cos(q5)*cos(q6)*((9411*3^(1/2))/160000 - 259/16000) - ddqr6*cos(q2)*cos(q3)*cos(q5)*cos(q6)*((641*3^(1/2))/20000 + 37/1000) - ddqr4*cos(q2)*cos(q3)*cos(q5)*cos(q6)*((641*3^(1/2))/40000 - 37/4000) - ddqr5*cos(q2)*cos(q3)*cos(q5)*cos(q6)*((641*3^(1/2))/40000 - 37/4000) + ddqr2*cos(q2)*cos(q3)*cos(q4)*cos(q6)*((111*3^(1/2))/8000 + 7539/40000) - ddqr3*cos(q2)*cos(q3)*cos(q4)*cos(q6)*((111*3^(1/2))/8000 + 7539/40000) + ddqr1*cos(2*q2)*cos(2*q3)*cos(2*q4)*cos(q6)*((1923*3^(1/2))/160000 + 111/6400) - (37*ddqr1*cos(2*q2)*cos(2*q3)*cos(2*q4)*cos(2*q5)*cos(q6))/6400 + ddqr1*cos(2*q4)*sin(2*q2)*sin(2*q3)*cos(q6)*((1923*3^(1/2))/160000 + 111/6400) + (7*3^(1/2)*ddqr2*cos(q2)*cos(q3)*cos(q5)*cos(q6))/4000 - (7*3^(1/2)*ddqr3*cos(q2)*cos(q3)*cos(q5)*cos(q6))/4000 + (37*ddqr1*cos(2*q2)*cos(2*q3)*sin(2*q4)*sin(2*q5)*cos(q6))/8000 - (37*ddqr1*cos(2*q4)*cos(2*q5)*sin(2*q2)*sin(2*q3)*cos(q6))/6400 + (37*ddqr1*sin(2*q2)*sin(2*q3)*sin(2*q4)*sin(2*q5)*cos(q6))/8000 + (1231*ddqr2*cos(q2)*cos(q3)*cos(q4)*cos(q5)*cos(q6))/40000 - (1231*ddqr3*cos(q2)*cos(q3)*cos(q4)*cos(q5)*cos(q6))/40000 + (7*ddqr4*cos(q2)*cos(q3)*cos(q4)*cos(q5)*cos(q6))/4000 + (7*ddqr5*cos(q2)*cos(q3)*cos(q4)*cos(q5)*cos(q6))/2000 + (7*ddqr6*cos(q2)*cos(q3)*cos(q4)*cos(q5)*cos(q6))/1000 - ddqr1*cos(2*q2)*cos(2*q3)*cos(q5)*cos(q6)*((9411*3^(1/2))/160000 - 259/16000) + ddqr1*cos(2*q2)*cos(2*q3)*cos(2*q4)*cos(q5)*cos(q6)*((641*3^(1/2))/160000 - 37/16000) + ddqr1*cos(2*q4)*sin(2*q2)*sin(2*q3)*cos(q5)*cos(q6)*((641*3^(1/2))/160000 - 37/16000) - (37*3^(1/2)*ddqr1*cos(2*q2)*sin(2*q3)*sin(2*q5)*cos(q4)*cos(q6))/4000 + (37*3^(1/2)*ddqr1*cos(2*q3)*sin(2*q2)*sin(2*q5)*cos(q4)*cos(q6))/4000 + (37*3^(1/2)*ddqr2*cos(2*q5)*cos(q2)*cos(q3)*cos(q4)*cos(q6))/8000 - (37*3^(1/2)*ddqr3*cos(2*q5)*cos(q2)*cos(q3)*cos(q4)*cos(q6))/8000 - (37*3^(1/2)*ddqr2*sin(2*q5)*cos(q2)*cos(q3)*cos(q4)*sin(q6))/4000 + (37*3^(1/2)*ddqr3*sin(2*q5)*cos(q2)*cos(q3)*cos(q4)*sin(q6))/4000;
Y1_15_1=ddqr1;
Y1_16_1=ddqr1/2 - (ddqr1*cos(2*q2))/2 + (dq1*dqr2*sin(2*q2))/2 + (dq2*dqr1*sin(2*q2))/2;
Y1_17_1=ddqr1/2 - (ddqr1*cos(2*q2)*cos(2*q3))/2 - (ddqr1*sin(2*q2)*sin(2*q3))/2 - (dq1*dqr2*cos(2*q2)*sin(2*q3))/2 + (dq1*dqr2*cos(2*q3)*sin(2*q2))/2 - (dq2*dqr1*cos(2*q2)*sin(2*q3))/2 + (dq2*dqr1*cos(2*q3)*sin(2*q2))/2 + (dq1*dqr3*cos(2*q2)*sin(2*q3))/2 - (dq1*dqr3*cos(2*q3)*sin(2*q2))/2 + (dq3*dqr1*cos(2*q2)*sin(2*q3))/2 - (dq3*dqr1*cos(2*q3)*sin(2*q2))/2;
Y1_18_1=(3*ddqr1)/4 + (ddqr1*cos(2*q4))/4 + (ddqr1*cos(2*q2)*cos(2*q3))/4 + (ddqr1*sin(2*q2)*sin(2*q3))/4 - (dq1*dqr4*sin(2*q4))/4 - (dq4*dqr1*sin(2*q4))/4 + ddqr4*cos(q2)*cos(q3) + ddqr4*sin(q2)*sin(q3) - (ddqr1*cos(2*q2)*cos(2*q3)*cos(2*q4))/4 - (ddqr1*cos(2*q4)*sin(2*q2)*sin(2*q3))/4 + (dq1*dqr2*cos(2*q2)*sin(2*q3))/4 - (dq1*dqr2*cos(2*q3)*sin(2*q2))/4 + (dq2*dqr1*cos(2*q2)*sin(2*q3))/4 - (dq2*dqr1*cos(2*q3)*sin(2*q2))/4 - (dq1*dqr3*cos(2*q2)*sin(2*q3))/4 + (dq1*dqr3*cos(2*q3)*sin(2*q2))/4 - (dq3*dqr1*cos(2*q2)*sin(2*q3))/4 + (dq3*dqr1*cos(2*q3)*sin(2*q2))/4 + (ddqr2*sin(2*q4)*cos(q2)*sin(q3))/2 - (ddqr2*sin(2*q4)*cos(q3)*sin(q2))/2 - (ddqr3*sin(2*q4)*cos(q2)*sin(q3))/2 + (ddqr3*sin(2*q4)*cos(q3)*sin(q2))/2 + (dq2*dqr4*cos(q2)*sin(q3))/2 - (dq2*dqr4*cos(q3)*sin(q2))/2 + (dq4*dqr2*cos(q2)*sin(q3))/2 - (dq4*dqr2*cos(q3)*sin(q2))/2 - (dq3*dqr4*cos(q2)*sin(q3))/2 + (dq3*dqr4*cos(q3)*sin(q2))/2 - (dq4*dqr3*cos(q2)*sin(q3))/2 + (dq4*dqr3*cos(q3)*sin(q2))/2 - (dq2*dqr2*sin(2*q4)*cos(q2)*cos(q3))/2 + (dq2*dqr3*sin(2*q4)*cos(q2)*cos(q3))/2 + (dq3*dqr2*sin(2*q4)*cos(q2)*cos(q3))/2 + (dq2*dqr4*cos(2*q4)*cos(q2)*sin(q3))/2 - (dq2*dqr4*cos(2*q4)*cos(q3)*sin(q2))/2 - (dq3*dqr3*sin(2*q4)*cos(q2)*cos(q3))/2 + (dq4*dqr2*cos(2*q4)*cos(q2)*sin(q3))/2 - (dq4*dqr2*cos(2*q4)*cos(q3)*sin(q2))/2 - (dq3*dqr4*cos(2*q4)*cos(q2)*sin(q3))/2 + (dq3*dqr4*cos(2*q4)*cos(q3)*sin(q2))/2 - (dq4*dqr3*cos(2*q4)*cos(q2)*sin(q3))/2 + (dq4*dqr3*cos(2*q4)*cos(q3)*sin(q2))/2 - (dq2*dqr2*sin(2*q4)*sin(q2)*sin(q3))/2 + (dq2*dqr3*sin(2*q4)*sin(q2)*sin(q3))/2 + (dq3*dqr2*sin(2*q4)*sin(q2)*sin(q3))/2 - (dq3*dqr3*sin(2*q4)*sin(q2)*sin(q3))/2 - (dq1*dqr2*cos(2*q2)*cos(2*q4)*sin(2*q3))/4 + (dq1*dqr2*cos(2*q3)*cos(2*q4)*sin(2*q2))/4 - (dq2*dqr1*cos(2*q2)*cos(2*q4)*sin(2*q3))/4 + (dq2*dqr1*cos(2*q3)*cos(2*q4)*sin(2*q2))/4 + (dq1*dqr3*cos(2*q2)*cos(2*q4)*sin(2*q3))/4 - (dq1*dqr3*cos(2*q3)*cos(2*q4)*sin(2*q2))/4 + (dq3*dqr1*cos(2*q2)*cos(2*q4)*sin(2*q3))/4 - (dq3*dqr1*cos(2*q3)*cos(2*q4)*sin(2*q2))/4 + (dq1*dqr4*cos(2*q2)*cos(2*q3)*sin(2*q4))/4 + (dq4*dqr1*cos(2*q2)*cos(2*q3)*sin(2*q4))/4 + (dq1*dqr4*sin(2*q2)*sin(2*q3)*sin(2*q4))/4 + (dq4*dqr1*sin(2*q2)*sin(2*q3)*sin(2*q4))/4;
Y1_19_1=(3*dq4*dqr1*sin(2*q4))/32 + (3*dq5*dqr1*sin(2*q5))/32 - (dq2*dqr1*cos(2*q2)*sin(2*q3))/32 + (dq2*dqr1*cos(2*q3)*sin(2*q2))/32 + (dq3*dqr1*cos(2*q2)*sin(2*q3))/32 - (dq3*dqr1*cos(2*q3)*sin(2*q2))/32 - (dq4*dqr1*cos(2*q4)*sin(2*q5))/8 - (5*dq4*dqr1*cos(2*q5)*sin(2*q4))/32 - (5*dq5*dqr1*cos(2*q4)*sin(2*q5))/32 - (dq5*dqr1*cos(2*q5)*sin(2*q4))/8 + (5*dq4*dqr2*cos(q2)*sin(q3))/16 - (5*dq4*dqr2*cos(q3)*sin(q2))/16 + (dq5*dqr2*cos(q2)*sin(q3))/4 - (dq5*dqr2*cos(q3)*sin(q2))/4 - (3*dq4*dqr2*cos(2*q4)*cos(q2)*sin(q3))/16 + (3*dq4*dqr2*cos(2*q4)*cos(q3)*sin(q2))/16 - (3*dq4*dqr2*cos(2*q5)*cos(q2)*sin(q3))/16 + (3*dq4*dqr2*cos(2*q5)*cos(q3)*sin(q2))/16 + (3*dq2*dqr2*sin(2*q4)*sin(q2)*sin(q3))/16 - (3*dq3*dqr2*sin(2*q4)*sin(q2)*sin(q3))/16 + (3*dq2*dqr1*cos(2*q2)*cos(2*q4)*sin(2*q3))/32 - (3*dq2*dqr1*cos(2*q3)*cos(2*q4)*sin(2*q2))/32 - (9*dq2*dqr1*cos(2*q2)*cos(2*q5)*sin(2*q3))/32 + (9*dq2*dqr1*cos(2*q3)*cos(2*q5)*sin(2*q2))/32 - (3*dq3*dqr1*cos(2*q2)*cos(2*q4)*sin(2*q3))/32 + (3*dq3*dqr1*cos(2*q3)*cos(2*q4)*sin(2*q2))/32 + (9*dq3*dqr1*cos(2*q2)*cos(2*q5)*sin(2*q3))/32 - (9*dq3*dqr1*cos(2*q3)*cos(2*q5)*sin(2*q2))/32 - (3*dq4*dqr1*cos(2*q2)*cos(2*q3)*sin(2*q4))/32 + (9*dq5*dqr1*cos(2*q2)*cos(2*q3)*sin(2*q5))/32 - (3*dq4*dqr1*sin(2*q2)*sin(2*q3)*sin(2*q4))/32 + (9*dq5*dqr1*sin(2*q2)*sin(2*q3)*sin(2*q5))/32 - (5*dq2*dqr1*cos(2*q2)*cos(2*q4)*cos(2*q5)*sin(2*q3))/32 + (5*dq2*dqr1*cos(2*q3)*cos(2*q4)*cos(2*q5)*sin(2*q2))/32 + (5*dq3*dqr1*cos(2*q2)*cos(2*q4)*cos(2*q5)*sin(2*q3))/32 - (5*dq3*dqr1*cos(2*q3)*cos(2*q4)*cos(2*q5)*sin(2*q2))/32 + (dq4*dqr1*cos(2*q2)*cos(2*q3)*cos(2*q4)*sin(2*q5))/8 + (5*dq4*dqr1*cos(2*q2)*cos(2*q3)*cos(2*q5)*sin(2*q4))/32 + (5*dq5*dqr1*cos(2*q2)*cos(2*q3)*cos(2*q4)*sin(2*q5))/32 + (dq5*dqr1*cos(2*q2)*cos(2*q3)*cos(2*q5)*sin(2*q4))/8 + (3^(1/2)*dq2*dqr2*cos(q2)*cos(q4)*sin(q3))/8 - (3^(1/2)*dq2*dqr2*cos(q3)*cos(q4)*sin(q2))/8 - (3^(1/2)*dq3*dqr2*cos(q2)*cos(q4)*sin(q3))/8 + (3^(1/2)*dq3*dqr2*cos(q3)*cos(q4)*sin(q2))/8 + (3^(1/2)*dq5*dqr2*cos(q2)*cos(q3)*sin(q4))/4 + (dq2*dqr1*cos(2*q2)*sin(2*q3)*sin(2*q4)*sin(2*q5))/8 - (dq2*dqr1*cos(2*q3)*sin(2*q2)*sin(2*q4)*sin(2*q5))/8 - (dq3*dqr1*cos(2*q2)*sin(2*q3)*sin(2*q4)*sin(2*q5))/8 + (dq3*dqr1*cos(2*q3)*sin(2*q2)*sin(2*q4)*sin(2*q5))/8 + (dq4*dqr1*cos(2*q4)*sin(2*q2)*sin(2*q3)*sin(2*q5))/8 + (5*dq4*dqr1*cos(2*q5)*sin(2*q2)*sin(2*q3)*sin(2*q4))/32 + (5*dq5*dqr1*cos(2*q4)*sin(2*q2)*sin(2*q3)*sin(2*q5))/32 + (dq5*dqr1*cos(2*q5)*sin(2*q2)*sin(2*q3)*sin(2*q4))/8 + (3^(1/2)*dq5*dqr2*sin(q2)*sin(q3)*sin(q4))/4 + (5*dq4*dqr2*cos(2*q4)*cos(2*q5)*cos(q2)*sin(q3))/16 - (5*dq4*dqr2*cos(2*q4)*cos(2*q5)*cos(q3)*sin(q2))/16 + (dq5*dqr2*cos(2*q4)*cos(2*q5)*cos(q2)*sin(q3))/4 - (dq5*dqr2*cos(2*q4)*cos(2*q5)*cos(q3)*sin(q2))/4 - (dq2*dqr2*cos(2*q4)*sin(2*q5)*sin(q2)*sin(q3))/4 - (5*dq2*dqr2*cos(2*q5)*sin(2*q4)*sin(q2)*sin(q3))/16 + (dq3*dqr2*cos(2*q4)*sin(2*q5)*sin(q2)*sin(q3))/4 + (5*dq3*dqr2*cos(2*q5)*sin(2*q4)*sin(q2)*sin(q3))/16 - (dq4*dqr2*sin(2*q4)*sin(2*q5)*cos(q2)*sin(q3))/4 + (dq4*dqr2*sin(2*q4)*sin(2*q5)*cos(q3)*sin(q2))/4 - (5*dq5*dqr2*sin(2*q4)*sin(2*q5)*cos(q2)*sin(q3))/16 + (5*dq5*dqr2*sin(2*q4)*sin(2*q5)*cos(q3)*sin(q2))/16 + (3^(1/2)*dq2*dqr1*cos(2*q2)*cos(2*q3)*sin(q4))/8 - (3^(1/2)*dq3*dqr1*cos(2*q2)*cos(2*q3)*sin(q4))/8 - (3^(1/2)*dq4*dqr1*cos(2*q2)*sin(2*q3)*cos(q4))/16 + (3^(1/2)*dq4*dqr1*cos(2*q3)*sin(2*q2)*cos(q4))/16 + (3^(1/2)*dq2*dqr1*sin(2*q2)*sin(2*q3)*sin(q4))/8 - (3^(1/2)*dq3*dqr1*sin(2*q2)*sin(2*q3)*sin(q4))/8 + (3^(1/2)*dq2*dqr1*cos(2*q2)*cos(2*q3)*cos(2*q5)*sin(q4))/8 + (3^(1/2)*dq2*dqr1*cos(2*q2)*cos(2*q3)*sin(2*q5)*cos(q4))/4 - (3^(1/2)*dq3*dqr1*cos(2*q2)*cos(2*q3)*cos(2*q5)*sin(q4))/8 - (3^(1/2)*dq3*dqr1*cos(2*q2)*cos(2*q3)*sin(2*q5)*cos(q4))/4 - (3^(1/2)*dq4*dqr1*cos(2*q2)*cos(2*q5)*sin(2*q3)*cos(q4))/16 + (3^(1/2)*dq4*dqr1*cos(2*q3)*cos(2*q5)*sin(2*q2)*cos(q4))/16 - (3^(1/2)*dq5*dqr1*cos(2*q2)*cos(2*q5)*sin(2*q3)*cos(q4))/4 + (3^(1/2)*dq5*dqr1*cos(2*q3)*cos(2*q5)*sin(2*q2)*cos(q4))/4 + (3^(1/2)*dq1*dqr2*cos(2*q5)*sin(2*q2)*sin(2*q3)*sin(q4))/8 + (3^(1/2)*dq2*dqr1*cos(2*q5)*sin(2*q2)*sin(2*q3)*sin(q4))/8 + (3^(1/2)*dq2*dqr1*sin(2*q2)*sin(2*q3)*sin(2*q5)*cos(q4))/4 - (3^(1/2)*dq3*dqr1*cos(2*q5)*sin(2*q2)*sin(2*q3)*sin(q4))/8 - (3^(1/2)*dq3*dqr1*sin(2*q2)*sin(2*q3)*sin(2*q5)*cos(q4))/4 + (3^(1/2)*dq4*dqr1*cos(2*q2)*sin(2*q3)*sin(2*q5)*sin(q4))/8 - (3^(1/2)*dq4*dqr1*cos(2*q3)*sin(2*q2)*sin(2*q5)*sin(q4))/8 + (3^(1/2)*dq5*dqr1*cos(2*q2)*sin(2*q3)*sin(2*q5)*sin(q4))/8 - (3^(1/2)*dq5*dqr1*cos(2*q3)*sin(2*q2)*sin(2*q5)*sin(q4))/8 + (3^(1/2)*dq2*dqr2*cos(2*q5)*cos(q2)*cos(q4)*sin(q3))/8 - (3^(1/2)*dq2*dqr2*cos(2*q5)*cos(q3)*cos(q4)*sin(q2))/8 - (3^(1/2)*dq3*dqr2*cos(2*q5)*cos(q2)*cos(q4)*sin(q3))/8 + (3^(1/2)*dq3*dqr2*cos(2*q5)*cos(q3)*cos(q4)*sin(q2))/8 - (3^(1/2)*dq5*dqr2*cos(2*q5)*cos(q2)*cos(q3)*sin(q4))/4 - (3^(1/2)*dq2*dqr2*sin(2*q5)*cos(q2)*sin(q3)*sin(q4))/4 + (3^(1/2)*dq2*dqr2*sin(2*q5)*cos(q3)*sin(q2)*sin(q4))/4 + (3^(1/2)*dq3*dqr2*sin(2*q5)*cos(q2)*sin(q3)*sin(q4))/4 - (3^(1/2)*dq3*dqr2*sin(2*q5)*cos(q3)*sin(q2)*sin(q4))/4 - (3^(1/2)*dq5*dqr2*cos(2*q5)*sin(q2)*sin(q3)*sin(q4))/4 - (3^(1/2)*dq5*dqr2*sin(2*q5)*cos(q4)*sin(q2)*sin(q3))/8;
Y1_19_2=(dq1*dqr2*cos(2*q3)*sin(2*q2))/32 - (dq1*dqr2*cos(2*q2)*sin(2*q3))/32 + (dq1*dqr3*cos(2*q2)*sin(2*q3))/32 - (dq1*dqr3*cos(2*q3)*sin(2*q2))/32 - (5*dq2*dqr4*cos(q3)*sin(q2))/16 - (5*dq4*dqr3*cos(q2)*sin(q3))/16 + (5*dq4*dqr3*cos(q3)*sin(q2))/16 - (dq5*dqr3*cos(q2)*sin(q3))/4 + (dq5*dqr3*cos(q3)*sin(q2))/4 + (3*dq2*dqr2*sin(2*q4)*cos(q2)*cos(q3))/16 - (3*dq2*dqr3*sin(2*q4)*cos(q2)*cos(q3))/16 - (3*dq3*dqr2*sin(2*q4)*cos(q2)*cos(q3))/16 + (3*dq2*dqr4*cos(2*q4)*cos(q3)*sin(q2))/16 + (3*dq3*dqr3*sin(2*q4)*cos(q2)*cos(q3))/16 + (3*dq2*dqr4*cos(2*q5)*cos(q3)*sin(q2))/16 - (3*dq3*dqr4*cos(2*q4)*cos(q3)*sin(q2))/16 + (3*dq4*dqr3*cos(2*q4)*cos(q2)*sin(q3))/16 - (3*dq4*dqr3*cos(2*q4)*cos(q3)*sin(q2))/16 - (3*dq3*dqr4*cos(2*q5)*cos(q3)*sin(q2))/16 + (3*dq4*dqr3*cos(2*q5)*cos(q2)*sin(q3))/16 - (3*dq4*dqr3*cos(2*q5)*cos(q3)*sin(q2))/16 - (3*dq2*dqr3*sin(2*q4)*sin(q2)*sin(q3))/16 + (3*dq3*dqr3*sin(2*q4)*sin(q2)*sin(q3))/16 + (3*dq5*dqr4*sin(2*q5)*sin(q2)*sin(q3))/8 + (3*dq1*dqr2*cos(2*q2)*cos(2*q4)*sin(2*q3))/32 - (3*dq1*dqr2*cos(2*q3)*cos(2*q4)*sin(2*q2))/32 - (9*dq1*dqr2*cos(2*q2)*cos(2*q5)*sin(2*q3))/32 + (9*dq1*dqr2*cos(2*q3)*cos(2*q5)*sin(2*q2))/32 - (3*dq1*dqr3*cos(2*q2)*cos(2*q4)*sin(2*q3))/32 + (3*dq1*dqr3*cos(2*q3)*cos(2*q4)*sin(2*q2))/32 + (9*dq1*dqr3*cos(2*q2)*cos(2*q5)*sin(2*q3))/32 - (9*dq1*dqr3*cos(2*q3)*cos(2*q5)*sin(2*q2))/32 - (5*dq1*dqr2*cos(2*q2)*cos(2*q4)*cos(2*q5)*sin(2*q3))/32 + (5*dq1*dqr2*cos(2*q3)*cos(2*q4)*cos(2*q5)*sin(2*q2))/32 + (5*dq1*dqr3*cos(2*q2)*cos(2*q4)*cos(2*q5)*sin(2*q3))/32 - (5*dq1*dqr3*cos(2*q3)*cos(2*q4)*cos(2*q5)*sin(2*q2))/32 - (3^(1/2)*dq2*dqr3*cos(q2)*cos(q4)*sin(q3))/8 + (3^(1/2)*dq2*dqr3*cos(q3)*cos(q4)*sin(q2))/8 + (3^(1/2)*dq3*dqr3*cos(q2)*cos(q4)*sin(q3))/8 - (3^(1/2)*dq3*dqr3*cos(q3)*cos(q4)*sin(q2))/8 + (3^(1/2)*dq4*dqr4*cos(q3)*cos(q4)*sin(q2))/8 - (3^(1/2)*dq5*dqr3*cos(q2)*cos(q3)*sin(q4))/4 + (3^(1/2)*dq5*dqr4*cos(q3)*cos(q4)*sin(q2))/4 + (dq1*dqr2*cos(2*q2)*sin(2*q3)*sin(2*q4)*sin(2*q5))/8 - (dq1*dqr2*cos(2*q3)*sin(2*q2)*sin(2*q4)*sin(2*q5))/8 - (dq1*dqr3*cos(2*q2)*sin(2*q3)*sin(2*q4)*sin(2*q5))/8 + (dq1*dqr3*cos(2*q3)*sin(2*q2)*sin(2*q4)*sin(2*q5))/8 - (3^(1/2)*dq5*dqr3*sin(q2)*sin(q3)*sin(q4))/4 - (dq2*dqr2*cos(2*q4)*sin(2*q5)*cos(q2)*cos(q3))/4 - (5*dq2*dqr2*cos(2*q5)*sin(2*q4)*cos(q2)*cos(q3))/16 + (dq2*dqr3*cos(2*q4)*sin(2*q5)*cos(q2)*cos(q3))/4 + (5*dq2*dqr3*cos(2*q5)*sin(2*q4)*cos(q2)*cos(q3))/16 + (dq3*dqr2*cos(2*q4)*sin(2*q5)*cos(q2)*cos(q3))/4 + (5*dq3*dqr2*cos(2*q5)*sin(2*q4)*cos(q2)*cos(q3))/16 - (5*dq2*dqr4*cos(2*q4)*cos(2*q5)*cos(q3)*sin(q2))/16 - (dq3*dqr3*cos(2*q4)*sin(2*q5)*cos(q2)*cos(q3))/4 - (5*dq3*dqr3*cos(2*q5)*sin(2*q4)*cos(q2)*cos(q3))/16 + (5*dq3*dqr4*cos(2*q4)*cos(2*q5)*cos(q3)*sin(q2))/16 - (5*dq4*dqr3*cos(2*q4)*cos(2*q5)*cos(q2)*sin(q3))/16 + (5*dq4*dqr3*cos(2*q4)*cos(2*q5)*cos(q3)*sin(q2))/16 - (dq5*dqr3*cos(2*q4)*cos(2*q5)*cos(q2)*sin(q3))/4 + (dq5*dqr3*cos(2*q4)*cos(2*q5)*cos(q3)*sin(q2))/4 + (dq2*dqr3*cos(2*q4)*sin(2*q5)*sin(q2)*sin(q3))/4 + (5*dq2*dqr3*cos(2*q5)*sin(2*q4)*sin(q2)*sin(q3))/16 + (dq2*dqr4*sin(2*q4)*sin(2*q5)*cos(q3)*sin(q2))/4 - (dq3*dqr3*cos(2*q4)*sin(2*q5)*sin(q2)*sin(q3))/4 - (5*dq3*dqr3*cos(2*q5)*sin(2*q4)*sin(q2)*sin(q3))/16 - (dq3*dqr4*sin(2*q4)*sin(2*q5)*cos(q3)*sin(q2))/4 + (dq4*dqr3*sin(2*q4)*sin(2*q5)*cos(q2)*sin(q3))/4 - (dq4*dqr3*sin(2*q4)*sin(2*q5)*cos(q3)*sin(q2))/4 + (5*dq5*dqr3*sin(2*q4)*sin(2*q5)*cos(q2)*sin(q3))/16 - (5*dq5*dqr3*sin(2*q4)*sin(2*q5)*cos(q3)*sin(q2))/16 + (3^(1/2)*dq1*dqr2*cos(2*q2)*cos(2*q3)*sin(q4))/8 - (3^(1/2)*dq1*dqr3*cos(2*q2)*cos(2*q3)*sin(q4))/8 + (3^(1/2)*dq1*dqr2*sin(2*q2)*sin(2*q3)*sin(q4))/8 - (3^(1/2)*dq1*dqr3*sin(2*q2)*sin(2*q3)*sin(q4))/8 + (3^(1/2)*dq1*dqr2*cos(2*q2)*cos(2*q3)*cos(2*q5)*sin(q4))/8 + (3^(1/2)*dq1*dqr2*cos(2*q2)*cos(2*q3)*sin(2*q5)*cos(q4))/4 - (3^(1/2)*dq1*dqr3*cos(2*q2)*cos(2*q3)*cos(2*q5)*sin(q4))/8 - (3^(1/2)*dq1*dqr3*cos(2*q2)*cos(2*q3)*sin(2*q5)*cos(q4))/4 + (3^(1/2)*dq1*dqr2*sin(2*q2)*sin(2*q3)*sin(2*q5)*cos(q4))/4 - (3^(1/2)*dq1*dqr3*cos(2*q5)*sin(2*q2)*sin(2*q3)*sin(q4))/8 - (3^(1/2)*dq1*dqr3*sin(2*q2)*sin(2*q3)*sin(2*q5)*cos(q4))/4 - (3^(1/2)*dq2*dqr3*cos(2*q5)*cos(q2)*cos(q4)*sin(q3))/8 + (3^(1/2)*dq2*dqr3*cos(2*q5)*cos(q3)*cos(q4)*sin(q2))/8 + (3^(1/2)*dq3*dqr3*cos(2*q5)*cos(q2)*cos(q4)*sin(q3))/8 - (3^(1/2)*dq3*dqr3*cos(2*q5)*cos(q3)*cos(q4)*sin(q2))/8 - (3^(1/2)*dq5*dqr2*sin(2*q5)*cos(q2)*cos(q3)*cos(q4))/8 + (3^(1/2)*dq4*dqr4*cos(2*q5)*cos(q3)*cos(q4)*sin(q2))/8 + (3^(1/2)*dq5*dqr3*cos(2*q5)*cos(q2)*cos(q3)*sin(q4))/4 + (3^(1/2)*dq5*dqr3*sin(2*q5)*cos(q2)*cos(q3)*cos(q4))/8 + (3^(1/2)*dq5*dqr4*cos(2*q5)*cos(q3)*cos(q4)*sin(q2))/4 + (3^(1/2)*dq2*dqr3*sin(2*q5)*cos(q2)*sin(q3)*sin(q4))/4 - (3^(1/2)*dq2*dqr3*sin(2*q5)*cos(q3)*sin(q2)*sin(q4))/4 - (3^(1/2)*dq3*dqr3*sin(2*q5)*cos(q2)*sin(q3)*sin(q4))/4 + (3^(1/2)*dq3*dqr3*sin(2*q5)*cos(q3)*sin(q2)*sin(q4))/4 - (3^(1/2)*dq4*dqr4*sin(2*q5)*cos(q3)*sin(q2)*sin(q4))/4 + (3^(1/2)*dq5*dqr3*cos(2*q5)*sin(q2)*sin(q3)*sin(q4))/4 + (3^(1/2)*dq5*dqr3*sin(2*q5)*cos(q4)*sin(q2)*sin(q3))/8 - (3^(1/2)*dq5*dqr4*sin(2*q5)*cos(q3)*sin(q2)*sin(q4))/8;
Y1_19_3=(3*dq1*dqr4*sin(2*q4))/32 + (3*dq1*dqr5*sin(2*q5))/32 + (5*ddqr4*sin(q2)*sin(q3))/8 + (ddqr5*sin(q2)*sin(q3))/2 - (dq1*dqr4*cos(2*q4)*sin(2*q5))/8 - (5*dq1*dqr4*cos(2*q5)*sin(2*q4))/32 - (5*dq1*dqr5*cos(2*q4)*sin(2*q5))/32 - (dq1*dqr5*cos(2*q5)*sin(2*q4))/8 + (3*ddqr2*sin(2*q4)*cos(q3)*sin(q2))/16 - (3*ddqr3*sin(2*q4)*cos(q3)*sin(q2))/16 - (3*ddqr4*cos(2*q5)*sin(q2)*sin(q3))/8 + (5*dq2*dqr4*cos(q2)*sin(q3))/16 + (dq2*dqr5*cos(q2)*sin(q3))/4 - (dq2*dqr5*cos(q3)*sin(q2))/4 - (5*dq3*dqr4*cos(q2)*sin(q3))/16 + (5*dq3*dqr4*cos(q3)*sin(q2))/16 - (dq3*dqr5*cos(q2)*sin(q3))/4 + (dq3*dqr5*cos(q3)*sin(q2))/4 - (3*dq2*dqr4*cos(2*q4)*cos(q2)*sin(q3))/16 - (3*dq2*dqr4*cos(2*q5)*cos(q2)*sin(q3))/16 + (3*dq3*dqr4*cos(2*q4)*cos(q2)*sin(q3))/16 + (3*dq3*dqr4*cos(2*q5)*cos(q2)*sin(q3))/16 + (3*dq4*dqr5*sin(2*q5)*cos(q2)*cos(q3))/8 + (3*dq5*dqr4*sin(2*q5)*cos(q2)*cos(q3))/8 + (3*dq4*dqr5*sin(2*q5)*sin(q2)*sin(q3))/8 + (3^(1/2)*ddqr2*cos(q4)*sin(q2)*sin(q3))/8 - (3^(1/2)*ddqr3*cos(q4)*sin(q2)*sin(q3))/8 - (3^(1/2)*ddqr4*cos(q2)*sin(q3)*sin(q4))/8 + (3^(1/2)*ddqr4*cos(q3)*sin(q2)*sin(q4))/8 - (3^(1/2)*ddqr5*cos(q2)*sin(q3)*sin(q4))/2 + (3^(1/2)*ddqr5*cos(q3)*sin(q2)*sin(q4))/2 - (3*dq1*dqr4*cos(2*q2)*cos(2*q3)*sin(2*q4))/32 + (9*dq1*dqr5*cos(2*q2)*cos(2*q3)*sin(2*q5))/32 - (3*dq1*dqr4*sin(2*q2)*sin(2*q3)*sin(2*q4))/32 + (9*dq1*dqr5*sin(2*q2)*sin(2*q3)*sin(2*q5))/32 - (ddqr2*cos(2*q4)*sin(2*q5)*cos(q3)*sin(q2))/4 - (5*ddqr2*cos(2*q5)*sin(2*q4)*cos(q3)*sin(q2))/16 + (ddqr3*cos(2*q4)*sin(2*q5)*cos(q3)*sin(q2))/4 + (5*ddqr3*cos(2*q5)*sin(2*q4)*cos(q3)*sin(q2))/16 + (dq1*dqr4*cos(2*q2)*cos(2*q3)*cos(2*q4)*sin(2*q5))/8 + (5*dq1*dqr4*cos(2*q2)*cos(2*q3)*cos(2*q5)*sin(2*q4))/32 + (5*dq1*dqr5*cos(2*q2)*cos(2*q3)*cos(2*q4)*sin(2*q5))/32 + (dq1*dqr5*cos(2*q2)*cos(2*q3)*cos(2*q5)*sin(2*q4))/8 - (3^(1/2)*ddqr2*sin(2*q5)*sin(q2)*sin(q3)*sin(q4))/4 + (3^(1/2)*ddqr3*sin(2*q5)*sin(q2)*sin(q3)*sin(q4))/4 + (3^(1/2)*dq2*dqr5*cos(q2)*cos(q3)*sin(q4))/4 - (3^(1/2)*dq3*dqr5*cos(q2)*cos(q3)*sin(q4))/4 - (3^(1/2)*dq4*dqr4*cos(q2)*cos(q4)*sin(q3))/8 - (3^(1/2)*dq4*dqr5*cos(q2)*cos(q4)*sin(q3))/4 + (3^(1/2)*dq4*dqr5*cos(q3)*cos(q4)*sin(q2))/4 - (3^(1/2)*dq5*dqr4*cos(q2)*cos(q4)*sin(q3))/4 + (dq1*dqr4*cos(2*q4)*sin(2*q2)*sin(2*q3)*sin(2*q5))/8 + (5*dq1*dqr4*cos(2*q5)*sin(2*q2)*sin(2*q3)*sin(2*q4))/32 + (5*dq1*dqr5*cos(2*q4)*sin(2*q2)*sin(2*q3)*sin(2*q5))/32 + (dq1*dqr5*cos(2*q5)*sin(2*q2)*sin(2*q3)*sin(2*q4))/8 + (3^(1/2)*dq2*dqr5*sin(q2)*sin(q3)*sin(q4))/4 - (3^(1/2)*dq3*dqr5*sin(q2)*sin(q3)*sin(q4))/4 + (5*dq2*dqr4*cos(2*q4)*cos(2*q5)*cos(q2)*sin(q3))/16 + (dq2*dqr5*cos(2*q4)*cos(2*q5)*cos(q2)*sin(q3))/4 - (dq2*dqr5*cos(2*q4)*cos(2*q5)*cos(q3)*sin(q2))/4 - (5*dq3*dqr4*cos(2*q4)*cos(2*q5)*cos(q2)*sin(q3))/16 - (dq3*dqr5*cos(2*q4)*cos(2*q5)*cos(q2)*sin(q3))/4 + (dq3*dqr5*cos(2*q4)*cos(2*q5)*cos(q3)*sin(q2))/4 - (dq2*dqr4*sin(2*q4)*sin(2*q5)*cos(q2)*sin(q3))/4 - (5*dq2*dqr5*sin(2*q4)*sin(2*q5)*cos(q2)*sin(q3))/16 + (5*dq2*dqr5*sin(2*q4)*sin(2*q5)*cos(q3)*sin(q2))/16 + (dq3*dqr4*sin(2*q4)*sin(2*q5)*cos(q2)*sin(q3))/4 + (5*dq3*dqr5*sin(2*q4)*sin(2*q5)*cos(q2)*sin(q3))/16 - (5*dq3*dqr5*sin(2*q4)*sin(2*q5)*cos(q3)*sin(q2))/16 - (3^(1/2)*dq1*dqr4*cos(2*q2)*sin(2*q3)*cos(q4))/16 + (3^(1/2)*dq1*dqr4*cos(2*q3)*sin(2*q2)*cos(q4))/16 + (3^(1/2)*ddqr2*cos(2*q5)*cos(q4)*sin(q2)*sin(q3))/8 - (3^(1/2)*ddqr3*cos(2*q5)*cos(q4)*sin(q2)*sin(q3))/8 - (3^(1/2)*ddqr4*cos(2*q5)*cos(q2)*sin(q3)*sin(q4))/8 + (3^(1/2)*ddqr4*cos(2*q5)*cos(q3)*sin(q2)*sin(q4))/8 + (3^(1/2)*ddqr4*sin(2*q5)*cos(q3)*cos(q4)*sin(q2))/4 - (3^(1/2)*dq1*dqr4*cos(2*q2)*cos(2*q5)*sin(2*q3)*cos(q4))/16 + (3^(1/2)*dq1*dqr4*cos(2*q3)*cos(2*q5)*sin(2*q2)*cos(q4))/16 - (3^(1/2)*dq1*dqr5*cos(2*q2)*cos(2*q5)*sin(2*q3)*cos(q4))/4 + (3^(1/2)*dq1*dqr5*cos(2*q3)*cos(2*q5)*sin(2*q2)*cos(q4))/4 + (3^(1/2)*dq1*dqr4*cos(2*q2)*sin(2*q3)*sin(2*q5)*sin(q4))/8 - (3^(1/2)*dq1*dqr4*cos(2*q3)*sin(2*q2)*sin(2*q5)*sin(q4))/8 + (3^(1/2)*dq1*dqr5*cos(2*q2)*sin(2*q3)*sin(2*q5)*sin(q4))/8 - (3^(1/2)*dq1*dqr5*cos(2*q3)*sin(2*q2)*sin(2*q5)*sin(q4))/8 - (3^(1/2)*dq2*dqr5*cos(2*q5)*cos(q2)*cos(q3)*sin(q4))/4 - (3^(1/2)*dq2*dqr5*sin(2*q5)*cos(q2)*cos(q3)*cos(q4))/8 + (3^(1/2)*dq3*dqr5*cos(2*q5)*cos(q2)*cos(q3)*sin(q4))/4 + (3^(1/2)*dq3*dqr5*sin(2*q5)*cos(q2)*cos(q3)*cos(q4))/8 - (3^(1/2)*dq4*dqr4*cos(2*q5)*cos(q2)*cos(q4)*sin(q3))/8 - (3^(1/2)*dq4*dqr5*cos(2*q5)*cos(q2)*cos(q4)*sin(q3))/4 + (3^(1/2)*dq4*dqr5*cos(2*q5)*cos(q3)*cos(q4)*sin(q2))/4 - (3^(1/2)*dq5*dqr4*cos(2*q5)*cos(q2)*cos(q4)*sin(q3))/4 - (3^(1/2)*dq2*dqr5*cos(2*q5)*sin(q2)*sin(q3)*sin(q4))/4 - (3^(1/2)*dq2*dqr5*sin(2*q5)*cos(q4)*sin(q2)*sin(q3))/8 + (3^(1/2)*dq3*dqr5*cos(2*q5)*sin(q2)*sin(q3)*sin(q4))/4 + (3^(1/2)*dq3*dqr5*sin(2*q5)*cos(q4)*sin(q2)*sin(q3))/8 + (3^(1/2)*dq4*dqr4*sin(2*q5)*cos(q2)*sin(q3)*sin(q4))/4 + (3^(1/2)*dq4*dqr5*sin(2*q5)*cos(q2)*sin(q3)*sin(q4))/8 - (3^(1/2)*dq4*dqr5*sin(2*q5)*cos(q3)*sin(q2)*sin(q4))/8 + (3^(1/2)*dq5*dqr4*sin(2*q5)*cos(q2)*sin(q3)*sin(q4))/8;
Y1_19_4=(21*ddqr1)/32 - (3*ddqr1*cos(2*q4))/32 - (3*ddqr1*cos(2*q5))/32 - (ddqr1*cos(2*q2)*cos(2*q3))/32 + (5*ddqr1*cos(2*q4)*cos(2*q5))/32 - (ddqr1*sin(2*q2)*sin(2*q3))/32 - (ddqr1*sin(2*q4)*sin(2*q5))/8 + (5*ddqr4*cos(q2)*cos(q3))/8 + (ddqr5*cos(q2)*cos(q3))/2 + (3*ddqr1*cos(2*q2)*cos(2*q3)*cos(2*q4))/32 - (9*ddqr1*cos(2*q2)*cos(2*q3)*cos(2*q5))/32 + (3*ddqr1*cos(2*q4)*sin(2*q2)*sin(2*q3))/32 - (9*ddqr1*cos(2*q5)*sin(2*q2)*sin(2*q3))/32 - (3*ddqr4*cos(2*q5)*cos(q2)*cos(q3))/8 - (3*ddqr2*sin(2*q4)*cos(q2)*sin(q3))/16 + (3*ddqr3*sin(2*q4)*cos(q2)*sin(q3))/16 - (3^(1/2)*ddqr1*cos(2*q2)*sin(2*q3)*sin(q4))/8 + (3^(1/2)*ddqr1*cos(2*q3)*sin(2*q2)*sin(q4))/8 - (5*ddqr1*cos(2*q2)*cos(2*q3)*cos(2*q4)*cos(2*q5))/32 + (3^(1/2)*ddqr2*cos(q2)*cos(q3)*cos(q4))/8 - (3^(1/2)*ddqr3*cos(q2)*cos(q3)*cos(q4))/8 + (ddqr1*cos(2*q2)*cos(2*q3)*sin(2*q4)*sin(2*q5))/8 - (5*ddqr1*cos(2*q4)*cos(2*q5)*sin(2*q2)*sin(2*q3))/32 + (ddqr1*sin(2*q2)*sin(2*q3)*sin(2*q4)*sin(2*q5))/8 + (ddqr2*cos(2*q4)*sin(2*q5)*cos(q2)*sin(q3))/4 + (5*ddqr2*cos(2*q5)*sin(2*q4)*cos(q2)*sin(q3))/16 - (ddqr3*cos(2*q4)*sin(2*q5)*cos(q2)*sin(q3))/4 - (5*ddqr3*cos(2*q5)*sin(2*q4)*cos(q2)*sin(q3))/16 - (3^(1/2)*ddqr1*cos(2*q2)*cos(2*q5)*sin(2*q3)*sin(q4))/8 - (3^(1/2)*ddqr1*cos(2*q2)*sin(2*q3)*sin(2*q5)*cos(q4))/4 + (3^(1/2)*ddqr1*cos(2*q3)*cos(2*q5)*sin(2*q2)*sin(q4))/8 + (3^(1/2)*ddqr1*cos(2*q3)*sin(2*q2)*sin(2*q5)*cos(q4))/4 + (3^(1/2)*ddqr2*cos(2*q5)*cos(q2)*cos(q3)*cos(q4))/8 - (3^(1/2)*ddqr3*cos(2*q5)*cos(q2)*cos(q3)*cos(q4))/8 - (3^(1/2)*ddqr2*sin(2*q5)*cos(q2)*cos(q3)*sin(q4))/4 + (3^(1/2)*ddqr3*sin(2*q5)*cos(q2)*cos(q3)*sin(q4))/4 - (3^(1/2)*ddqr4*sin(2*q5)*cos(q2)*cos(q4)*sin(q3))/4;
Y1_20_1=(3*dq2*dqr1*cos(2*q2)*sin(2*q3)*sin(2*q4)*sin(q5))/32 - (3*dq2*dqr1*cos(2*q3)*sin(2*q2)*sin(2*q4)*sin(q5))/32 - (3*dq3*dqr1*cos(2*q2)*sin(2*q3)*sin(2*q4)*sin(q5))/32 + (3*dq3*dqr1*cos(2*q3)*sin(2*q2)*sin(2*q4)*sin(q5))/32 - (9*dq2*dqr1*cos(2*q2)*sin(2*q3)*sin(2*q6)*sin(q5))/32 + (9*dq2*dqr1*cos(2*q3)*sin(2*q2)*sin(2*q6)*sin(q5))/32 + (3*dq4*dqr1*cos(2*q4)*sin(2*q2)*sin(2*q3)*sin(q5))/32 + (9*dq3*dqr1*cos(2*q2)*sin(2*q3)*sin(2*q6)*sin(q5))/32 - (9*dq3*dqr1*cos(2*q3)*sin(2*q2)*sin(2*q6)*sin(q5))/32 - (3^(1/2)*dq2*dqr1*cos(2*q2)*cos(2*q3)*sin(q4))/64 + (3^(1/2)*dq3*dqr1*cos(2*q2)*cos(2*q3)*sin(q4))/64 - (3^(1/2)*dq2*dqr1*sin(2*q2)*sin(2*q3)*sin(q4))/64 + (3^(1/2)*dq3*dqr1*sin(2*q2)*sin(2*q3)*sin(q4))/64 - (3*3^(1/2)*dq2*dqr1*cos(2*q2)*cos(2*q3)*cos(2*q5)*sin(q4))/64 - (9*3^(1/2)*dq2*dqr1*cos(2*q2)*cos(2*q3)*cos(2*q6)*sin(q4))/64 + (3*3^(1/2)*dq3*dqr1*cos(2*q2)*cos(2*q3)*cos(2*q5)*sin(q4))/64 + (9*3^(1/2)*dq3*dqr1*cos(2*q2)*cos(2*q3)*cos(2*q6)*sin(q4))/64 - (3*dq4*dqr1*sin(2*q2)*sin(2*q3)*sin(2*q4)*sin(2*q6)*sin(q5))/32 - (3*3^(1/2)*dq2*dqr1*cos(2*q5)*sin(2*q2)*sin(2*q3)*sin(q4))/64 - (9*3^(1/2)*dq2*dqr1*cos(2*q6)*sin(2*q2)*sin(2*q3)*sin(q4))/64 + (3*3^(1/2)*dq3*dqr1*cos(2*q5)*sin(2*q2)*sin(2*q3)*sin(q4))/64 + (9*3^(1/2)*dq3*dqr1*cos(2*q6)*sin(2*q2)*sin(2*q3)*sin(q4))/64 - (3*3^(1/2)*dq4*dqr1*cos(2*q2)*sin(2*q3)*sin(2*q5)*sin(q4))/64 + (3*3^(1/2)*dq4*dqr1*cos(2*q3)*sin(2*q2)*sin(2*q5)*sin(q4))/64 - (3*3^(1/2)*dq5*dqr1*cos(2*q2)*sin(2*q3)*sin(2*q5)*sin(q4))/64 + (3*3^(1/2)*dq5*dqr1*cos(2*q3)*sin(2*q2)*sin(2*q5)*sin(q4))/64 - (9*3^(1/2)*dq6*dqr1*cos(2*q2)*sin(2*q3)*sin(2*q6)*sin(q4))/64 + (9*3^(1/2)*dq6*dqr1*cos(2*q3)*sin(2*q2)*sin(2*q6)*sin(q4))/64 - (3^(1/2)*dq2*dqr1*cos(2*q2)*cos(2*q3)*cos(q4)*sin(q5))/16 + (3^(1/2)*dq2*dqr1*cos(2*q2)*cos(2*q3)*cos(q5)*sin(q4))/16 + (3^(1/2)*dq3*dqr1*cos(2*q2)*cos(2*q3)*cos(q4)*sin(q5))/16 - (3^(1/2)*dq3*dqr1*cos(2*q2)*cos(2*q3)*cos(q5)*sin(q4))/16 - (3^(1/2)*dq2*dqr1*sin(2*q2)*sin(2*q3)*cos(q4)*sin(q5))/16 + (3^(1/2)*dq2*dqr1*sin(2*q2)*sin(2*q3)*cos(q5)*sin(q4))/16 + (3^(1/2)*dq3*dqr1*sin(2*q2)*sin(2*q3)*cos(q4)*sin(q5))/16 - (3^(1/2)*dq3*dqr1*sin(2*q2)*sin(2*q3)*cos(q5)*sin(q4))/16 - (3^(1/2)*dq4*dqr1*cos(2*q2)*sin(2*q3)*sin(q4)*sin(q5))/32 + (3^(1/2)*dq4*dqr1*cos(2*q3)*sin(2*q2)*sin(q4)*sin(q5))/32 + (3^(1/2)*dq5*dqr1*cos(2*q2)*sin(2*q3)*sin(q4)*sin(q5))/32 - (3^(1/2)*dq5*dqr1*cos(2*q3)*sin(2*q2)*sin(q4)*sin(q5))/32 + (3*dq2*dqr1*cos(2*q2)*cos(2*q4)*sin(2*q3)*sin(2*q6)*sin(q5))/32 + (3*dq2*dqr1*cos(2*q2)*cos(2*q6)*sin(2*q3)*sin(2*q4)*sin(q5))/32 - (3*dq2*dqr1*cos(2*q3)*cos(2*q4)*sin(2*q2)*sin(2*q6)*sin(q5))/32 - (3*dq2*dqr1*cos(2*q3)*cos(2*q6)*sin(2*q2)*sin(2*q4)*sin(q5))/32 - (3*dq3*dqr1*cos(2*q2)*cos(2*q4)*sin(2*q3)*sin(2*q6)*sin(q5))/32 - (3*dq3*dqr1*cos(2*q2)*cos(2*q6)*sin(2*q3)*sin(2*q4)*sin(q5))/32 + (3*dq3*dqr1*cos(2*q3)*cos(2*q4)*sin(2*q2)*sin(2*q6)*sin(q5))/32 + (3*dq3*dqr1*cos(2*q3)*cos(2*q6)*sin(2*q2)*sin(2*q4)*sin(q5))/32 - (3*dq4*dqr1*cos(2*q2)*cos(2*q3)*sin(2*q4)*sin(2*q6)*sin(q5))/32 + (3*dq4*dqr1*cos(2*q4)*cos(2*q6)*sin(2*q2)*sin(2*q3)*sin(q5))/32 - (3^(1/2)*dq2*dqr1*sin(2*q2)*sin(2*q3)*sin(2*q6)*sin(q4)*sin(q5))/8 + (3^(1/2)*dq3*dqr1*sin(2*q2)*sin(2*q3)*sin(2*q6)*sin(q4)*sin(q5))/8 + (5*3^(1/2)*dq2*dqr1*cos(2*q2)*cos(2*q3)*cos(2*q5)*cos(2*q6)*sin(q4))/64 - (5*3^(1/2)*dq3*dqr1*cos(2*q2)*cos(2*q3)*cos(2*q5)*cos(2*q6)*sin(q4))/64 - (3^(1/2)*dq2*dqr1*cos(2*q2)*cos(2*q3)*sin(2*q5)*sin(2*q6)*sin(q4))/16 + (5*3^(1/2)*dq2*dqr1*cos(2*q5)*cos(2*q6)*sin(2*q2)*sin(2*q3)*sin(q4))/64 + (3^(1/2)*dq3*dqr1*cos(2*q2)*cos(2*q3)*sin(2*q5)*sin(2*q6)*sin(q4))/16 - (5*3^(1/2)*dq3*dqr1*cos(2*q5)*cos(2*q6)*sin(2*q2)*sin(2*q3)*sin(q4))/64 + (3^(1/2)*dq4*dqr1*cos(2*q2)*cos(2*q5)*sin(2*q3)*sin(2*q6)*sin(q4))/16 + (5*3^(1/2)*dq4*dqr1*cos(2*q2)*cos(2*q6)*sin(2*q3)*sin(2*q5)*sin(q4))/64 - (3^(1/2)*dq4*dqr1*cos(2*q3)*cos(2*q5)*sin(2*q2)*sin(2*q6)*sin(q4))/16 - (5*3^(1/2)*dq4*dqr1*cos(2*q3)*cos(2*q6)*sin(2*q2)*sin(2*q5)*sin(q4))/64 + (3^(1/2)*dq5*dqr1*cos(2*q2)*cos(2*q5)*sin(2*q3)*sin(2*q6)*sin(q4))/16 + (5*3^(1/2)*dq5*dqr1*cos(2*q2)*cos(2*q6)*sin(2*q3)*sin(2*q5)*sin(q4))/64 - (3^(1/2)*dq5*dqr1*cos(2*q3)*cos(2*q5)*sin(2*q2)*sin(2*q6)*sin(q4))/16 - (5*3^(1/2)*dq5*dqr1*cos(2*q3)*cos(2*q6)*sin(2*q2)*sin(2*q5)*sin(q4))/64 + (5*3^(1/2)*dq6*dqr1*cos(2*q2)*cos(2*q5)*sin(2*q3)*sin(2*q6)*sin(q4))/64 + (3^(1/2)*dq6*dqr1*cos(2*q2)*cos(2*q6)*sin(2*q3)*sin(2*q5)*sin(q4))/16 - (5*3^(1/2)*dq6*dqr1*cos(2*q3)*cos(2*q5)*sin(2*q2)*sin(2*q6)*sin(q4))/64 - (3^(1/2)*dq6*dqr1*cos(2*q3)*cos(2*q6)*sin(2*q2)*sin(2*q5)*sin(q4))/16 - (3^(1/2)*dq2*dqr1*sin(2*q2)*sin(2*q3)*sin(2*q5)*sin(2*q6)*sin(q4))/16 + (3^(1/2)*dq3*dqr1*sin(2*q2)*sin(2*q3)*sin(2*q5)*sin(2*q6)*sin(q4))/16 - (3^(1/2)*dq2*dqr1*cos(2*q2)*cos(2*q3)*cos(2*q6)*cos(q4)*sin(q5))/16 + (3^(1/2)*dq2*dqr1*cos(2*q2)*cos(2*q3)*cos(2*q6)*cos(q5)*sin(q4))/16 + (3^(1/2)*dq3*dqr1*cos(2*q2)*cos(2*q3)*cos(2*q6)*cos(q4)*sin(q5))/16 - (3^(1/2)*dq3*dqr1*cos(2*q2)*cos(2*q3)*cos(2*q6)*cos(q5)*sin(q4))/16 - (3^(1/2)*dq2*dqr1*cos(2*q2)*cos(2*q3)*sin(2*q6)*sin(q4)*sin(q5))/8 - (3^(1/2)*dq2*dqr1*cos(2*q6)*sin(2*q2)*sin(2*q3)*cos(q4)*sin(q5))/16 + (3^(1/2)*dq2*dqr1*cos(2*q6)*sin(2*q2)*sin(2*q3)*cos(q5)*sin(q4))/16 + (3^(1/2)*dq3*dqr1*cos(2*q2)*cos(2*q3)*sin(2*q6)*sin(q4)*sin(q5))/8 + (3^(1/2)*dq3*dqr1*cos(2*q6)*sin(2*q2)*sin(2*q3)*cos(q4)*sin(q5))/16 - (3^(1/2)*dq3*dqr1*cos(2*q6)*sin(2*q2)*sin(2*q3)*cos(q5)*sin(q4))/16 - (3^(1/2)*dq4*dqr1*cos(2*q2)*cos(2*q6)*sin(2*q3)*sin(q4)*sin(q5))/32 + (3^(1/2)*dq4*dqr1*cos(2*q2)*sin(2*q3)*sin(2*q6)*cos(q4)*sin(q5))/16 - (3^(1/2)*dq4*dqr1*cos(2*q2)*sin(2*q3)*sin(2*q6)*cos(q5)*sin(q4))/16 + (3^(1/2)*dq4*dqr1*cos(2*q3)*cos(2*q6)*sin(2*q2)*sin(q4)*sin(q5))/32 - (3^(1/2)*dq4*dqr1*cos(2*q3)*sin(2*q2)*sin(2*q6)*cos(q4)*sin(q5))/16 + (3^(1/2)*dq4*dqr1*cos(2*q3)*sin(2*q2)*sin(2*q6)*cos(q5)*sin(q4))/16 + (3^(1/2)*dq5*dqr1*cos(2*q2)*cos(2*q6)*sin(2*q3)*sin(q4)*sin(q5))/32 - (3^(1/2)*dq5*dqr1*cos(2*q2)*sin(2*q3)*sin(2*q6)*cos(q4)*sin(q5))/16 + (3^(1/2)*dq5*dqr1*cos(2*q2)*sin(2*q3)*sin(2*q6)*cos(q5)*sin(q4))/16 - (3^(1/2)*dq5*dqr1*cos(2*q3)*cos(2*q6)*sin(2*q2)*sin(q4)*sin(q5))/32 + (3^(1/2)*dq5*dqr1*cos(2*q3)*sin(2*q2)*sin(2*q6)*cos(q4)*sin(q5))/16 - (3^(1/2)*dq5*dqr1*cos(2*q3)*sin(2*q2)*sin(2*q6)*cos(q5)*sin(q4))/16 + (3^(1/2)*dq6*dqr1*cos(2*q2)*cos(2*q6)*sin(2*q3)*sin(q4)*sin(q5))/8 - (3^(1/2)*dq6*dqr1*cos(2*q2)*sin(2*q3)*sin(2*q6)*cos(q4)*sin(q5))/16 + (3^(1/2)*dq6*dqr1*cos(2*q2)*sin(2*q3)*sin(2*q6)*cos(q5)*sin(q4))/16 - (3^(1/2)*dq6*dqr1*cos(2*q3)*cos(2*q6)*sin(2*q2)*sin(q4)*sin(q5))/8 + (3^(1/2)*dq6*dqr1*cos(2*q3)*sin(2*q2)*sin(2*q6)*cos(q4)*sin(q5))/16 - (3^(1/2)*dq6*dqr1*cos(2*q3)*sin(2*q2)*sin(2*q6)*cos(q5)*sin(q4))/16;
Y1_20_2=(9*dq2*dqr1*cos(2*q2)*sin(2*q3)*cos(q5))/64 - (3*dq4*dqr1*cos(2*q4)*sin(q5))/32 - (3*dq5*dqr1*cos(2*q4)*sin(q5))/128 - (3*dq5*dqr1*cos(2*q6)*sin(q5))/128 - (3*dq6*dqr1*cos(2*q6)*sin(q5))/32 - (3*dq5*dqr1*sin(q5))/128 - (9*dq2*dqr1*cos(2*q3)*sin(2*q2)*cos(q5))/64 - (9*dq3*dqr1*cos(2*q2)*sin(2*q3)*cos(q5))/64 + (9*dq3*dqr1*cos(2*q3)*sin(2*q2)*cos(q5))/64 - (9*dq5*dqr1*cos(2*q2)*cos(2*q3)*sin(q5))/128 - (3*dq4*dqr1*cos(2*q4)*cos(2*q6)*sin(q5))/32 - (3*dq5*dqr1*cos(2*q4)*cos(2*q6)*sin(q5))/128 - (3*dq6*dqr1*cos(2*q4)*cos(2*q6)*sin(q5))/32 - (9*dq5*dqr1*sin(2*q2)*sin(2*q3)*sin(q5))/128 + (3*dq4*dqr1*sin(2*q4)*sin(2*q6)*sin(q5))/32 + (3*dq5*dqr1*sin(2*q4)*sin(2*q6)*sin(q5))/32 + (3*dq6*dqr1*sin(2*q4)*sin(2*q6)*sin(q5))/32 - (3*dq2*dqr1*cos(2*q2)*cos(2*q4)*sin(2*q3)*cos(q5))/64 + (3*dq2*dqr1*cos(2*q3)*cos(2*q4)*sin(2*q2)*cos(q5))/64 + (3*dq3*dqr1*cos(2*q2)*cos(2*q4)*sin(2*q3)*cos(q5))/64 - (3*dq3*dqr1*cos(2*q3)*cos(2*q4)*sin(2*q2)*cos(q5))/64 + (9*dq2*dqr1*cos(2*q2)*cos(2*q6)*sin(2*q3)*cos(q5))/64 - (9*dq2*dqr1*cos(2*q3)*cos(2*q6)*sin(2*q2)*cos(q5))/64 + (3*dq4*dqr1*cos(2*q2)*cos(2*q3)*cos(2*q4)*sin(q5))/32 + (3*dq4*dqr1*cos(2*q2)*cos(2*q3)*sin(2*q4)*cos(q5))/64 - (9*dq3*dqr1*cos(2*q2)*cos(2*q6)*sin(2*q3)*cos(q5))/64 + (9*dq3*dqr1*cos(2*q3)*cos(2*q6)*sin(2*q2)*cos(q5))/64 + (3*dq5*dqr1*cos(2*q2)*cos(2*q3)*cos(2*q4)*sin(q5))/128 - (9*dq5*dqr1*cos(2*q2)*cos(2*q3)*cos(2*q6)*sin(q5))/128 - (9*dq6*dqr1*cos(2*q2)*cos(2*q3)*cos(2*q6)*sin(q5))/32 + (3*dq4*dqr1*sin(2*q2)*sin(2*q3)*sin(2*q4)*cos(q5))/64 + (3*dq5*dqr1*cos(2*q4)*sin(2*q2)*sin(2*q3)*sin(q5))/128 - (9*dq5*dqr1*cos(2*q6)*sin(2*q2)*sin(2*q3)*sin(q5))/128 - (9*dq6*dqr1*cos(2*q6)*sin(2*q2)*sin(2*q3)*sin(q5))/32 + (3^(1/2)*dq4*dqr1*cos(2*q2)*sin(2*q3)*cos(q4))/128 - (3^(1/2)*dq4*dqr1*cos(2*q3)*sin(2*q2)*cos(q4))/128 - (3*3^(1/2)*dq2*dqr1*cos(2*q2)*cos(2*q3)*sin(2*q5)*cos(q4))/32 + (3*3^(1/2)*dq3*dqr1*cos(2*q2)*cos(2*q3)*sin(2*q5)*cos(q4))/32 + (3*3^(1/2)*dq4*dqr1*cos(2*q2)*cos(2*q5)*sin(2*q3)*cos(q4))/128 - (3*3^(1/2)*dq4*dqr1*cos(2*q3)*cos(2*q5)*sin(2*q2)*cos(q4))/128 + (9*3^(1/2)*dq4*dqr1*cos(2*q2)*cos(2*q6)*sin(2*q3)*cos(q4))/128 - (9*3^(1/2)*dq4*dqr1*cos(2*q3)*cos(2*q6)*sin(2*q2)*cos(q4))/128 + (3*3^(1/2)*dq5*dqr1*cos(2*q2)*cos(2*q5)*sin(2*q3)*cos(q4))/32 - (3*3^(1/2)*dq5*dqr1*cos(2*q3)*cos(2*q5)*sin(2*q2)*cos(q4))/32 - (3*dq5*dqr1*sin(2*q2)*sin(2*q3)*sin(2*q4)*sin(2*q6)*sin(q5))/32 - (3*dq6*dqr1*sin(2*q2)*sin(2*q3)*sin(2*q4)*sin(2*q6)*sin(q5))/32 - (3*3^(1/2)*dq2*dqr1*sin(2*q2)*sin(2*q3)*sin(2*q5)*cos(q4))/32 + (3*3^(1/2)*dq3*dqr1*sin(2*q2)*sin(2*q3)*sin(2*q5)*cos(q4))/32 - (3^(1/2)*dq4*dqr1*cos(2*q2)*sin(2*q3)*cos(q4)*cos(q5))/32 + (3^(1/2)*dq4*dqr1*cos(2*q3)*sin(2*q2)*cos(q4)*cos(q5))/32 + (3^(1/2)*dq5*dqr1*cos(2*q2)*sin(2*q3)*cos(q4)*cos(q5))/32 - (3^(1/2)*dq5*dqr1*cos(2*q3)*sin(2*q2)*cos(q4)*cos(q5))/32 - (3*dq2*dqr1*cos(2*q2)*cos(2*q4)*cos(2*q6)*sin(2*q3)*cos(q5))/64 + (3*dq2*dqr1*cos(2*q3)*cos(2*q4)*cos(2*q6)*sin(2*q2)*cos(q5))/64 + (3*dq3*dqr1*cos(2*q2)*cos(2*q4)*cos(2*q6)*sin(2*q3)*cos(q5))/64 - (3*dq3*dqr1*cos(2*q3)*cos(2*q4)*cos(2*q6)*sin(2*q2)*cos(q5))/64 + (3*dq4*dqr1*cos(2*q2)*cos(2*q3)*cos(2*q4)*cos(2*q6)*sin(q5))/32 + (3*dq4*dqr1*cos(2*q2)*cos(2*q3)*cos(2*q6)*sin(2*q4)*cos(q5))/64 + (3*dq5*dqr1*cos(2*q2)*cos(2*q3)*cos(2*q4)*cos(2*q6)*sin(q5))/128 + (3*dq6*dqr1*cos(2*q2)*cos(2*q3)*cos(2*q4)*cos(2*q6)*sin(q5))/32 + (3*dq2*dqr1*cos(2*q2)*sin(2*q3)*sin(2*q4)*sin(2*q6)*cos(q5))/16 - (3*dq2*dqr1*cos(2*q3)*sin(2*q2)*sin(2*q4)*sin(2*q6)*cos(q5))/16 - (3*dq3*dqr1*cos(2*q2)*sin(2*q3)*sin(2*q4)*sin(2*q6)*cos(q5))/16 + (3*dq3*dqr1*cos(2*q3)*sin(2*q2)*sin(2*q4)*sin(2*q6)*cos(q5))/16 + (3*dq4*dqr1*cos(2*q4)*sin(2*q2)*sin(2*q3)*sin(2*q6)*cos(q5))/16 + (3*dq4*dqr1*cos(2*q6)*sin(2*q2)*sin(2*q3)*sin(2*q4)*cos(q5))/64 - (3*dq5*dqr1*cos(2*q2)*cos(2*q3)*sin(2*q4)*sin(2*q6)*sin(q5))/32 + (3*dq5*dqr1*cos(2*q4)*cos(2*q6)*sin(2*q2)*sin(2*q3)*sin(q5))/128 - (3*dq6*dqr1*cos(2*q2)*cos(2*q3)*sin(2*q4)*sin(2*q6)*sin(q5))/32 + (3*dq6*dqr1*cos(2*q4)*cos(2*q6)*sin(2*q2)*sin(2*q3)*sin(q5))/32 + (3^(1/2)*dq2*dqr1*cos(2*q2)*cos(2*q3)*cos(2*q5)*sin(2*q6)*cos(q4))/8 + (5*3^(1/2)*dq2*dqr1*cos(2*q2)*cos(2*q3)*cos(2*q6)*sin(2*q5)*cos(q4))/32 - (3^(1/2)*dq3*dqr1*cos(2*q2)*cos(2*q3)*cos(2*q5)*sin(2*q6)*cos(q4))/8 - (5*3^(1/2)*dq3*dqr1*cos(2*q2)*cos(2*q3)*cos(2*q6)*sin(2*q5)*cos(q4))/32 - (5*3^(1/2)*dq4*dqr1*cos(2*q2)*cos(2*q5)*cos(2*q6)*sin(2*q3)*cos(q4))/128 + (5*3^(1/2)*dq4*dqr1*cos(2*q3)*cos(2*q5)*cos(2*q6)*sin(2*q2)*cos(q4))/128 - (5*3^(1/2)*dq5*dqr1*cos(2*q2)*cos(2*q5)*cos(2*q6)*sin(2*q3)*cos(q4))/32 + (5*3^(1/2)*dq5*dqr1*cos(2*q3)*cos(2*q5)*cos(2*q6)*sin(2*q2)*cos(q4))/32 - (3^(1/2)*dq6*dqr1*cos(2*q2)*cos(2*q5)*cos(2*q6)*sin(2*q3)*cos(q4))/8 + (3^(1/2)*dq6*dqr1*cos(2*q3)*cos(2*q5)*cos(2*q6)*sin(2*q2)*cos(q4))/8 + (3^(1/2)*dq2*dqr1*cos(2*q5)*sin(2*q2)*sin(2*q3)*sin(2*q6)*cos(q4))/8 + (5*3^(1/2)*dq2*dqr1*cos(2*q6)*sin(2*q2)*sin(2*q3)*sin(2*q5)*cos(q4))/32 - (3^(1/2)*dq3*dqr1*cos(2*q5)*sin(2*q2)*sin(2*q3)*sin(2*q6)*cos(q4))/8 - (5*3^(1/2)*dq3*dqr1*cos(2*q6)*sin(2*q2)*sin(2*q3)*sin(2*q5)*cos(q4))/32 + (3^(1/2)*dq4*dqr1*cos(2*q2)*sin(2*q3)*sin(2*q5)*sin(2*q6)*cos(q4))/32 - (3^(1/2)*dq4*dqr1*cos(2*q3)*sin(2*q2)*sin(2*q5)*sin(2*q6)*cos(q4))/32 + (3^(1/2)*dq5*dqr1*cos(2*q2)*sin(2*q3)*sin(2*q5)*sin(2*q6)*cos(q4))/8 - (3^(1/2)*dq5*dqr1*cos(2*q3)*sin(2*q2)*sin(2*q5)*sin(2*q6)*cos(q4))/8 + (5*3^(1/2)*dq6*dqr1*cos(2*q2)*sin(2*q3)*sin(2*q5)*sin(2*q6)*cos(q4))/32 - (5*3^(1/2)*dq6*dqr1*cos(2*q3)*sin(2*q2)*sin(2*q5)*sin(2*q6)*cos(q4))/32 - (3^(1/2)*dq2*dqr1*cos(2*q2)*cos(2*q3)*sin(2*q6)*cos(q4)*cos(q5))/8 + (3^(1/2)*dq3*dqr1*cos(2*q2)*cos(2*q3)*sin(2*q6)*cos(q4)*cos(q5))/8 - (3^(1/2)*dq4*dqr1*cos(2*q2)*cos(2*q6)*sin(2*q3)*cos(q4)*cos(q5))/32 + (3^(1/2)*dq4*dqr1*cos(2*q3)*cos(2*q6)*sin(2*q2)*cos(q4)*cos(q5))/32 + (3^(1/2)*dq5*dqr1*cos(2*q2)*cos(2*q6)*sin(2*q3)*cos(q4)*cos(q5))/32 - (3^(1/2)*dq5*dqr1*cos(2*q3)*cos(2*q6)*sin(2*q2)*cos(q4)*cos(q5))/32 + (3^(1/2)*dq6*dqr1*cos(2*q2)*cos(2*q6)*sin(2*q3)*cos(q4)*cos(q5))/8 - (3^(1/2)*dq6*dqr1*cos(2*q3)*cos(2*q6)*sin(2*q2)*cos(q4)*cos(q5))/8 - (3^(1/2)*dq2*dqr1*sin(2*q2)*sin(2*q3)*sin(2*q6)*cos(q4)*cos(q5))/8 + (3^(1/2)*dq3*dqr1*sin(2*q2)*sin(2*q3)*sin(2*q6)*cos(q4)*cos(q5))/8;
